simulink model "PD_trajectory"  (R2020b)
settings: Solver=VariableStepAuto  StartTime=0.0  StopTime=10  RelTol=1e-3
libraries: pid_lib x6
(part 2 of 3)

== matlab function PD_trajectory/plant/MATLAB Function1 ==
  data: Theta input size=6; V output size=6; Thetad input size=6
function V = NumV(Theta,Thetad)
t1=Theta(1);
t2=Theta(2);
t3=Theta(3);
t4=Theta(4);
t5=Theta(5);
t6=Theta(6);
td1=Thetad(1);
td2=Thetad(2);
td3=Thetad(3);
td4=Thetad(4);
td5=Thetad(5);
td6=Thetad(6);

L1=0.1025;
L2=0.408;
L3=0.376;
L4=0.1025; 
L5=0.1025;

V=[td2*(td1*(25109.9375*sin(2.0*t2 + 2.0*t3 + 2.0*t4) + 1339251.84*sin(2.0*t2 + t3) + 184221.2*sin(2.0*t2 + 2.0*t3 + t4) + 1047890.8266888983333333366584905*sin(2.0*t2) + 199899.6*sin(2.0*t2 + t3 + t4) + 617106.24*sin(2.0*t2 + 2.0*t3) - 0.149375*L3^2*sin(2.0*t2 + 2.0*t3 + 2.0*t4) + 1.195*L4^2*sin(2.0*t2 + 2.0*t3 + 2.0*t4) - 898.64*L4*sin(2.0*t2 +2.0*t3 + t4) + 0.0746875*L3^2*sin(2.0*t2 + 2.0*t3 + 2.0*t4 - 2.0*t5) + 0.0746875*L3^2*sin(2.0*t2 + 2.0*t3 + 2.0*t4 + 2.0*t5) + 224.66*L3*sin(2.0*t2 + 2.0*t3 + t4 - 1.0*t5) -61.24375*L3*sin(2.0*t2 + 2.0*t3 + 2.0*t4 + t5) - 975.12*L4*sin(2.0*t2 + t3 + t4) + 243.78*L3*sin(2.0*t2 + t3 + t4 - 1.0*t5) - 224.66*L3*sin(2.0*t2 + 2.0*t3 + t4 + t5) +0.94625*L2^2*sin(2.0*t2) - 244.975*L4*sin(2.0*t2 + 2.0*t3 + 2.0*t4) + 61.24375*L3*sin(2.0*t2 + 2.0*t3 + 2.0*t4 - 1.0*t5) - 243.78*L3*sin(2.0*t2 + t3 + t4 + t5) -0.5975*L3*L4*sin(2.0*t2 + 2.0*t3 + 2.0*t4 - 1.0*t5) + 0.5975*L3*L4*sin(2.0*t2 + 2.0*t3 + 2.0*t4 + t5)) - 1.0*td5*(0.00036659114583333335217474324707609*sin(3.0*t2 -1.0*t1 + t3 + t4) + 0.00073318229166666670434948649415219*sin(t2 - 2.0*t1 + 3.0*t3 + t4) + 0.00018329557291666667608737162353805*sin(3.0*t2 - 2.0*t1 + t3 + t4) +0.00018329557291666667608737162353805*sin(2.0*t1 + 3.0*t2 + t3 + t4) + 0.00073318229166666670434948649415219*sin(t2 + t3 + t4) + 0.00036659114583333335217474324707609*sin(t1 - 1.0*t2 + t3 + t4) -0.00057664973958333336527190549070099*sin(t2 - 2.0*t1 + t3 + t4) - 0.00057664973958333336527190549070099*sin(2.0*t1 + t2 + t3 + t4) + 0.00036659114583333335217474324707609*sin(t1 + 3.0*t2 + t3 + t4) -0.00018329557291666667608737162353805*sin(2.0*t1 + t2 - 1.0*t3 - 1.0*t4) + 0.00036659114583333335217474324707609*sin(t3 - 1.0*t2 + t4) - 0.00036659114583333335217474324707609*sin(t1 + t2 - 1.0*t3 - 1.0*t4) +0.00073318229166666670434948649415219*sin(2.0*t1 + t2 - 1.0*t3 + t4) + 0.00018329557291666667608737162353805*sin(2.0*t1 - 1.0*t2 + t3 + t4) - 0.0010997734375000000565242297412283*sin(3.0*t2 + t3 + t4) -243.78*L3*sin(t2 - 1.0*t5) + 0.29875*L3^2*sin(t2 + t3 + t4) - 0.149375*L3^2*sin(t2 + t3 + t4 - 2.0*t5) - 0.149375*L3^2*sin(t2 + t3 + t4 + 2.0*t5) + 61.24375*L3*sin(t2 + t3 + t4 + t5) + 243.78*L3*sin(t2 + t5) -224.66*L3*sin(t2 + t3 - 1.0*t5) + 224.66*L3*sin(t2 + t3 + t5) - 61.24375*L3*sin(t2 + t3 + t4 - 1.0*t5) + 0.5975*L3*L4*sin(t2 + t3 + t4 - 1.0*t5) - 0.5975*L3*L4*sin(t2 + t3 + t4 + t5)) -1.0*td6*(0.00084023437500000005238864897449957*cos(t1)*cos(t5)*sin(t1) + 0.00042011718750000002619432448724979*cos(t1)^2*cos(t2)*cos(t3)*cos(t4)*sin(t5) - 0.00042011718750000002619432448724979*cos(t2)*cos(t3)*cos(t4)*sin(t1)^2*sin(t5) -0.00042011718750000002619432448724979*cos(t1)^2*cos(t2)*sin(t3)*sin(t4)*sin(t5) - 0.00042011718750000002619432448724979*cos(t1)^2*cos(t3)*sin(t2)*sin(t4)*sin(t5) - 0.00042011718750000002619432448724979*cos(t1)^2*cos(t4)*sin(t2)*sin(t3)*sin(t5) +0.00042011718750000002619432448724979*cos(t2)*sin(t1)^2*sin(t3)*sin(t4)*sin(t5) + 0.00042011718750000002619432448724979*cos(t3)*sin(t1)^2*sin(t2)*sin(t4)*sin(t5) + 0.00042011718750000002619432448724979*cos(t4)*sin(t1)^2*sin(t2)*sin(t3)*sin(t5)) +td2*(1.8925*L2^2*cos(t1)*cos(t2)^2*sin(t1) - 1.8925*L2^2*cos(t1)*sin(t1) - 531.7925*sin(t2)*L2*cos(t1)^2 + 531.7925*sin(t2)*L2*sin(t1)^2 - 0.0029327291666666668173979459766088*sin(t3)*cos(t1)^2*cos(t3) - 0.10662220333333332668301896006824*cos(t1)*cos(t2)^2*sin(t1) +0.0058654583333333336347958919532175*cos(t1)*cos(t3)^2*sin(t1) + 149433.79717526104166665983606632*cos(t1)*sin(t1) + 0.0029327291666666668173979459766088*sin(t3)*cos(t3)*sin(t1)^2) + td3*(- 0.0029327291666666668173979459766088*sin(t3)*cos(t1)^2*cos(t3) + 0.0029327291666666668173979459766088*cos(t1)*cos(t2)^2*sin(t1) + 0.0058654583333333336347958919532175*cos(t1)*cos(t3)^2*sin(t1) - 0.0048796714583333336643505839802515*cos(t1)*sin(t1) + 0.0029327291666666668173979459766088*sin(t3)*cos(t3)*sin(t1)^2 + 0.00073318229166666670434948649415219*sin(t1 - 2.0*t2) + 0.00073318229166666670434948649415219*sin(t1 + 2.0*t2)) + td4*(0.0029327291666666668173979459766088*sin(2.0*t1)*cos(t3)^2 - 0.0029327291666666668173979459766088*cos(2.0*t1)*sin(t3)*cos(t3) + 0.00073318229166666670434948649415219*sin(t1 - 2.0*t2) + 0.00073318229166666670434948649415219*sin(t1 + 2.0*t2) - 0.0026196640625000001392427839697064*sin(2.0*t1) + 0.00073318229166666670434948649415219*cos(2.0*t2)*sin(2.0*t1))) - td6*(td6*(0.5*(0.00084023437500000005238864897449957*cos(t1)*cos(t5) - 0.00084023437500000005238864897449957*cos(t2)*cos(t3)*cos(t4)*sin(t1)*sin(t5) + 0.00084023437500000005238864897449957*cos(t2)*sin(t1)*sin(t3)*sin(t4)*sin(t5) + 0.00084023437500000005238864897449957*cos(t3)*sin(t1)*sin(t2)*sin(t4)*sin(t5) + 0.00084023437500000005238864897449957*cos(t4)*sin(t1)*sin(t2)*sin(t3)*sin(t5))*(cos(t1)*cos(t2)*sin(t3)*sin(t4)*sin(t5) - 1.0*cos(t1)*cos(t2)*cos(t3)*cos(t4)*sin(t5) - 1.0*cos(t5)*sin(t1) + cos(t1)*cos(t3)*sin(t2)*sin(t4)*sin(t5) + cos(t1)*cos(t4)*sin(t2)*sin(t3)*sin(t5)) - 0.5*(0.0016804687500000001047772979489991*cos(t1)*cos(t5) - 0.0016804687500000001047772979489991*cos(t2)*cos(t3)*cos(t4)*sin(t1)*sin(t5) + 0.0016804687500000001047772979489991*cos(t2)*sin(t1)*sin(t3)*sin(t4)*sin(t5) + 0.0016804687500000001047772979489991*cos(t3)*sin(t1)*sin(t2)*sin(t4)*sin(t5) + 0.0016804687500000001047772979489991*cos(t4)*sin(t1)*sin(t2)*sin(t3)*sin(t5))*(cos(t1)*cos(t2)*sin(t3)*sin(t4)*sin(t5) - 1.0*cos(t1)*cos(t2)*cos(t3)*cos(t4)*sin(t5) - 1.0*cos(t5)*sin(t1) + cos(t1)*cos(t3)*sin(t2)*sin(t4)*sin(t5) + cos(t1)*cos(t4)*sin(t2)*sin(t3)*sin(t5)) + 0.5*(0.00084023437500000005238864897449957*cos(t1)*cos(t2)*sin(t3)*sin(t4)*sin(t5) - 0.00084023437500000005238864897449957*cos(t1)*cos(t2)*cos(t3)*cos(t4)*sin(t5) - 0.00084023437500000005238864897449957*cos(t5)*sin(t1) + 0.00084023437500000005238864897449957*cos(t1)*cos(t3)*sin(t2)*sin(t4)*sin(t5) + 0.00084023437500000005238864897449957*cos(t1)*cos(t4)*sin(t2)*sin(t3)*sin(t5))*(cos(t1)*cos(t5) - 1.0*cos(t2)*cos(t3)*cos(t4)*sin(t1)*sin(t5) + cos(t2)*sin(t1)*sin(t3)*sin(t4)*sin(t5) + cos(t3)*sin(t1)*sin(t2)*sin(t4)*sin(t5) + cos(t4)*sin(t1)*sin(t2)*sin(t3)*sin(t5)) - 0.5*(0.0016804687500000001047772979489991*cos(t1)*cos(t2)*sin(t3)*sin(t4)*sin(t5) - 0.0016804687500000001047772979489991*cos(t1)*cos(t2)*cos(t3)*cos(t4)*sin(t5) - 0.0016804687500000001047772979489991*cos(t5)*sin(t1) + 0.0016804687500000001047772979489991*cos(t1)*cos(t3)*sin(t2)*sin(t4)*sin(t5) + 0.0016804687500000001047772979489991*cos(t1)*cos(t4)*sin(t2)*sin(t3)*sin(t5))*(cos(t1)*cos(t5) - 1.0*cos(t2)*cos(t3)*cos(t4)*sin(t1)*sin(t5) + cos(t2)*sin(t1)*sin(t3)*sin(t4)*sin(t5) + cos(t3)*sin(t1)*sin(t2)*sin(t4)*sin(t5) + cos(t4)*sin(t1)*sin(t2)*sin(t3)*sin(t5))) + 1.0*td2*(0.00084023437500000005238864897449957*cos(t1)*cos(t5)*sin(t1) + 0.00042011718750000002619432448724979*cos(t1)^2*cos(t2)*cos(t3)*cos(t4)*sin(t5) - 0.00042011718750000002619432448724979*cos(t2)*cos(t3)*cos(t4)*sin(t1)^2*sin(t5) - 0.00042011718750000002619432448724979*cos(t1)^2*cos(t2)*sin(t3)*sin(t4)*sin(t5) - 0.00042011718750000002619432448724979*cos(t1)^2*cos(t3)*sin(t2)*sin(t4)*sin(t5) - 0.00042011718750000002619432448724979*cos(t1)^2*cos(t4)*sin(t2)*sin(t3)*sin(t5) + 0.00042011718750000002619432448724979*cos(t2)*sin(t1)^2*sin(t3)*sin(t4)*sin(t5) + 0.00042011718750000002619432448724979*cos(t3)*sin(t1)^2*sin(t2)*sin(t4)*sin(t5) + 0.00042011718750000002619432448724979*cos(t4)*sin(t1)^2*sin(t2)*sin(t3)*sin(t5)) + 1.0*td3*(0.00084023437500000005238864897449957*cos(t1)*cos(t5)*sin(t1) + 0.00042011718750000002619432448724979*cos(t1)^2*cos(t2)*cos(t3)*cos(t4)*sin(t5) - 0.00042011718750000002619432448724979*cos(t2)*cos(t3)*cos(t4)*sin(t1)^2*sin(t5) - 0.00042011718750000002619432448724979*cos(t1)^2*cos(t2)*sin(t3)*sin(t4)*sin(t5) - 0.00042011718750000002619432448724979*cos(t1)^2*cos(t3)*sin(t2)*sin(t4)*sin(t5) - 0.00042011718750000002619432448724979*cos(t1)^2*cos(t4)*sin(t2)*sin(t3)*sin(t5) + 0.00042011718750000002619432448724979*cos(t2)*sin(t1)^2*sin(t3)*sin(t4)*sin(t5) + 0.00042011718750000002619432448724979*cos(t3)*sin(t1)^2*sin(t2)*sin(t4)*sin(t5) + 0.00042011718750000002619432448724979*cos(t4)*sin(t1)^2*sin(t2)*sin(t3)*sin(t5)) + 1.0*td4*(0.00084023437500000005238864897449957*cos(t1)*cos(t5)*sin(t1) + 0.00042011718750000002619432448724979*cos(t1)^2*cos(t2)*cos(t3)*cos(t4)*sin(t5) - 0.00042011718750000002619432448724979*cos(t2)*cos(t3)*cos(t4)*sin(t1)^2*sin(t5) - 0.00042011718750000002619432448724979*cos(t1)^2*cos(t2)*sin(t3)*sin(t4)*sin(t5) - 0.00042011718750000002619432448724979*cos(t1)^2*cos(t3)*sin(t2)*sin(t4)*sin(t5) - 0.00042011718750000002619432448724979*cos(t1)^2*cos(t4)*sin(t2)*sin(t3)*sin(t5) + 0.00042011718750000002619432448724979*cos(t2)*sin(t1)^2*sin(t3)*sin(t4)*sin(t5) + 0.00042011718750000002619432448724979*cos(t3)*sin(t1)^2*sin(t2)*sin(t4)*sin(t5) + 0.00042011718750000002619432448724979*cos(t4)*sin(t1)^2*sin(t2)*sin(t3)*sin(t5)) + td5*(0.00021005859375000001309716224362489*cos(2.0*t2)*cos(2.0*t3)*sin(2.0*t1)*sin(2.0*t4)*sin(t5) + 0.00021005859375000001309716224362489*cos(2.0*t2)*cos(2.0*t4)*sin(2.0*t1)*sin(2.0*t3)*sin(t5) + 0.00021005859375000001309716224362489*cos(2.0*t3)*cos(2.0*t4)*sin(2.0*t1)*sin(2.0*t2)*sin(t5) - 0.00042011718750000002619432448724979*cos(2.0*t1)*cos(t2)*cos(t3)*cos(t5)*sin(t4) - 0.00042011718750000002619432448724979*cos(2.0*t1)*cos(t2)*cos(t4)*cos(t5)*sin(t3) - 0.00042011718750000002619432448724979*cos(2.0*t1)*cos(t3)*cos(t4)*cos(t5)*sin(t2) - 0.00021005859375000001309716224362489*sin(2.0*t1)*sin(2.0*t2)*sin(2.0*t3)*sin(2.0*t4)*sin(t5) + 0.00042011718750000002619432448724979*cos(2.0*t1)*cos(t5)*sin(t2)*sin(t3)*sin(t4))) - td3*(1.0*td6*(0.00084023437500000005238864897449957*cos(t1)*cos(t5)*sin(t1) + 0.00042011718750000002619432448724979*cos(t1)^2*cos(t2)*cos(t3)*cos(t4)*sin(t5) - 0.00042011718750000002619432448724979*cos(t2)*cos(t3)*cos(t4)*sin(t1)^2*sin(t5) - 0.00042011718750000002619432448724979*cos(t1)^2*cos(t2)*sin(t3)*sin(t4)*sin(t5) - 0.00042011718750000002619432448724979*cos(t1)^2*cos(t3)*sin(t2)*sin(t4)*sin(t5) - 0.00042011718750000002619432448724979*cos(t1)^2*cos(t4)*sin(t2)*sin(t3)*sin(t5) + 0.00042011718750000002619432448724979*cos(t2)*sin(t1)^2*sin(t3)*sin(t4)*sin(t5) + 0.00042011718750000002619432448724979*cos(t3)*sin(t1)^2*sin(t2)*sin(t4)*sin(t5) + 0.00042011718750000002619432448724979*cos(t4)*sin(t1)^2*sin(t2)*sin(t3)*sin(t5)) - td1*(25109.9375*sin(2.0*t2 + 2.0*t3 + 2.0*t4) + 669625.92*sin(2.0*t2 + t3) + 184221.2*sin(2.0*t2 + 2.0*t3 + t4) - 99949.8*sin(t3 + t4) + 99949.8*sin(2.0*t2 + t3 + t4) - 669625.92*sin(t3) + 617106.24*sin(2.0*t2 + 2.0*t3) - 0.149375*L3^2*sin(2.0*t2 + 2.0*t3 + 2.0*t4) + 1.195*L4^2*sin(2.0*t2 + 2.0*t3 + 2.0*t4) - 898.64*L4*sin(2.0*t2 + 2.0*t3 + t4) + 0.0746875*L3^2*sin(2.0*t2 + 2.0*t3 + 2.0*t4 - 2.0*t5) + 0.0746875*L3^2*sin(2.0*t2 + 2.0*t3 + 2.0*t4 + 2.0*t5) + 224.66*L3*sin(2.0*t2 + 2.0*t3 + t4 - 1.0*t5) - 61.24375*L3*sin(2.0*t2 + 2.0*t3 + 2.0*t4 + t5) + 487.56*L4*sin(t3 + t4) - 487.56*L4*sin(2.0*t2 + t3 + t4) - 121.89*L3*sin(t3 + t4 - 1.0*t5) + 121.89*L3*sin(2.0*t2 + t3 + t4 - 1.0*t5) - 224.66*L3*sin(2.0*t2 + 2.0*t3 + t4 + t5) - 244.975*L4*sin(2.0*t2 + 2.0*t3 + 2.0*t4) + 61.24375*L3*sin(2.0*t2 + 2.0*t3 + 2.0*t4 - 1.0*t5) + 121.89*L3*sin(t3 + t4 + t5) - 121.89*L3*sin(2.0*t2 + t3 + t4 + t5) - 0.5975*L3*L4*sin(2.0*t2 + 2.0*t3 + 2.0*t4 - 1.0*t5) + 0.5975*L3*L4*sin(2.0*t2 + 2.0*t3 + 2.0*t4 + t5)) - td3*(- 0.0029327291666666668173979459766088*sin(t3)*cos(t1)^2*cos(t3) + 0.0029327291666666668173979459766088*cos(t1)*cos(t2)^2*sin(t1) + 0.0058654583333333336347958919532175*cos(t1)*cos(t3)^2*sin(t1) - 0.0048796714583333336643505839802515*cos(t1)*sin(t1) + 0.0029327291666666668173979459766088*sin(t3)*cos(t3)*sin(t1)^2) + td5*(0.00073318229166666670434948649415219*sin(t2 - 2.0*t1 + 3.0*t3 + t4) + 0.00018329557291666667608737162353805*sin(3.0*t2 - 2.0*t1 + t3 + t4) + 0.00018329557291666667608737162353805*sin(2.0*t1 + 3.0*t2 + t3 + t4) + 0.00073318229166666670434948649415219*sin(t2 + t3 + t4) - 0.00057664973958333336527190549070099*sin(t2 - 2.0*t1 + t3 + t4) - 0.00057664973958333336527190549070099*sin(2.0*t1 + t2 + t3 + t4) - 0.00018329557291666667608737162353805*sin(2.0*t1 + t2 - 1.0*t3 - 1.0*t4) - 0.00036659114583333335217474324707609*sin(t3 - 1.0*t2 + t4) + 0.00073318229166666670434948649415219*sin(2.0*t1 + t2 - 1.0*t3 + t4) + 0.00018329557291666667608737162353805*sin(2.0*t1 - 1.0*t2 + t3 + t4) - 0.00036659114583333335217474324707609*sin(3.0*t2 + t3 + t4) + 0.29875*L3^2*sin(t2 + t3 + t4) - 0.149375*L3^2*sin(t2 + t3 + t4 - 2.0*t5) - 0.149375*L3^2*sin(t2 + t3 + t4 + 2.0*t5) + 61.24375*L3*sin(t2 + t3 + t4 + t5) - 224.66*L3*sin(t2 + t3 - 1.0*t5) + 224.66*L3*sin(t2 + t3 + t5) - 61.24375*L3*sin(t2 + t3 + t4 - 1.0*t5) + 0.5975*L3*L4*sin(t2 + t3 + t4 - 1.0*t5) - 0.5975*L3*L4*sin(t2 + t3 + t4 + t5)) - td4*(- 0.0029327291666666668173979459766088*sin(t3)*cos(t1)^2*cos(t3) + 0.0029327291666666668173979459766088*cos(t1)*cos(t2)^2*sin(t1) + 0.0058654583333333336347958919532175*cos(t1)*cos(t3)^2*sin(t1) - 0.0067056927083333336871845409277171*cos(t1)*sin(t1) + 0.0029327291666666668173979459766088*sin(t3)*cos(t3)*sin(t1)^2) + 1.0*td2*(0.0029327291666666668173979459766088*sin(t3)*cos(t1)^2*cos(t3) - 0.0029327291666666668173979459766088*cos(t1)*cos(t2)^2*sin(t1) - 0.0058654583333333336347958919532175*cos(t1)*cos(t3)^2*sin(t1) + 0.0048796714583333336643505839802515*cos(t1)*sin(t1) - 0.0029327291666666668173979459766088*sin(t3)*cos(t3)*sin(t1)^2 + 0.00073318229166666670434948649415219*sin(t1 - 2.0*t2) + 0.00073318229166666670434948649415219*sin(t1 + 2.0*t2))) - td4*(1.0*td6*(0.00084023437500000005238864897449957*cos(t1)*cos(t5)*sin(t1) + 0.00042011718750000002619432448724979*cos(t1)^2*cos(t2)*cos(t3)*cos(t4)*sin(t5) - 0.00042011718750000002619432448724979*cos(t2)*cos(t3)*cos(t4)*sin(t1)^2*sin(t5) - 0.00042011718750000002619432448724979*cos(t1)^2*cos(t2)*sin(t3)*sin(t4)*sin(t5) - 0.00042011718750000002619432448724979*cos(t1)^2*cos(t3)*sin(t2)*sin(t4)*sin(t5) - 0.00042011718750000002619432448724979*cos(t1)^2*cos(t4)*sin(t2)*sin(t3)*sin(t5) + 0.00042011718750000002619432448724979*cos(t2)*sin(t1)^2*sin(t3)*sin(t4)*sin(t5) + 0.00042011718750000002619432448724979*cos(t3)*sin(t1)^2*sin(t2)*sin(t4)*sin(t5) + 0.00042011718750000002619432448724979*cos(t4)*sin(t1)^2*sin(t2)*sin(t3)*sin(t5)) + td5*(0.00073318229166666670434948649415219*sin(t2 - 2.0*t1 + 3.0*t3 + t4) + 0.00018329557291666667608737162353805*sin(3.0*t2 - 2.0*t1 + t3 + t4) + 0.00018329557291666667608737162353805*sin(2.0*t1 + 3.0*t2 + t3 + t4) + 0.00073318229166666670434948649415219*sin(t2 + t3 + t4) - 0.00057664973958333336527190549070099*sin(t2 - 2.0*t1 + t3 + t4) - 0.00057664973958333336527190549070099*sin(2.0*t1 + t2 + t3 + t4) - 0.00018329557291666667608737162353805*sin(2.0*t1 + t2 - 1.0*t3 - 1.0*t4) - 0.00036659114583333335217474324707609*sin(t3 - 1.0*t2 + t4) + 0.00073318229166666670434948649415219*sin(2.0*t1 + t2 - 1.0*t3 + t4) + 0.00018329557291666667608737162353805*sin(2.0*t1 - 1.0*t2 + t3 + t4) - 0.00036659114583333335217474324707609*sin(3.0*t2 + t3 + t4) + 0.29875*L3^2*sin(t2 + t3 + t4) - 0.149375*L3^2*sin(t2 + t3 + t4 - 2.0*t5) - 0.149375*L3^2*sin(t2 + t3 + t4 + 2.0*t5) + 61.24375*L3*sin(t2 + t3 + t4 + t5) - 61.24375*L3*sin(t2 + t3 + t4 - 1.0*t5) + 0.5975*L3*L4*sin(t2 + t3 + t4 - 1.0*t5) - 0.5975*L3*L4*sin(t2 + t3 + t4 + t5)) + 1.0*td4*(0.001153299479166666730543810981402*sin(2.0*t1) - 0.00073318229166666670434948649415219*cos(2.0*t2)*sin(2.0*t1) + 0.0014663645833333334086989729883044*cos(2.0*t1)*sin(2.0*t3) - 0.0014663645833333334086989729883044*cos(2.0*t3)*sin(2.0*t1)) - td3*(- 0.0029327291666666668173979459766088*sin(t3)*cos(t1)^2*cos(t3) + 0.0029327291666666668173979459766088*cos(t1)*cos(t2)^2*sin(t1) + 0.0058654583333333336347958919532175*cos(t1)*cos(t3)^2*sin(t1) - 0.0067056927083333336871845409277171*cos(t1)*sin(t1) + 0.0029327291666666668173979459766088*sin(t3)*cos(t3)*sin(t1)^2) + 1.0*td2*(- 0.0029327291666666668173979459766088*sin(2.0*t1)*cos(t3)^2 + 0.0029327291666666668173979459766088*cos(2.0*t1)*sin(t3)*cos(t3) + 0.00073318229166666670434948649415219*sin(t1 - 2.0*t2) + 0.00073318229166666670434948649415219*sin(t1 + 2.0*t2) + 0.0026196640625000001392427839697064*sin(2.0*t1) - 0.00073318229166666670434948649415219*cos(2.0*t2)*sin(2.0*t1)) - td1*(25109.9375*sin(2.0*t2 + 2.0*t3 + 2.0*t4) + 92110.6*sin(2.0*t2 + 2.0*t3 + t4) - 99949.8*sin(t3 + t4) + 99949.8*sin(2.0*t2 + t3 + t4) - 92110.6*sin(t4) - 112.33*L3*sin(t4 - 1.0*t5) - 0.149375*L3^2*sin(2.0*t2 + 2.0*t3 + 2.0*t4) + 1.195*L4^2*sin(2.0*t2 + 2.0*t3 + 2.0*t4) - 449.32*L4*sin(2.0*t2 + 2.0*t3 + t4) + 0.0746875*L3^2*sin(2.0*t2 + 2.0*t3 + 2.0*t4 - 2.0*t5) + 0.0746875*L3^2*sin(2.0*t2 + 2.0*t3 + 2.0*t4 + 2.0*t5) + 112.33*L3*sin(2.0*t2 + 2.0*t3 + t4 - 1.0*t5) - 61.24375*L3*sin(2.0*t2 + 2.0*t3 + 2.0*t4 + t5) + 487.56*L4*sin(t3 + t4) + 112.33*L3*sin(t4 + t5) - 487.56*L4*sin(2.0*t2 + t3 + t4) - 121.89*L3*sin(t3 + t4 - 1.0*t5) + 121.89*L3*sin(2.0*t2 + t3 + t4 - 1.0*t5) - 112.33*L3*sin(2.0*t2 + 2.0*t3 + t4 + t5) + 449.32*L4*sin(t4) - 244.975*L4*sin(2.0*t2 + 2.0*t3 + 2.0*t4) + 61.24375*L3*sin(2.0*t2 + 2.0*t3 + 2.0*t4 - 1.0*t5) + 121.89*L3*sin(t3 + t4 + t5) - 121.89*L3*sin(2.0*t2 + t3 + t4 + t5) - 0.5975*L3*L4*sin(2.0*t2 + 2.0*t3 + 2.0*t4 - 1.0*t5) + 0.5975*L3*L4*sin(2.0*t2 + 2.0*t3 + 2.0*t4 + t5))) - td5*(1.0*td3*(0.00073318229166666670434948649415219*sin(t2 - 2.0*t1 + 3.0*t3 + t4) - 0.00036659114583333335217474324707609*sin(3.0*t2 - 1.0*t1 + t3 + t4) + 0.00018329557291666667608737162353805*sin(3.0*t2 - 2.0*t1 + t3 + t4) + 0.00018329557291666667608737162353805*sin(2.0*t1 + 3.0*t2 + t3 + t4) - 0.00073318229166666670434948649415219*sin(t2 + t3 + t4) + 0.00036659114583333335217474324707609*sin(t1 - 1.0*t2 + t3 + t4) - 0.00057664973958333336527190549070099*sin(t2 - 2.0*t1 + t3 + t4) - 0.00057664973958333336527190549070099*sin(2.0*t1 + t2 + t3 + t4) - 0.00036659114583333335217474324707609*sin(t1 + 3.0*t2 + t3 + t4) - 0.00018329557291666667608737162353805*sin(2.0*t1 + t2 - 1.0*t3 - 1.0*t4) + 0.00036659114583333335217474324707609*sin(t3 - 1.0*t2 + t4) - 0.00036659114583333335217474324707609*sin(t1 + t2 - 1.0*t3 - 1.0*t4) + 0.00073318229166666670434948649415219*sin(2.0*t1 + t2 - 1.0*t3 + t4) + 0.00018329557291666667608737162353805*sin(2.0*t1 - 1.0*t2 + t3 + t4) + 0.00036659114583333335217474324707609*sin(3.0*t2 + t3 + t4) - 0.29875*L3^2*sin(t2 + t3 + t4) + 0.149375*L3^2*sin(t2 + t3 + t4 - 2.0*t5) + 0.149375*L3^2*sin(t2 + t3 + t4 + 2.0*t5) - 61.24375*L3*sin(t2 + t3 + t4 + t5) + 224.66*L3*sin(t2 + t3 - 1.0*t5) - 224.66*L3*sin(t2 + t3 + t5) + 61.24375*L3*sin(t2 + t3 + t4 - 1.0*t5) - 0.5975*L3*L4*sin(t2 + t3 + t4 - 1.0*t5) + 0.5975*L3*L4*sin(t2 + t3 + t4 + t5)) + 1.0*td5*(0.00018329557291666667608737162353805*sin(2.0*t3 - 1.0*t1 + 2.0*t4) - 0.00036659114583333335217474324707609*sin(2.0*t1 + 2.0*t2 + 2.0*t4) + 0.000091647786458333338043685811769024*sin(2.0*t3 - 2.0*t1 + 2.0*t4) - 0.000091647786458333338043685811769024*sin(2.0*t1 + 2.0*t3 + 2.0*t4) - 0.00018329557291666667608737162353805*sin(4.0*t2 - 1.0*t1 + 2.0*t3 + 2.0*t4) - 0.00028832486979166668263595274535049*sin(2.0*t2 - 2.0*t1 + 2.0*t3 + 2.0*t4) + 0.00028832486979166668263595274535049*sin(2.0*t1 + 2.0*t2 + 2.0*t3 + 2.0*t4) + 0.00036659114583333335217474324707609*sin(2.0*t2 - 2.0*t1 + 4.0*t3 + 2.0*t4) + 0.000091647786458333338043685811769024*sin(4.0*t2 - 2.0*t1 + 2.0*t3 + 2.0*t4) - 0.000091647786458333338043685811769024*sin(2.0*t1 + 4.0*t2 + 2.0*t3 + 2.0*t4) - 0.00018329557291666667608737162353805*sin(t1 + 2.0*t3 + 2.0*t4) + 0.00018329557291666667608737162353805*sin(t1 + 4.0*t2 + 2.0*t3 + 2.0*t4) - 0.00057664973958333336527190549070099*sin(2.0*t1) + 0.00018329557291666667608737162353805*sin(2.0*t1 - 2.0*t2) + 0.00018329557291666667608737162353805*sin(2.0*t1 + 2.0*t2) + 0.00073318229166666670434948649415219*sin(2.0*t1 - 2.0*t3)) + 1.0*td1*(0.0746875*L3^2*sin(2.0*t2 + 2.0*t3 + 2.0*t4 - 2.0*t5) - 112.33*L3*sin(t4 - 1.0*t5) - 0.0746875*L3^2*sin(2.0*t2 + 2.0*t3 + 2.0*t4 + 2.0*t5) + 112.33*L3*sin(2.0*t2 + 2.0*t3 + t4 - 1.0*t5) + 30.621875*L3*sin(2.0*t2 + 2.0*t3 + 2.0*t4 + t5) - 112.33*L3*sin(t4 + t5) - 121.89*L3*sin(t3 + t4 - 1.0*t5) + 121.89*L3*sin(2.0*t2 + t3 + t4 - 1.0*t5) + 112.33*L3*sin(2.0*t2 + 2.0*t3 + t4 + t5) + 0.149375*L3^2*sin(2.0*t5) + 167.8975*L3*sin(t5) + 30.621875*L3*sin(2.0*t2 + 2.0*t3 + 2.0*t4 - 1.0*t5) - 121.89*L3*sin(t3 + t4 + t5) + 121.89*L3*sin(2.0*t2 + t3 + t4 + t5) - 0.29875*L3*L4*sin(2.0*t2 + 2.0*t3 + 2.0*t4 - 1.0*t5) - 0.29875*L3*L4*sin(2.0*t2 + 2.0*t3 + 2.0*t4 + t5)) - td2*(0.00073318229166666670434948649415219*sin(3.0*t2 - 1.0*t1 + t3 + t4) - 0.00073318229166666670434948649415219*sin(t2 - 2.0*t1 + 3.0*t3 + t4) - 0.00018329557291666667608737162353805*sin(3.0*t2 - 2.0*t1 + t3 + t4) - 0.00018329557291666667608737162353805*sin(2.0*t1 + 3.0*t2 + t3 + t4) + 0.00073318229166666670434948649415219*sin(t2 + t3 + t4) + 0.00057664973958333336527190549070099*sin(t2 - 2.0*t1 + t3 + t4) + 0.00057664973958333336527190549070099*sin(2.0*t1 + t2 + t3 + t4) + 0.00073318229166666670434948649415219*sin(t1 + 3.0*t2 + t3 + t4) + 0.00018329557291666667608737162353805*sin(2.0*t1 + t2 - 1.0*t3 - 1.0*t4) + 0.00036659114583333335217474324707609*sin(t3 - 1.0*t2 + t4) - 0.00073318229166666670434948649415219*sin(2.0*t1 + t2 - 1.0*t3 + t4) - 0.00018329557291666667608737162353805*sin(2.0*t1 - 1.0*t2 + t3 + t4) - 0.0010997734375000000565242297412283*sin(3.0*t2 + t3 + t4) - 243.78*L3*sin(t2 - 1.0*t5) + 0.29875*L3^2*sin(t2 + t3 + t4) - 0.149375*L3^2*sin(t2 + t3 + t4 - 2.0*t5) - 0.149375*L3^2*sin(t2 + t3 + t4 + 2.0*t5) + 61.24375*L3*sin(t2 + t3 + t4 + t5) + 243.78*L3*sin(t2 + t5) - 224.66*L3*sin(t2 + t3 - 1.0*t5) + 224.66*L3*sin(t2 + t3 + t5) - 61.24375*L3*sin(t2 + t3 + t4 - 1.0*t5) + 0.5975*L3*L4*sin(t2 + t3 + t4 - 1.0*t5) - 0.5975*L3*L4*sin(t2 + t3 + t4 + t5)) + 1.0*td4*(0.00073318229166666670434948649415219*sin(t2 - 2.0*t1 + 3.0*t3 + t4) - 0.00036659114583333335217474324707609*sin(3.0*t2 - 1.0*t1 + t3 + t4) + 0.00018329557291666667608737162353805*sin(3.0*t2 - 2.0*t1 + t3 + t4) + 0.00018329557291666667608737162353805*sin(2.0*t1 + 3.0*t2 + t3 + t4) - 0.00073318229166666670434948649415219*sin(t2 + t3 + t4) + 0.00036659114583333335217474324707609*sin(t1 - 1.0*t2 + t3 + t4) - 0.00057664973958333336527190549070099*sin(t2 - 2.0*t1 + t3 + t4) - 0.00057664973958333336527190549070099*sin(2.0*t1 + t2 + t3 + t4) - 0.00036659114583333335217474324707609*sin(t1 + 3.0*t2 + t3 + t4) - 0.00018329557291666667608737162353805*sin(2.0*t1 + t2 - 1.0*t3 - 1.0*t4) + 0.00036659114583333335217474324707609*sin(t3 - 1.0*t2 + t4) - 0.00036659114583333335217474324707609*sin(t1 + t2 - 1.0*t3 - 1.0*t4) + 0.00073318229166666670434948649415219*sin(2.0*t1 + t2 - 1.0*t3 + t4) + 0.00018329557291666667608737162353805*sin(2.0*t1 - 1.0*t2 + t3 + t4) + 0.00036659114583333335217474324707609*sin(3.0*t2 + t3 + t4) - 0.29875*L3^2*sin(t2 + t3 + t4) + 0.149375*L3^2*sin(t2 + t3 + t4 - 2.0*t5) + 0.149375*L3^2*sin(t2 + t3 + t4 + 2.0*t5) - 61.24375*L3*sin(t2 + t3 + t4 + t5) + 61.24375*L3*sin(t2 + t3 + t4 - 1.0*t5) - 0.5975*L3*L4*sin(t2 + t3 + t4 - 1.0*t5) + 0.5975*L3*L4*sin(t2 + t3 + t4 + t5)) + td6*(0.00021005859375000001309716224362489*cos(2.0*t2)*cos(2.0*t3)*sin(2.0*t1)*sin(2.0*t4)*sin(t5) + 0.00021005859375000001309716224362489*cos(2.0*t2)*cos(2.0*t4)*sin(2.0*t1)*sin(2.0*t3)*sin(t5) + 0.00021005859375000001309716224362489*cos(2.0*t3)*cos(2.0*t4)*sin(2.0*t1)*sin(2.0*t2)*sin(t5) - 0.00042011718750000002619432448724979*cos(2.0*t1)*cos(t2)*cos(t3)*cos(t5)*sin(t4) - 0.00042011718750000002619432448724979*cos(2.0*t1)*cos(t2)*cos(t4)*cos(t5)*sin(t3) - 0.00042011718750000002619432448724979*cos(2.0*t1)*cos(t3)*cos(t4)*cos(t5)*sin(t2) - 0.00021005859375000001309716224362489*sin(2.0*t1)*sin(2.0*t2)*sin(2.0*t3)*sin(2.0*t4)*sin(t5) + 0.00042011718750000002619432448724979*cos(2.0*t1)*cos(t5)*sin(t2)*sin(t3)*sin(t4))) - td1*(1.0*td4*(25109.9375*sin(2.0*t2 + 2.0*t3 + 2.0*t4) + 0.00073318229166666670434948649415219*sin(t1 - 2.0*t2) - 0.00073318229166666670434948649415219*sin(t1 + 2.0*t2) + 92110.6*sin(2.0*t2 + 2.0*t3 + t4) - 99949.8*sin(t3 + t4) + 99949.8*sin(2.0*t2 + t3 + t4) - 92110.6*sin(t4) - 112.33*L3*sin(t4 - 1.0*t5) - 0.149375*L3^2*sin(2.0*t2 + 2.0*t3 + 2.0*t4) + 1.195*L4^2*sin(2.0*t2 + 2.0*t3 + 2.0*t4) - 449.32*L4*sin(2.0*t2 + 2.0*t3 + t4) + 0.0746875*L3^2*sin(2.0*t2 + 2.0*t3 + 2.0*t4 - 2.0*t5) + 0.0746875*L3^2*sin(2.0*t2 + 2.0*t3 + 2.0*t4 + 2.0*t5) + 112.33*L3*sin(2.0*t2 + 2.0*t3 + t4 - 1.0*t5) - 61.24375*L3*sin(2.0*t2 + 2.0*t3 + 2.0*t4 + t5) + 487.56*L4*sin(t3 + t4) + 112.33*L3*sin(t4 + t5) - 487.56*L4*sin(2.0*t2 + t3 + t4) - 121.89*L3*sin(t3 + t4 - 1.0*t5) + 121.89*L3*sin(2.0*t2 + t3 + t4 - 1.0*t5) - 112.33*L3*sin(2.0*t2 + 2.0*t3 + t4 + t5) + 449.32*L4*sin(t4) - 244.975*L4*sin(2.0*t2 + 2.0*t3 + 2.0*t4) + 61.24375*L3*sin(2.0*t2 + 2.0*t3 + 2.0*t4 - 1.0*t5) + 121.89*L3*sin(t3 + t4 + t5) - 121.89*L3*sin(2.0*t2 + t3 + t4 + t5) - 0.5975*L3*L4*sin(2.0*t2 + 2.0*t3 + 2.0*t4 - 1.0*t5) + 0.5975*L3*L4*sin(2.0*t2 + 2.0*t3 + 2.0*t4 + t5)) - td5*(0.00036659114583333335217474324707609*sin(3.0*t2 - 1.0*t1 + t3 + t4) + 0.00036659114583333335217474324707609*sin(t1 - 1.0*t2 + t3 + t4) - 0.00036659114583333335217474324707609*sin(t1 + 3.0*t2 + t3 + t4) + 0.00036659114583333335217474324707609*sin(t1 + t2 - 1.0*t3 - 1.0*t4) - 112.33*L3*sin(t4 - 1.0*t5) + 0.0746875*L3^2*sin(2.0*t2 + 2.0*t3 + 2.0*t4 - 2.0*t5) - 0.0746875*L3^2*sin(2.0*t2 + 2.0*t3 + 2.0*t4 + 2.0*t5) + 112.33*L3*sin(2.0*t2 + 2.0*t3 + t4 - 1.0*t5) + 30.621875*L3*sin(2.0*t2 + 2.0*t3 + 2.0*t4 + t5) - 112.33*L3*sin(t4 + t5) - 121.89*L3*sin(t3 + t4 - 1.0*t5) + 121.89*L3*sin(2.0*t2 + t3 + t4 - 1.0*t5) + 112.33*L3*sin(2.0*t2 + 2.0*t3 + t4 + t5) + 0.149375*L3^2*sin(2.0*t5) + 167.8975*L3*sin(t5) + 30.621875*L3*sin(2.0*t2 + 2.0*t3 + 2.0*t4 - 1.0*t5) - 121.89*L3*sin(t3 + t4 + t5) + 121.89*L3*sin(2.0*t2 + t3 + t4 + t5) - 0.29875*L3*L4*sin(2.0*t2 + 2.0*t3 + 2.0*t4 - 1.0*t5) - 0.29875*L3*L4*sin(2.0*t2 + 2.0*t3 + 2.0*t4 + t5)) + 1.0*td2*(25109.9375*sin(2.0*t2 + 2.0*t3 + 2.0*t4) - 0.02665555083333333167075474001706*sin(t1 - 2.0*t2) + 0.02665555083333333167075474001706*sin(t1 + 2.0*t2) + 1339251.84*sin(2.0*t2 + t3) + 184221.2*sin(2.0*t2 + 2.0*t3 + t4) + 1047890.8266888983333333366584905*sin(2.0*t2) + 199899.6*sin(2.0*t2 + t3 + t4) + 617106.24*sin(2.0*t2 + 2.0*t3) - 265.89625*L2*sin(t1 - 1.0*t2) - 0.149375*L3^2*sin(2.0*t2 + 2.0*t3 + 2.0*t4) + 1.195*L4^2*sin(2.0*t2 + 2.0*t3 + 2.0*t4) - 898.64*L4*sin(2.0*t2 + 2.0*t3 + t4) + 0.0746875*L3^2*sin(2.0*t2 + 2.0*t3 + 2.0*t4 - 2.0*t5) + 0.0746875*L3^2*sin(2.0*t2 + 2.0*t3 + 2.0*t4 + 2.0*t5) + 224.66*L3*sin(2.0*t2 + 2.0*t3 + t4 - 1.0*t5) - 61.24375*L3*sin(2.0*t2 + 2.0*t3 + 2.0*t4 + t5) - 0.473125*L2^2*sin(t1 - 2.0*t2) + 0.473125*L2^2*sin(t1 + 2.0*t2) - 265.89625*L2*sin(t1 + t2) - 975.12*L4*sin(2.0*t2 + t3 + t4) + 243.78*L3*sin(2.0*t2 + t3 + t4 - 1.0*t5) - 224.66*L3*sin(2.0*t2 + 2.0*t3 + t4 + t5) + 0.94625*L2^2*sin(2.0*t2) - 244.975*L4*sin(2.0*t2 + 2.0*t3 + 2.0*t4) + 61.24375*L3*sin(2.0*t2 + 2.0*t3 + 2.0*t4 - 1.0*t5) - 243.78*L3*sin(2.0*t2 + t3 + t4 + t5) - 0.5975*L3*L4*sin(2.0*t2 + 2.0*t3 + 2.0*t4 - 1.0*t5) + 0.5975*L3*L4*sin(2.0*t2 + 2.0*t3 + 2.0*t4 + t5)) + 1.0*td3*(25109.9375*sin(2.0*t2 + 2.0*t3 + 2.0*t4) + 0.00073318229166666670434948649415219*sin(t1 - 2.0*t2) - 0.00073318229166666670434948649415219*sin(t1 + 2.0*t2) + 669625.92*sin(2.0*t2 + t3) + 184221.2*sin(2.0*t2 + 2.0*t3 + t4) - 99949.8*sin(t3 + t4) + 99949.8*sin(2.0*t2 + t3 + t4) - 669625.92*sin(t3) + 617106.24*sin(2.0*t2 + 2.0*t3) - 0.149375*L3^2*sin(2.0*t2 + 2.0*t3 + 2.0*t4) + 1.195*L4^2*sin(2.0*t2 + 2.0*t3 + 2.0*t4) - 898.64*L4*sin(2.0*t2 + 2.0*t3 + t4) + 0.0746875*L3^2*sin(2.0*t2 + 2.0*t3 + 2.0*t4 - 2.0*t5) + 0.0746875*L3^2*sin(2.0*t2 + 2.0*t3 + 2.0*t4 + 2.0*t5) + 224.66*L3*sin(2.0*t2 + 2.0*t3 + t4 - 1.0*t5) - 61.24375*L3*sin(2.0*t2 + 2.0*t3 + 2.0*t4 + t5) + 487.56*L4*sin(t3 + t4) - 487.56*L4*sin(2.0*t2 + t3 + t4) - 121.89*L3*sin(t3 + t4 - 1.0*t5) + 121.89*L3*sin(2.0*t2 + t3 + t4 - 1.0*t5) - 224.66*L3*sin(2.0*t2 + 2.0*t3 + t4 + t5) - 244.975*L4*sin(2.0*t2 + 2.0*t3 + 2.0*t4) + 61.24375*L3*sin(2.0*t2 + 2.0*t3 + 2.0*t4 - 1.0*t5) + 121.89*L3*sin(t3 + t4 + t5) - 121.89*L3*sin(2.0*t2 + t3 + t4 + t5) - 0.5975*L3*L4*sin(2.0*t2 + 2.0*t3 + 2.0*t4 - 1.0*t5) + 0.5975*L3*L4*sin(2.0*t2 + 2.0*t3 + 2.0*t4 + t5)))
    td6*(td1*(0.00084023437500000005238864897449957*cos(t1)*cos(t5)*sin(t1) + 0.00042011718750000002619432448724979*cos(t1)^2*cos(t2)*cos(t3)*cos(t4)*sin(t5) - 0.00042011718750000002619432448724979*cos(t2)*cos(t3)*cos(t4)*sin(t1)^2*sin(t5) - 0.00042011718750000002619432448724979*cos(t1)^2*cos(t2)*sin(t3)*sin(t4)*sin(t5) - 0.00042011718750000002619432448724979*cos(t1)^2*cos(t3)*sin(t2)*sin(t4)*sin(t5) - 0.00042011718750000002619432448724979*cos(t1)^2*cos(t4)*sin(t2)*sin(t3)*sin(t5) + 0.00042011718750000002619432448724979*cos(t2)*sin(t1)^2*sin(t3)*sin(t4)*sin(t5) + 0.00042011718750000002619432448724979*cos(t3)*sin(t1)^2*sin(t2)*sin(t4)*sin(t5) + 0.00042011718750000002619432448724979*cos(t4)*sin(t1)^2*sin(t2)*sin(t3)*sin(t5)) + td6*(0.5*(0.00084023437500000005238864897449957*cos(t1)*cos(t2)*cos(t3)*sin(t4)*sin(t5) + 0.00084023437500000005238864897449957*cos(t1)*cos(t2)*cos(t4)*sin(t3)*sin(t5) + 0.00084023437500000005238864897449957*cos(t1)*cos(t3)*cos(t4)*sin(t2)*sin(t5) - 0.00084023437500000005238864897449957*cos(t1)*sin(t2)*sin(t3)*sin(t4)*sin(t5))*(cos(t1)*cos(t2)*sin(t3)*sin(t4)*sin(t5) - 1.0*cos(t1)*cos(t2)*cos(t3)*cos(t4)*sin(t5) - 1.0*cos(t5)*sin(t1) + cos(t1)*cos(t3)*sin(t2)*sin(t4)*sin(t5) + cos(t1)*cos(t4)*sin(t2)*sin(t3)*sin(t5)) + 0.5*(cos(t1)*cos(t2)*cos(t3)*sin(t4)*sin(t5) + cos(t1)*cos(t2)*cos(t4)*sin(t3)*sin(t5) + cos(t1)*cos(t3)*cos(t4)*sin(t2)*sin(t5) - 1.0*cos(t1)*sin(t2)*sin(t3)*sin(t4)*sin(t5))*(0.00084023437500000005238864897449957*cos(t1)*cos(t2)*sin(t3)*sin(t4)*sin(t5) - 0.00084023437500000005238864897449957*cos(t1)*cos(t2)*cos(t3)*cos(t4)*sin(t5) - 0.00084023437500000005238864897449957*cos(t5)*sin(t1) + 0.00084023437500000005238864897449957*cos(t1)*cos(t3)*sin(t2)*sin(t4)*sin(t5) + 0.00084023437500000005238864897449957*cos(t1)*cos(t4)*sin(t2)*sin(t3)*sin(t5)) + 0.5*(0.0016804687500000001047772979489991*cos(t2)*cos(t3)*sin(t1)*sin(t4)*sin(t5) + 0.0016804687500000001047772979489991*cos(t2)*cos(t4)*sin(t1)*sin(t3)*sin(t5) + 0.0016804687500000001047772979489991*cos(t3)*cos(t4)*sin(t1)*sin(t2)*sin(t5) - 0.0016804687500000001047772979489991*sin(t1)*sin(t2)*sin(t3)*sin(t4)*sin(t5))*(cos(t1)*cos(t5) - 1.0*cos(t2)*cos(t3)*cos(t4)*sin(t1)*sin(t5) + cos(t2)*sin(t1)*sin(t3)*sin(t4)*sin(t5) + cos(t3)*sin(t1)*sin(t2)*sin(t4)*sin(t5) + cos(t4)*sin(t1)*sin(t2)*sin(t3)*sin(t5)) + 0.5*(cos(t2)*cos(t3)*sin(t1)*sin(t4)*sin(t5) + cos(t2)*cos(t4)*sin(t1)*sin(t3)*sin(t5) + cos(t3)*cos(t4)*sin(t1)*sin(t2)*sin(t5) - 1.0*sin(t1)*sin(t2)*sin(t3)*sin(t4)*sin(t5))*(0.0016804687500000001047772979489991*cos(t1)*cos(t5) - 0.0016804687500000001047772979489991*cos(t2)*cos(t3)*cos(t4)*sin(t1)*sin(t5) + 0.0016804687500000001047772979489991*cos(t2)*sin(t1)*sin(t3)*sin(t4)*sin(t5) + 0.0016804687500000001047772979489991*cos(t3)*sin(t1)*sin(t2)*sin(t4)*sin(t5) + 0.0016804687500000001047772979489991*cos(t4)*sin(t1)*sin(t2)*sin(t3)*sin(t5))) - 1.0*td5*(0.00063017578125000003929148673087468*cos(2.0*t2)*cos(2.0*t3)*cos(2.0*t4)*sin(t5) - 0.00042011718750000002619432448724979*cos(t1)^2*sin(t5) - 0.00042011718750000002619432448724979*sin(t5) - 0.00063017578125000003929148673087468*cos(2.0*t2)*sin(2.0*t3)*sin(2.0*t4)*sin(t5) - 0.00063017578125000003929148673087468*cos(2.0*t3)*sin(2.0*t2)*sin(2.0*t4)*sin(t5) - 0.00063017578125000003929148673087468*cos(2.0*t4)*sin(2.0*t2)*sin(2.0*t3)*sin(t5) - 0.00021005859375000001309716224362489*cos(2.0*t1)*cos(2.0*t2)*cos(2.0*t3)*cos(2.0*t4)*sin(t5) + 0.00021005859375000001309716224362489*cos(2.0*t1)*cos(2.0*t2)*sin(2.0*t3)*sin(2.0*t4)*sin(t5) + 0.00021005859375000001309716224362489*cos(2.0*t1)*cos(2.0*t3)*sin(2.0*t2)*sin(2.0*t4)*sin(t5) + 0.00021005859375000001309716224362489*cos(2.0*t1)*cos(2.0*t4)*sin(2.0*t2)*sin(2.0*t3)*sin(t5) - 0.00021005859375000001309716224362489*sin(2.0*t1)*cos(t2)*cos(t3)*cos(t4)*cos(t5) + 0.00021005859375000001309716224362489*sin(2.0*t1)*cos(t2)*cos(t5)*sin(t3)*sin(t4) + 0.00021005859375000001309716224362489*sin(2.0*t1)*cos(t3)*cos(t5)*sin(t2)*sin(t4) + 0.00021005859375000001309716224362489*sin(2.0*t1)*cos(t4)*cos(t5)*sin(t2)*sin(t3) - 0.00042011718750000002619432448724979*cos(t1)*cos(t2)*cos(t3)*cos(t4)*cos(t5)*sin(t1) + 0.00042011718750000002619432448724979*cos(t1)*cos(t2)*cos(t5)*sin(t1)*sin(t3)*sin(t4) + 0.00042011718750000002619432448724979*cos(t1)*cos(t3)*cos(t5)*sin(t1)*sin(t2)*sin(t4) + 0.00042011718750000002619432448724979*cos(t1)*cos(t4)*cos(t5)*sin(t1)*sin(t2)*sin(t3))) - td2*(1.0*td4*(0.0014663645833333334086989729883044*sin(2.0*t2) - 184221.2*sin(t4) - 199899.6*cos(t3)*sin(t4) - 199899.6*cos(t4)*sin(t3) - 0.0014663645833333334086989729883044*cos(2.0*t1)*sin(2.0*t2) + 898.64*L4*sin(t4) + 975.12*L4*cos(t3)*sin(t4) + 975.12*L4*cos(t4)*sin(t3) + 449.32*L3*cos(t4)*sin(t5) + 487.56*L3*cos(t3)*cos(t4)*sin(t5) - 487.56*L3*sin(t3)*sin(t4)*sin(t5)) - td3*(1339251.84*sin(t3) - 0.0058654583333333336347958919532175*cos(t2)*sin(t2) + 0.0029327291666666668173979459766088*cos(t3)*sin(t3) + 199899.6*cos(t3)*sin(t4) + 199899.6*cos(t4)*sin(t3) + 0.0029327291666666668173979459766088*cos(t1)*cos(t3)^2*sin(t1) + 0.0058654583333333336347958919532175*cos(t1)^2*cos(t2)*sin(t2) - 0.0058654583333333336347958919532175*cos(t1)^2*cos(t3)*sin(t3) - 0.0029327291666666668173979459766088*cos(t1)*sin(t1)*sin(t3)^2 - 975.12*L4*cos(t3)*sin(t4) - 975.12*L4*cos(t4)*sin(t3) - 487.56*L3*cos(t3)*cos(t4)*sin(t5) + 487.56*L3*sin(t3)*sin(t4)*sin(t5)) + td5*(0.0010997734375000000565242297412283*sin(3.0*t2 - 1.0*t1 + t3 + t4) - 0.00073318229166666670434948649415219*sin(t2 - 2.0*t1 + 3.0*t3 + t4) - 0.00054988671875000002826211487061414*sin(3.0*t2 - 2.0*t1 + t3 + t4) + 0.00054988671875000002826211487061414*sin(2.0*t1 + 3.0*t2 + t3 + t4) - 0.00036659114583333335217474324707609*sin(t1 - 1.0*t2 + t3 + t4) + 0.00057664973958333336527190549070099*sin(t2 - 2.0*t1 + t3 + t4) - 0.00057664973958333336527190549070099*sin(2.0*t1 + t2 + t3 + t4) - 0.0010997734375000000565242297412283*sin(t1 + 3.0*t2 + t3 + t4) - 0.00018329557291666667608737162353805*sin(2.0*t1 + t2 - 1.0*t3 - 1.0*t4) - 0.00036659114583333335217474324707609*sin(t1 + t2 - 1.0*t3 - 1.0*t4) + 0.00073318229166666670434948649415219*sin(2.0*t1 + t2 - 1.0*t3 + t4) - 0.00018329557291666667608737162353805*sin(2.0*t1 - 1.0*t2 + t3 + t4) + 449.32*L3*cos(t5)*sin(t4) + 0.5975*L3^2*cos(t5)*sin(t5) + 487.56*L3*cos(t3)*cos(t5)*sin(t4) + 487.56*L3*cos(t4)*cos(t5)*sin(t3)) + 1.0*td1*(0.053311101666666663341509480034119*sin(t1 - 2.0*t2) - 68837.975*sin(t2 + t3 + t4) + 0.053311101666666663341509480034119*sin(t1 + 2.0*t2) - 461188.44*sin(t2 + t3) - 721709.16*sin(t2) + 265.89625*L2*sin(t1 - 1.0*t2) - 243.78*L3*sin(t2 - 1.0*t5) + 149433.79717526104166665983606632*cos(t1)*sin(t1) - 0.149375*L3^2*sin(t2 + t3 + t4 - 2.0*t5) + 0.149375*L3^2*sin(t2 + t3 + t4 + 2.0*t5) + 22.705*L3*sin(t2 + t3 + t4 + t5) + 0.94625*L2^2*sin(t1 - 2.0*t2) + 0.94625*L2^2*sin(t1 + 2.0*t2) - 265.89625*L2*sin(t1 + t2) + 1485.2*L1*sin(t2 + t3) - 243.78*L3*sin(t2 + t5) - 224.66*L3*sin(t2 + t3 - 1.0*t5) + 3186.48*L1*sin(t2) - 224.66*L3*sin(t2 + t3 + t5) + 335.795*L4*sin(t2 + t3 + t4) - 145.1925*L3*sin(t2 + t3 + t4 - 1.0*t5) + 0.5975*L3*L4*sin(t2 + t3 + t4 - 1.0*t5) - 0.10662220333333332668301896006824*cos(t1)*cos(t2)^2*sin(t1) + 0.0058654583333333336347958919532175*cos(t1)*cos(t3)^2*sin(t1) - 0.0029327291666666668173979459766088*cos(t1)^2*cos(t3)*sin(t3) + 0.0029327291666666668173979459766088*cos(t3)*sin(t1)^2*sin(t3) + 0.5975*L3*L4*sin(t2 + t3 + t4 + t5) - 1.8925*L2^2*cos(t1)*sin(t1) - 531.7925*L2*cos(t1)^2*sin(t2) + 531.7925*L2*sin(t1)^2*sin(t2) + 1.8925*L2^2*cos(t1)*cos(t2)^2*sin(t1)) - td6*(0.00084023437500000005238864897449957*cos(t1)*cos(t2)*cos(t3)*sin(t1)*sin(t4)*sin(t5) + 0.00084023437500000005238864897449957*cos(t1)*cos(t2)*cos(t4)*sin(t1)*sin(t3)*sin(t5) + 0.00084023437500000005238864897449957*cos(t1)*cos(t3)*cos(t4)*sin(t1)*sin(t2)*sin(t5) - 0.00084023437500000005238864897449957*cos(t1)*sin(t1)*sin(t2)*sin(t3)*sin(t4)*sin(t5)) + 1.0*td2*(- 1.8925*cos(t2)*sin(t2)*L2^2*cos(t1)^2 + 1.8925*cos(t2)*sin(t2)*L2^2 + 531.7925*cos(t2)*sin(t1)*L2*cos(t1) + 0.10662220333333332668301896006824*cos(t2)*sin(t2)*cos(t1)^2 - 0.10662220333333332668301896006824*cos(t2)*sin(t2))) - td3*(1.0*td3*(0.0029327291666666668173979459766088*cos(t2)*sin(t2) - 0.0029327291666666668173979459766088*cos(t1)^2*cos(t2)*sin(t2)) - td6*(0.00084023437500000005238864897449957*cos(t1)*cos(t2)*cos(t3)*sin(t1)*sin(t4)*sin(t5) + 0.00084023437500000005238864897449957*cos(t1)*cos(t2)*cos(t4)*sin(t1)*sin(t3)*sin(t5) + 0.00084023437500000005238864897449957*cos(t1)*cos(t3)*cos(t4)*sin(t1)*sin(t2)*sin(t5) - 0.00084023437500000005238864897449957*cos(t1)*sin(t1)*sin(t2)*sin(t3)*sin(t4)*sin(t5)) - td1*(68837.975*sin(t2 + t3 + t4) + 0.00073318229166666670434948649415219*sin(t1 - 2.0*t2) + 0.00073318229166666670434948649415219*sin(t1 + 2.0*t2) + 461188.44*sin(t2 + t3) + 0.0048796714583333336643505839802515*cos(t1)*sin(t1) + 0.149375*L3^2*sin(t2 + t3 + t4 - 2.0*t5) - 0.149375*L3^2*sin(t2 + t3 + t4 + 2.0*t5) - 22.705*L3*sin(t2 + t3 + t4 + t5) - 1485.2*L1*sin(t2 + t3) + 224.66*L3*sin(t2 + t3 - 1.0*t5) + 224.66*L3*sin(t2 + t3 + t5) - 335.795*L4*sin(t2 + t3 + t4) + 145.1925*L3*sin(t2 + t3 + t4 - 1.0*t5) - 0.5975*L3*L4*sin(t2 + t3 + t4 - 1.0*t5) - 0.0029327291666666668173979459766088*cos(t1)*cos(t2)^2*sin(t1) - 0.0058654583333333336347958919532175*cos(t1)*cos(t3)^2*sin(t1) + 0.0029327291666666668173979459766088*cos(t1)^2*cos(t3)*sin(t3) - 0.0029327291666666668173979459766088*cos(t3)*sin(t1)^2*sin(t3) - 0.5975*L3*L4*sin(t2 + t3 + t4 + t5)) + 1.0*td2*(1339251.84*sin(t3) + 0.0029327291666666668173979459766088*cos(t3)*sin(t3) + 199899.6*cos(t3)*sin(t4) + 199899.6*cos(t4)*sin(t3) + 0.0029327291666666668173979459766088*cos(t1)*cos(t3)^2*sin(t1) - 0.0058654583333333336347958919532175*cos(t1)^2*cos(t3)*sin(t3) - 0.0029327291666666668173979459766088*cos(t1)*sin(t1)*sin(t3)^2 - 975.12*L4*cos(t3)*sin(t4) - 975.12*L4*cos(t4)*sin(t3) - 487.56*L3*cos(t3)*cos(t4)*sin(t5) + 487.56*L3*sin(t3)*sin(t4)*sin(t5)) + 1.0*td5*(0.00073318229166666670434948649415219*sin(3.0*t2 - 1.0*t1 + t3 + t4) - 0.0014663645833333334086989729883044*sin(t2 - 2.0*t1 + 3.0*t3 + t4) - 0.00036659114583333335217474324707609*sin(3.0*t2 - 2.0*t1 + t3 + t4) + 0.00036659114583333335217474324707609*sin(2.0*t1 + 3.0*t2 + t3 + t4) + 0.00057664973958333336527190549070099*sin(t2 - 2.0*t1 + t3 + t4) - 0.00057664973958333336527190549070099*sin(2.0*t1 + t2 + t3 + t4) - 0.00073318229166666670434948649415219*sin(t1 + 3.0*t2 + t3 + t4) - 121.89*L3*sin(t3 + t4 - 1.0*t5) - 121.89*L3*sin(t3 + t4 + t5) + 449.32*L3*cos(t5)*sin(t4) + 0.5975*L3^2*cos(t5)*sin(t5) + 243.78*L3*cos(t3)*cos(t5)*sin(t4) + 243.78*L3*cos(t4)*cos(t5)*sin(t3)) - td4*(0.0029327291666666668173979459766088*cos(t2)*sin(t2)*cos(t1)^2 - 0.0014663645833333334086989729883044*sin(2.0*t1)*cos(t3)^2 + 0.0029327291666666668173979459766088*cos(2.0*t1)*cos(t3)*sin(t3) + 0.0014663645833333334086989729883044*sin(2.0*t1)*sin(t3)^2 + 184221.2*sin(t4) - 0.0029327291666666668173979459766088*cos(t2)*sin(t2) - 898.64*L4*sin(t4) - 449.32*L3*cos(t4)*sin(t5))) + td1*(td1*(25109.9375*sin(2.0*t2 + 2.0*t3 + 2.0*t4) + 1339251.84*sin(2.0*t2 + t3) + 184221.2*sin(2.0*t2 + 2.0*t3 + t4) + 1047890.8266888983333333366584905*sin(2.0*t2) + 199899.6*sin(2.0*t2 + t3 + t4) + 617106.24*sin(2.0*t2 + 2.0*t3) - 0.149375*L3^2*sin(2.0*t2 + 2.0*t3 + 2.0*t4) + 1.195*L4^2*sin(2.0*t2 + 2.0*t3 + 2.0*t4) - 898.64*L4*sin(2.0*t2 + 2.0*t3 + t4) + 0.0746875*L3^2*sin(2.0*t2 + 2.0*t3 + 2.0*t4 - 2.0*t5) + 0.0746875*L3^2*sin(2.0*t2 + 2.0*t3 + 2.0*t4 + 2.0*t5) + 224.66*L3*sin(2.0*t2 + 2.0*t3 + t4 - 1.0*t5) - 61.24375*L3*sin(2.0*t2 + 2.0*t3 + 2.0*t4 + t5) - 975.12*L4*sin(2.0*t2 + t3 + t4) + 243.78*L3*sin(2.0*t2 + t3 + t4 - 1.0*t5) - 224.66*L3*sin(2.0*t2 + 2.0*t3 + t4 + t5) + 0.94625*L2^2*sin(2.0*t2) - 244.975*L4*sin(2.0*t2 + 2.0*t3 + 2.0*t4) + 61.24375*L3*sin(2.0*t2 + 2.0*t3 + 2.0*t4 - 1.0*t5) - 243.78*L3*sin(2.0*t2 + t3 + t4 + t5) - 0.5975*L3*L4*sin(2.0*t2 + 2.0*t3 + 2.0*t4 - 1.0*t5) + 0.5975*L3*L4*sin(2.0*t2 + 2.0*t3 + 2.0*t4 + t5)) - 1.0*td5*(0.00036659114583333335217474324707609*sin(3.0*t2 - 1.0*t1 + t3 + t4) + 0.00073318229166666670434948649415219*sin(t2 - 2.0*t1 + 3.0*t3 + t4) + 0.00018329557291666667608737162353805*sin(3.0*t2 - 2.0*t1 + t3 + t4) + 0.00018329557291666667608737162353805*sin(2.0*t1 + 3.0*t2 + t3 + t4) + 0.00073318229166666670434948649415219*sin(t2 + t3 + t4) + 0.00036659114583333335217474324707609*sin(t1 - 1.0*t2 + t3 + t4) - 0.00057664973958333336527190549070099*sin(t2 - 2.0*t1 + t3 + t4) - 0.00057664973958333336527190549070099*sin(2.0*t1 + t2 + t3 + t4) + 0.00036659114583333335217474324707609*sin(t1 + 3.0*t2 + t3 + t4) - 0.00018329557291666667608737162353805*sin(2.0*t1 + t2 - 1.0*t3 - 1.0*t4) + 0.00036659114583333335217474324707609*sin(t3 - 1.0*t2 + t4) - 0.00036659114583333335217474324707609*sin(t1 + t2 - 1.0*t3 - 1.0*t4) + 0.00073318229166666670434948649415219*sin(2.0*t1 + t2 - 1.0*t3 + t4) + 0.00018329557291666667608737162353805*sin(2.0*t1 - 1.0*t2 + t3 + t4) - 0.0010997734375000000565242297412283*sin(3.0*t2 + t3 + t4) - 243.78*L3*sin(t2 - 1.0*t5) + 0.29875*L3^2*sin(t2 + t3 + t4) - 0.149375*L3^2*sin(t2 + t3 + t4 - 2.0*t5) - 0.149375*L3^2*sin(t2 + t3 + t4 + 2.0*t5) + 61.24375*L3*sin(t2 + t3 + t4 + t5) + 243.78*L3*sin(t2 + t5) - 224.66*L3*sin(t2 + t3 - 1.0*t5) + 224.66*L3*sin(t2 + t3 + t5) - 61.24375*L3*sin(t2 + t3 + t4 - 1.0*t5) + 0.5975*L3*L4*sin(t2 + t3 + t4 - 1.0*t5) - 0.5975*L3*L4*sin(t2 + t3 + t4 + t5)) - 1.0*td6*(0.00084023437500000005238864897449957*cos(t1)*cos(t5)*sin(t1) + 0.00042011718750000002619432448724979*cos(t1)^2*cos(t2)*cos(t3)*cos(t4)*sin(t5) - 0.00042011718750000002619432448724979*cos(t2)*cos(t3)*cos(t4)*sin(t1)^2*sin(t5) - 0.00042011718750000002619432448724979*cos(t1)^2*cos(t2)*sin(t3)*sin(t4)*sin(t5) - 0.00042011718750000002619432448724979*cos(t1)^2*cos(t3)*sin(t2)*sin(t4)*sin(t5) - 0.00042011718750000002619432448724979*cos(t1)^2*cos(t4)*sin(t2)*sin(t3)*sin(t5) + 0.00042011718750000002619432448724979*cos(t2)*sin(t1)^2*sin(t3)*sin(t4)*sin(t5) + 0.00042011718750000002619432448724979*cos(t3)*sin(t1)^2*sin(t2)*sin(t4)*sin(t5) + 0.00042011718750000002619432448724979*cos(t4)*sin(t1)^2*sin(t2)*sin(t3)*sin(t5)) + td2*(1.8925*L2^2*cos(t1)*cos(t2)^2*sin(t1) - 1.8925*L2^2*cos(t1)*sin(t1) - 531.7925*sin(t2)*L2*cos(t1)^2 + 531.7925*sin(t2)*L2*sin(t1)^2 - 0.0029327291666666668173979459766088*sin(t3)*cos(t1)^2*cos(t3) - 0.10662220333333332668301896006824*cos(t1)*cos(t2)^2*sin(t1) + 0.0058654583333333336347958919532175*cos(t1)*cos(t3)^2*sin(t1) + 149433.79717526104166665983606632*cos(t1)*sin(t1) + 0.0029327291666666668173979459766088*sin(t3)*cos(t3)*sin(t1)^2) + td3*(- 0.0029327291666666668173979459766088*sin(t3)*cos(t1)^2*cos(t3) + 0.0029327291666666668173979459766088*cos(t1)*cos(t2)^2*sin(t1) + 0.0058654583333333336347958919532175*cos(t1)*cos(t3)^2*sin(t1) - 0.0048796714583333336643505839802515*cos(t1)*sin(t1) + 0.0029327291666666668173979459766088*sin(t3)*cos(t3)*sin(t1)^2 + 0.00073318229166666670434948649415219*sin(t1 - 2.0*t2) + 0.00073318229166666670434948649415219*sin(t1 + 2.0*t2)) + td4*(0.0029327291666666668173979459766088*sin(2.0*t1)*cos(t3)^2 - 0.0029327291666666668173979459766088*cos(2.0*t1)*sin(t3)*cos(t3) + 0.00073318229166666670434948649415219*sin(t1 - 2.0*t2) + 0.00073318229166666670434948649415219*sin(t1 + 2.0*t2) - 0.0026196640625000001392427839697064*sin(2.0*t1) + 0.00073318229166666670434948649415219*cos(2.0*t2)*sin(2.0*t1))) + td5*(td4*(0.00018329557291666667608737162353805*sin(3.0*t2 - 2.0*t1 + t3 + t4) - 0.00036659114583333335217474324707609*sin(3.0*t2 - 1.0*t1 + t3 + t4) - 0.00018329557291666667608737162353805*sin(2.0*t1 + 3.0*t2 + t3 + t4) + 0.00036659114583333335217474324707609*sin(t1 - 1.0*t2 + t3 + t4) + 0.00036659114583333335217474324707609*sin(t1 + 3.0*t2 + t3 + t4) + 0.00018329557291666667608737162353805*sin(2.0*t1 + t2 - 1.0*t3 - 1.0*t4) + 0.00036659114583333335217474324707609*sin(t1 + t2 - 1.0*t3 - 1.0*t4) + 0.00018329557291666667608737162353805*sin(2.0*t1 - 1.0*t2 + t3 + t4) - 112.33*L3*sin(t4 - 1.0*t5) - 112.33*L3*sin(t4 + t5) - 121.89*L3*sin(t3 + t4 - 1.0*t5) - 121.89*L3*sin(t3 + t4 + t5) + 224.66*L3*cos(t5)*sin(t4) + 0.5975*L3^2*cos(t5)*sin(t5) + 243.78*L3*cos(t3)*cos(t5)*sin(t4) + 243.78*L3*cos(t4)*cos(t5)*sin(t3)) + td3*(0.00018329557291666667608737162353805*sin(3.0*t2 - 2.0*t1 + t3 + t4) - 0.00073318229166666670434948649415219*sin(t2 - 2.0*t1 + 3.0*t3 + t4) - 0.00036659114583333335217474324707609*sin(3.0*t2 - 1.0*t1 + t3 + t4) - 0.00018329557291666667608737162353805*sin(2.0*t1 + 3.0*t2 + t3 + t4) + 0.00036659114583333335217474324707609*sin(t1 - 1.0*t2 + t3 + t4) + 0.00036659114583333335217474324707609*sin(t1 + 3.0*t2 + t3 + t4) + 0.00018329557291666667608737162353805*sin(2.0*t1 + t2 - 1.0*t3 - 1.0*t4) + 0.00036659114583333335217474324707609*sin(t1 + t2 - 1.0*t3 - 1.0*t4) - 0.00073318229166666670434948649415219*sin(2.0*t1 + t2 - 1.0*t3 + t4) + 0.00018329557291666667608737162353805*sin(2.0*t1 - 1.0*t2 + t3 + t4) - 121.89*L3*sin(t3 + t4 - 1.0*t5) - 121.89*L3*sin(t3 + t4 + t5) + 449.32*L3*cos(t5)*sin(t4) + 0.5975*L3^2*cos(t5)*sin(t5) + 243.78*L3*cos(t3)*cos(t5)*sin(t4) + 243.78*L3*cos(t4)*cos(t5)*sin(t3)) - 1.0*td1*(0.00073318229166666670434948649415219*sin(3.0*t2 - 1.0*t1 + t3 + t4) - 0.00073318229166666670434948649415219*sin(t2 - 2.0*t1 + 3.0*t3 + t4) - 0.00018329557291666667608737162353805*sin(3.0*t2 - 2.0*t1 + t3 + t4) - 0.00018329557291666667608737162353805*sin(2.0*t1 + 3.0*t2 + t3 + t4) + 0.00073318229166666670434948649415219*sin(t2 + t3 + t4) + 0.00057664973958333336527190549070099*sin(t2 - 2.0*t1 + t3 + t4) + 0.00057664973958333336527190549070099*sin(2.0*t1 + t2 + t3 + t4) + 0.00073318229166666670434948649415219*sin(t1 + 3.0*t2 + t3 + t4) + 0.00018329557291666667608737162353805*sin(2.0*t1 + t2 - 1.0*t3 - 1.0*t4) + 0.00036659114583333335217474324707609*sin(t3 - 1.0*t2 + t4) - 0.00073318229166666670434948649415219*sin(2.0*t1 + t2 - 1.0*t3 + t4) - 0.00018329557291666667608737162353805*sin(2.0*t1 - 1.0*t2 + t3 + t4) - 0.0010997734375000000565242297412283*sin(3.0*t2 + t3 + t4) + 0.29875*L3^2*sin(t2 + t3 + t4) + 0.149375*L3^2*sin(t2 + t3 + t4 - 2.0*t5) + 0.149375*L3^2*sin(t2 + t3 + t4 + 2.0*t5) + 83.94875*L3*sin(t2 + t3 + t4 + t5) + 83.94875*L3*sin(t2 + t3 + t4 - 1.0*t5)) + td2*(449.32*L3*cos(t5)*sin(t4) + 0.5975*L3^2*cos(t5)*sin(t5) + 487.56*L3*cos(t3)*cos(t5)*sin(t4) + 487.56*L3*cos(t4)*cos(t5)*sin(t3)) + td5*(0.00036659114583333335217474324707609*sin(2.0*t1 + 2.0*t2 + 2.0*t4) + 0.001729949218750000095815716472103*sin(2.0*t2 + 2.0*t3 + 2.0*t4) + 0.0010997734375000000565242297412283*sin(4.0*t2 + 2.0*t3 + 2.0*t4) - 0.00073318229166666670434948649415219*sin(4.0*t2 - 1.0*t1 + 2.0*t3 + 2.0*t4) - 0.00028832486979166668263595274535049*sin(2.0*t2 - 2.0*t1 + 2.0*t3 + 2.0*t4) - 0.00028832486979166668263595274535049*sin(2.0*t1 + 2.0*t2 + 2.0*t3 + 2.0*t4) + 0.00036659114583333335217474324707609*sin(2.0*t2 - 2.0*t1 + 4.0*t3 + 2.0*t4) + 0.00018329557291666667608737162353805*sin(4.0*t2 - 2.0*t1 + 2.0*t3 + 2.0*t4) + 0.00018329557291666667608737162353805*sin(2.0*t1 + 4.0*t2 + 2.0*t3 + 2.0*t4) - 0.00073318229166666670434948649415219*sin(t1 + 4.0*t2 + 2.0*t3 + 2.0*t4) + 0.00036659114583333335217474324707609*sin(2.0*t2) + 0.00018329557291666667608737162353805*sin(2.0*t1 - 2.0*t2) - 0.00018329557291666667608737162353805*sin(2.0*t1 + 2.0*t2)) - 1.0*td6*(0.00042011718750000002619432448724979*sin(t5) + 0.00042011718750000002619432448724979*cos(t1)^2*sin(t5) + 0.00063017578125000003929148673087468*cos(2.0*t2)*cos(2.0*t3)*cos(2.0*t4)*sin(t5) - 0.00063017578125000003929148673087468*cos(2.0*t2)*sin(2.0*t3)*sin(2.0*t4)*sin(t5) - 0.00063017578125000003929148673087468*cos(2.0*t3)*sin(2.0*t2)*sin(2.0*t4)*sin(t5) - 0.00063017578125000003929148673087468*cos(2.0*t4)*sin(2.0*t2)*sin(2.0*t3)*sin(t5) - 0.00021005859375000001309716224362489*cos(2.0*t1)*cos(2.0*t2)*cos(2.0*t3)*cos(2.0*t4)*sin(t5) + 0.00021005859375000001309716224362489*cos(2.0*t1)*cos(2.0*t2)*sin(2.0*t3)*sin(2.0*t4)*sin(t5) + 0.00021005859375000001309716224362489*cos(2.0*t1)*cos(2.0*t3)*sin(2.0*t2)*sin(2.0*t4)*sin(t5) + 0.00021005859375000001309716224362489*cos(2.0*t1)*cos(2.0*t4)*sin(2.0*t2)*sin(2.0*t3)*sin(t5) - 0.00021005859375000001309716224362489*sin(2.0*t1)*cos(t2)*cos(t3)*cos(t4)*cos(t5) + 0.00021005859375000001309716224362489*sin(2.0*t1)*cos(t2)*cos(t5)*sin(t3)*sin(t4) + 0.00021005859375000001309716224362489*sin(2.0*t1)*cos(t3)*cos(t5)*sin(t2)*sin(t4) + 0.00021005859375000001309716224362489*sin(2.0*t1)*cos(t4)*cos(t5)*sin(t2)*sin(t3) + 0.00042011718750000002619432448724979*cos(t1)*cos(t2)*cos(t3)*cos(t4)*cos(t5)*sin(t1) - 0.00042011718750000002619432448724979*cos(t1)*cos(t2)*cos(t5)*sin(t1)*sin(t3)*sin(t4) - 0.00042011718750000002619432448724979*cos(t1)*cos(t3)*cos(t5)*sin(t1)*sin(t2)*sin(t4) - 0.00042011718750000002619432448724979*cos(t1)*cos(t4)*cos(t5)*sin(t1)*sin(t2)*sin(t3))) + td4*(td2*(898.64*L4*sin(t4) - 199899.6*cos(t3)*sin(t4) - 199899.6*cos(t4)*sin(t3) - 184221.2*sin(t4) + 975.12*L4*cos(t3)*sin(t4) + 975.12*L4*cos(t4)*sin(t3) + 449.32*L3*cos(t4)*sin(t5) + 487.56*L3*cos(t3)*cos(t4)*sin(t5) - 487.56*L3*sin(t3)*sin(t4)*sin(t5)) - 1.0*td4*(0.00073318229166666670434948649415219*sin(2.0*t2) - 0.00073318229166666670434948649415219*cos(2.0*t1)*sin(2.0*t2)) + td1*(68837.975*sin(t2 + t3 + t4) + 0.00073318229166666670434948649415219*sin(t1 - 2.0*t2) + 0.00073318229166666670434948649415219*sin(t1 + 2.0*t2) + 0.0026196640625000001392427839697064*sin(2.0*t1) - 0.0029327291666666668173979459766088*sin(2.0*t1)*cos(t3)^2 + 0.149375*L3^2*sin(t2 + t3 + t4 - 2.0*t5) - 0.149375*L3^2*sin(t2 + t3 + t4 + 2.0*t5) - 22.705*L3*sin(t2 + t3 + t4 + t5) - 0.00073318229166666670434948649415219*cos(2.0*t2)*sin(2.0*t1) - 335.795*L4*sin(t2 + t3 + t4) + 145.1925*L3*sin(t2 + t3 + t4 - 1.0*t5) - 0.5975*L3*L4*sin(t2 + t3 + t4 - 1.0*t5) + 0.0029327291666666668173979459766088*cos(2.0*t1)*cos(t3)*sin(t3) - 0.5975*L3*L4*sin(t2 + t3 + t4 + t5)) + td6*(0.00084023437500000005238864897449957*cos(t1)*cos(t2)*cos(t3)*sin(t1)*sin(t4)*sin(t5) + 0.00084023437500000005238864897449957*cos(t1)*cos(t2)*cos(t4)*sin(t1)*sin(t3)*sin(t5) + 0.00084023437500000005238864897449957*cos(t1)*cos(t3)*cos(t4)*sin(t1)*sin(t2)*sin(t5) - 0.00084023437500000005238864897449957*cos(t1)*sin(t1)*sin(t2)*sin(t3)*sin(t4)*sin(t5)) - 1.0*td5*(0.00073318229166666670434948649415219*sin(3.0*t2 - 1.0*t1 + t3 + t4) - 0.00073318229166666670434948649415219*sin(t2 - 2.0*t1 + 3.0*t3 + t4) - 0.00036659114583333335217474324707609*sin(3.0*t2 - 2.0*t1 + t3 + t4) + 0.00036659114583333335217474324707609*sin(2.0*t1 + 3.0*t2 + t3 + t4) + 0.00057664973958333336527190549070099*sin(t2 - 2.0*t1 + t3 + t4) - 0.00057664973958333336527190549070099*sin(2.0*t1 + t2 + t3 + t4) - 0.00073318229166666670434948649415219*sin(t1 + 3.0*t2 + t3 + t4) + 0.00073318229166666670434948649415219*sin(2.0*t1 + t2 - 1.0*t3 + t4) - 112.33*L3*sin(t4 - 1.0*t5) - 112.33*L3*sin(t4 + t5) - 121.89*L3*sin(t3 + t4 - 1.0*t5) - 121.89*L3*sin(t3 + t4 + t5) + 224.66*L3*cos(t5)*sin(t4) + 0.5975*L3^2*cos(t5)*sin(t5) + 243.78*L3*cos(t3)*cos(t5)*sin(t4) + 243.78*L3*cos(t4)*cos(t5)*sin(t3)) - 1.0*td3*(- 0.0029327291666666668173979459766088*cos(t2)*sin(t2)*cos(t1)^2 - 0.0014663645833333334086989729883044*sin(2.0*t1)*cos(t3)^2 + 0.0029327291666666668173979459766088*cos(2.0*t1)*cos(t3)*sin(t3) + 0.0014663645833333334086989729883044*sin(2.0*t1)*sin(t3)^2 + 184221.2*sin(t4) + 0.0029327291666666668173979459766088*cos(t2)*sin(t2) - 898.64*L4*sin(t4) - 449.32*L3*cos(t4)*sin(t5)))
    td5*(td5*(0.00036659114583333335217474324707609*sin(2.0*t3 - 1.0*t1 + 2.0*t4) + 0.000091647786458333338043685811769024*sin(2.0*t3 - 2.0*t1 + 2.0*t4) + 0.000091647786458333338043685811769024*sin(2.0*t1 + 2.0*t3 + 2.0*t4) + 0.001729949218750000095815716472103*sin(2.0*t2 + 2.0*t3 + 2.0*t4) + 0.00054988671875000002826211487061414*sin(4.0*t2 + 2.0*t3 + 2.0*t4) - 0.00036659114583333335217474324707609*sin(4.0*t2 - 1.0*t1 + 2.0*t3 + 2.0*t4) - 0.00028832486979166668263595274535049*sin(2.0*t2 - 2.0*t1 + 2.0*t3 + 2.0*t4) - 0.00028832486979166668263595274535049*sin(2.0*t1 + 2.0*t2 + 2.0*t3 + 2.0*t4) + 0.00073318229166666670434948649415219*sin(2.0*t2 - 2.0*t1 + 4.0*t3 + 2.0*t4) + 0.000091647786458333338043685811769024*sin(4.0*t2 - 2.0*t1 + 2.0*t3 + 2.0*t4) + 0.000091647786458333338043685811769024*sin(2.0*t1 + 4.0*t2 + 2.0*t3 + 2.0*t4) + 0.00036659114583333335217474324707609*sin(t1 + 2.0*t3 + 2.0*t4) - 0.00036659114583333335217474324707609*sin(t1 + 4.0*t2 + 2.0*t3 + 2.0*t4) + 0.00073318229166666670434948649415219*sin(2.0*t1 - 2.0*t3) + 0.00054988671875000002826211487061414*sin(2.0*t3 + 2.0*t4)) - 1.0*td1*(0.00036659114583333335217474324707609*sin(3.0*t2 - 1.0*t1 + t3 + t4) - 0.00073318229166666670434948649415219*sin(t2 - 2.0*t1 + 3.0*t3 + t4) - 0.00018329557291666667608737162353805*sin(3.0*t2 - 2.0*t1 + t3 + t4) - 0.00018329557291666667608737162353805*sin(2.0*t1 + 3.0*t2 + t3 + t4) + 0.00073318229166666670434948649415219*sin(t2 + t3 + t4) - 0.00036659114583333335217474324707609*sin(t1 - 1.0*t2 + t3 + t4) + 0.00057664973958333336527190549070099*sin(t2 - 2.0*t1 + t3 + t4) + 0.00057664973958333336527190549070099*sin(2.0*t1 + t2 + t3 + t4) + 0.00036659114583333335217474324707609*sin(t1 + 3.0*t2 + t3 + t4) + 0.00018329557291666667608737162353805*sin(2.0*t1 + t2 - 1.0*t3 - 1.0*t4) - 0.00036659114583333335217474324707609*sin(t3 - 1.0*t2 + t4) + 0.00036659114583333335217474324707609*sin(t1 + t2 - 1.0*t3 - 1.0*t4) - 0.00073318229166666670434948649415219*sin(2.0*t1 + t2 - 1.0*t3 + t4) - 0.00018329557291666667608737162353805*sin(2.0*t1 - 1.0*t2 + t3 + t4) - 0.00036659114583333335217474324707609*sin(3.0*t2 + t3 + t4) + 0.29875*L3^2*sin(t2 + t3 + t4) + 0.149375*L3^2*sin(t2 + t3 + t4 - 2.0*t5) + 0.149375*L3^2*sin(t2 + t3 + t4 + 2.0*t5) + 83.94875*L3*sin(t2 + t3 + t4 + t5) + 83.94875*L3*sin(t2 + t3 + t4 - 1.0*t5)) + td3*(0.5975*cos(t5)*sin(t5)*L3^2 + 449.32*cos(t5)*sin(t4)*L3) + td2*(0.00036659114583333335217474324707609*sin(3.0*t2 - 1.0*t1 + t3 + t4) + 0.00073318229166666670434948649415219*sin(t2 - 2.0*t1 + 3.0*t3 + t4) - 0.00018329557291666667608737162353805*sin(3.0*t2 - 2.0*t1 + t3 + t4) + 0.00018329557291666667608737162353805*sin(2.0*t1 + 3.0*t2 + t3 + t4) - 0.00036659114583333335217474324707609*sin(t1 - 1.0*t2 + t3 + t4) - 0.00036659114583333335217474324707609*sin(t1 + 3.0*t2 + t3 + t4) - 0.00018329557291666667608737162353805*sin(2.0*t1 + t2 - 1.0*t3 - 1.0*t4) - 0.00036659114583333335217474324707609*sin(t1 + t2 - 1.0*t3 - 1.0*t4) + 0.00073318229166666670434948649415219*sin(2.0*t1 + t2 - 1.0*t3 + t4) - 0.00018329557291666667608737162353805*sin(2.0*t1 - 1.0*t2 + t3 + t4) + 121.89*L3*sin(t3 + t4 - 1.0*t5) + 121.89*L3*sin(t3 + t4 + t5) + 449.32*L3*cos(t5)*sin(t4) + 0.5975*L3^2*cos(t5)*sin(t5) + 243.78*L3*cos(t3)*cos(t5)*sin(t4) + 243.78*L3*cos(t4)*cos(t5)*sin(t3)) + td4*(0.00073318229166666670434948649415219*sin(t2 - 2.0*t1 + 3.0*t3 + t4) + 0.00073318229166666670434948649415219*sin(2.0*t1 + t2 - 1.0*t3 + t4) - 112.33*L3*sin(t4 - 1.0*t5) - 112.33*L3*sin(t4 + t5) + 224.66*L3*cos(t5)*sin(t4) + 0.5975*L3^2*cos(t5)*sin(t5)) - 1.0*td6*(0.00042011718750000002619432448724979*sin(t5) + 0.00042011718750000002619432448724979*cos(t1)^2*sin(t5) + 0.00063017578125000003929148673087468*cos(2.0*t2)*cos(2.0*t3)*cos(2.0*t4)*sin(t5) - 0.00063017578125000003929148673087468*cos(2.0*t2)*sin(2.0*t3)*sin(2.0*t4)*sin(t5) - 0.00063017578125000003929148673087468*cos(2.0*t3)*sin(2.0*t2)*sin(2.0*t4)*sin(t5) - 0.00063017578125000003929148673087468*cos(2.0*t4)*sin(2.0*t2)*sin(2.0*t3)*sin(t5) - 0.00021005859375000001309716224362489*cos(2.0*t1)*cos(2.0*t2)*cos(2.0*t3)*cos(2.0*t4)*sin(t5) + 0.00021005859375000001309716224362489*cos(2.0*t1)*cos(2.0*t2)*sin(2.0*t3)*sin(2.0*t4)*sin(t5) + 0.00021005859375000001309716224362489*cos(2.0*t1)*cos(2.0*t3)*sin(2.0*t2)*sin(2.0*t4)*sin(t5) + 0.00021005859375000001309716224362489*cos(2.0*t1)*cos(2.0*t4)*sin(2.0*t2)*sin(2.0*t3)*sin(t5) - 0.00021005859375000001309716224362489*sin(2.0*t1)*cos(t2)*cos(t3)*cos(t4)*cos(t5) + 0.00021005859375000001309716224362489*sin(2.0*t1)*cos(t2)*cos(t5)*sin(t3)*sin(t4) + 0.00021005859375000001309716224362489*sin(2.0*t1)*cos(t3)*cos(t5)*sin(t2)*sin(t4) + 0.00021005859375000001309716224362489*sin(2.0*t1)*cos(t4)*cos(t5)*sin(t2)*sin(t3) + 0.00042011718750000002619432448724979*cos(t1)*cos(t2)*cos(t3)*cos(t4)*cos(t5)*sin(t1) - 0.00042011718750000002619432448724979*cos(t1)*cos(t2)*cos(t5)*sin(t1)*sin(t3)*sin(t4) - 0.00042011718750000002619432448724979*cos(t1)*cos(t3)*cos(t5)*sin(t1)*sin(t2)*sin(t4) - 0.00042011718750000002619432448724979*cos(t1)*cos(t4)*cos(t5)*sin(t1)*sin(t2)*sin(t3))) + td6*(td1*(0.00084023437500000005238864897449957*cos(t1)*cos(t5)*sin(t1) + 0.00042011718750000002619432448724979*cos(t1)^2*cos(t2)*cos(t3)*cos(t4)*sin(t5) - 0.00042011718750000002619432448724979*cos(t2)*cos(t3)*cos(t4)*sin(t1)^2*sin(t5) - 0.00042011718750000002619432448724979*cos(t1)^2*cos(t2)*sin(t3)*sin(t4)*sin(t5) - 0.00042011718750000002619432448724979*cos(t1)^2*cos(t3)*sin(t2)*sin(t4)*sin(t5) - 0.00042011718750000002619432448724979*cos(t1)^2*cos(t4)*sin(t2)*sin(t3)*sin(t5) + 0.00042011718750000002619432448724979*cos(t2)*sin(t1)^2*sin(t3)*sin(t4)*sin(t5) + 0.00042011718750000002619432448724979*cos(t3)*sin(t1)^2*sin(t2)*sin(t4)*sin(t5) + 0.00042011718750000002619432448724979*cos(t4)*sin(t1)^2*sin(t2)*sin(t3)*sin(t5)) + td6*(0.5*(0.00084023437500000005238864897449957*cos(t1)*cos(t2)*cos(t3)*sin(t4)*sin(t5) + 0.00084023437500000005238864897449957*cos(t1)*cos(t2)*cos(t4)*sin(t3)*sin(t5) + 0.00084023437500000005238864897449957*cos(t1)*cos(t3)*cos(t4)*sin(t2)*sin(t5) - 0.00084023437500000005238864897449957*cos(t1)*sin(t2)*sin(t3)*sin(t4)*sin(t5))*(cos(t1)*cos(t2)*sin(t3)*sin(t4)*sin(t5) - 1.0*cos(t1)*cos(t2)*cos(t3)*cos(t4)*sin(t5) - 1.0*cos(t5)*sin(t1) + cos(t1)*cos(t3)*sin(t2)*sin(t4)*sin(t5) + cos(t1)*cos(t4)*sin(t2)*sin(t3)*sin(t5)) + 0.5*(cos(t1)*cos(t2)*cos(t3)*sin(t4)*sin(t5) + cos(t1)*cos(t2)*cos(t4)*sin(t3)*sin(t5) + cos(t1)*cos(t3)*cos(t4)*sin(t2)*sin(t5) - 1.0*cos(t1)*sin(t2)*sin(t3)*sin(t4)*sin(t5))*(0.00084023437500000005238864897449957*cos(t1)*cos(t2)*sin(t3)*sin(t4)*sin(t5) - 0.00084023437500000005238864897449957*cos(t1)*cos(t2)*cos(t3)*cos(t4)*sin(t5) - 0.00084023437500000005238864897449957*cos(t5)*sin(t1) + 0.00084023437500000005238864897449957*cos(t1)*cos(t3)*sin(t2)*sin(t4)*sin(t5) + 0.00084023437500000005238864897449957*cos(t1)*cos(t4)*sin(t2)*sin(t3)*sin(t5)) + 0.5*(0.0016804687500000001047772979489991*cos(t2)*cos(t3)*sin(t1)*sin(t4)*sin(t5) + 0.0016804687500000001047772979489991*cos(t2)*cos(t4)*sin(t1)*sin(t3)*sin(t5) + 0.0016804687500000001047772979489991*cos(t3)*cos(t4)*sin(t1)*sin(t2)*sin(t5) - 0.0016804687500000001047772979489991*sin(t1)*sin(t2)*sin(t3)*sin(t4)*sin(t5))*(cos(t1)*cos(t5) - 1.0*cos(t2)*cos(t3)*cos(t4)*sin(t1)*sin(t5) + cos(t2)*sin(t1)*sin(t3)*sin(t4)*sin(t5) + cos(t3)*sin(t1)*sin(t2)*sin(t4)*sin(t5) + cos(t4)*sin(t1)*sin(t2)*sin(t3)*sin(t5)) + 0.5*(cos(t2)*cos(t3)*sin(t1)*sin(t4)*sin(t5) + cos(t2)*cos(t4)*sin(t1)*sin(t3)*sin(t5) + cos(t3)*cos(t4)*sin(t1)*sin(t2)*sin(t5) - 1.0*sin(t1)*sin(t2)*sin(t3)*sin(t4)*sin(t5))*(0.0016804687500000001047772979489991*cos(t1)*cos(t5) - 0.0016804687500000001047772979489991*cos(t2)*cos(t3)*cos(t4)*sin(t1)*sin(t5) + 0.0016804687500000001047772979489991*cos(t2)*sin(t1)*sin(t3)*sin(t4)*sin(t5) + 0.0016804687500000001047772979489991*cos(t3)*sin(t1)*sin(t2)*sin(t4)*sin(t5) + 0.0016804687500000001047772979489991*cos(t4)*sin(t1)*sin(t2)*sin(t3)*sin(t5))) - 1.0*td5*(0.00063017578125000003929148673087468*cos(2.0*t2)*cos(2.0*t3)*cos(2.0*t4)*sin(t5) - 0.00042011718750000002619432448724979*cos(t1)^2*sin(t5) - 0.00042011718750000002619432448724979*sin(t5) - 0.00063017578125000003929148673087468*cos(2.0*t2)*sin(2.0*t3)*sin(2.0*t4)*sin(t5) - 0.00063017578125000003929148673087468*cos(2.0*t3)*sin(2.0*t2)*sin(2.0*t4)*sin(t5) - 0.00063017578125000003929148673087468*cos(2.0*t4)*sin(2.0*t2)*sin(2.0*t3)*sin(t5) - 0.00021005859375000001309716224362489*cos(2.0*t1)*cos(2.0*t2)*cos(2.0*t3)*cos(2.0*t4)*sin(t5) + 0.00021005859375000001309716224362489*cos(2.0*t1)*cos(2.0*t2)*sin(2.0*t3)*sin(2.0*t4)*sin(t5) + 0.00021005859375000001309716224362489*cos(2.0*t1)*cos(2.0*t3)*sin(2.0*t2)*sin(2.0*t4)*sin(t5) + 0.00021005859375000001309716224362489*cos(2.0*t1)*cos(2.0*t4)*sin(2.0*t2)*sin(2.0*t3)*sin(t5) - 0.00021005859375000001309716224362489*sin(2.0*t1)*cos(t2)*cos(t3)*cos(t4)*cos(t5) + 0.00021005859375000001309716224362489*sin(2.0*t1)*cos(t2)*cos(t5)*sin(t3)*sin(t4) + 0.00021005859375000001309716224362489*sin(2.0*t1)*cos(t3)*cos(t5)*sin(t2)*sin(t4) + 0.00021005859375000001309716224362489*sin(2.0*t1)*cos(t4)*cos(t5)*sin(t2)*sin(t3) - 0.00042011718750000002619432448724979*cos(t1)*cos(t2)*cos(t3)*cos(t4)*cos(t5)*sin(t1) + 0.00042011718750000002619432448724979*cos(t1)*cos(t2)*cos(t5)*sin(t1)*sin(t3)*sin(t4) + 0.00042011718750000002619432448724979*cos(t1)*cos(t3)*cos(t5)*sin(t1)*sin(t2)*sin(t4) + 0.00042011718750000002619432448724979*cos(t1)*cos(t4)*cos(t5)*sin(t1)*sin(t2)*sin(t3))) - td2*(1.0*td3*(0.0029327291666666668173979459766088*cos(t2)*sin(t2) - 0.0029327291666666668173979459766088*cos(t1)^2*cos(t2)*sin(t2)) - td6*(0.00084023437500000005238864897449957*cos(t1)*cos(t2)*cos(t3)*sin(t1)*sin(t4)*sin(t5) + 0.00084023437500000005238864897449957*cos(t1)*cos(t2)*cos(t4)*sin(t1)*sin(t3)*sin(t5) + 0.00084023437500000005238864897449957*cos(t1)*cos(t3)*cos(t4)*sin(t1)*sin(t2)*sin(t5) - 0.00084023437500000005238864897449957*cos(t1)*sin(t1)*sin(t2)*sin(t3)*sin(t4)*sin(t5)) - td1*(68837.975*sin(t2 + t3 + t4) + 0.00073318229166666670434948649415219*sin(t1 - 2.0*t2) + 0.00073318229166666670434948649415219*sin(t1 + 2.0*t2) + 461188.44*sin(t2 + t3) + 0.0048796714583333336643505839802515*cos(t1)*sin(t1) + 0.149375*L3^2*sin(t2 + t3 + t4 - 2.0*t5) - 0.149375*L3^2*sin(t2 + t3 + t4 + 2.0*t5) - 22.705*L3*sin(t2 + t3 + t4 + t5) - 1485.2*L1*sin(t2 + t3) + 224.66*L3*sin(t2 + t3 - 1.0*t5) + 224.66*L3*sin(t2 + t3 + t5) - 335.795*L4*sin(t2 + t3 + t4) + 145.1925*L3*sin(t2 + t3 + t4 - 1.0*t5) - 0.5975*L3*L4*sin(t2 + t3 + t4 - 1.0*t5) - 0.0029327291666666668173979459766088*cos(t1)*cos(t2)^2*sin(t1) - 0.0058654583333333336347958919532175*cos(t1)*cos(t3)^2*sin(t1) + 0.0029327291666666668173979459766088*cos(t1)^2*cos(t3)*sin(t3) - 0.0029327291666666668173979459766088*cos(t3)*sin(t1)^2*sin(t3) - 0.5975*L3*L4*sin(t2 + t3 + t4 + t5)) + 1.0*td2*(1339251.84*sin(t3) + 0.0029327291666666668173979459766088*cos(t3)*sin(t3) + 199899.6*cos(t3)*sin(t4) + 199899.6*cos(t4)*sin(t3) + 0.0029327291666666668173979459766088*cos(t1)*cos(t3)^2*sin(t1) - 0.0058654583333333336347958919532175*cos(t1)^2*cos(t3)*sin(t3) - 0.0029327291666666668173979459766088*cos(t1)*sin(t1)*sin(t3)^2 - 975.12*L4*cos(t3)*sin(t4) - 975.12*L4*cos(t4)*sin(t3) - 487.56*L3*cos(t3)*cos(t4)*sin(t5) + 487.56*L3*sin(t3)*sin(t4)*sin(t5)) + 1.0*td5*(0.00073318229166666670434948649415219*sin(3.0*t2 - 1.0*t1 + t3 + t4) - 0.0014663645833333334086989729883044*sin(t2 - 2.0*t1 + 3.0*t3 + t4) - 0.00036659114583333335217474324707609*sin(3.0*t2 - 2.0*t1 + t3 + t4) + 0.00036659114583333335217474324707609*sin(2.0*t1 + 3.0*t2 + t3 + t4) + 0.00057664973958333336527190549070099*sin(t2 - 2.0*t1 + t3 + t4) - 0.00057664973958333336527190549070099*sin(2.0*t1 + t2 + t3 + t4) - 0.00073318229166666670434948649415219*sin(t1 + 3.0*t2 + t3 + t4) - 121.89*L3*sin(t3 + t4 - 1.0*t5) - 121.89*L3*sin(t3 + t4 + t5) + 449.32*L3*cos(t5)*sin(t4) + 0.5975*L3^2*cos(t5)*sin(t5) + 243.78*L3*cos(t3)*cos(t5)*sin(t4) + 243.78*L3*cos(t4)*cos(t5)*sin(t3)) - td4*(0.0029327291666666668173979459766088*cos(t2)*sin(t2)*cos(t1)^2 - 0.0014663645833333334086989729883044*sin(2.0*t1)*cos(t3)^2 + 0.0029327291666666668173979459766088*cos(2.0*t1)*cos(t3)*sin(t3) + 0.0014663645833333334086989729883044*sin(2.0*t1)*sin(t3)^2 + 184221.2*sin(t4) - 0.0029327291666666668173979459766088*cos(t2)*sin(t2) - 898.64*L4*sin(t4) - 449.32*L3*cos(t4)*sin(t5))) - td1*(1.0*td6*(0.00084023437500000005238864897449957*cos(t1)*cos(t5)*sin(t1) + 0.00042011718750000002619432448724979*cos(t1)^2*cos(t2)*cos(t3)*cos(t4)*sin(t5) - 0.00042011718750000002619432448724979*cos(t2)*cos(t3)*cos(t4)*sin(t1)^2*sin(t5) - 0.00042011718750000002619432448724979*cos(t1)^2*cos(t2)*sin(t3)*sin(t4)*sin(t5) - 0.00042011718750000002619432448724979*cos(t1)^2*cos(t3)*sin(t2)*sin(t4)*sin(t5) - 0.00042011718750000002619432448724979*cos(t1)^2*cos(t4)*sin(t2)*sin(t3)*sin(t5) + 0.00042011718750000002619432448724979*cos(t2)*sin(t1)^2*sin(t3)*sin(t4)*sin(t5) + 0.00042011718750000002619432448724979*cos(t3)*sin(t1)^2*sin(t2)*sin(t4)*sin(t5) + 0.00042011718750000002619432448724979*cos(t4)*sin(t1)^2*sin(t2)*sin(t3)*sin(t5)) - td1*(25109.9375*sin(2.0*t2 + 2.0*t3 + 2.0*t4) + 669625.92*sin(2.0*t2 + t3) + 184221.2*sin(2.0*t2 + 2.0*t3 + t4) - 99949.8*sin(t3 + t4) + 99949.8*sin(2.0*t2 + t3 + t4) - 669625.92*sin(t3) + 617106.24*sin(2.0*t2 + 2.0*t3) - 0.149375*L3^2*sin(2.0*t2 + 2.0*t3 + 2.0*t4) + 1.195*L4^2*sin(2.0*t2 + 2.0*t3 + 2.0*t4) - 898.64*L4*sin(2.0*t2 + 2.0*t3 + t4) + 0.0746875*L3^2*sin(2.0*t2 + 2.0*t3 + 2.0*t4 - 2.0*t5) + 0.0746875*L3^2*sin(2.0*t2 + 2.0*t3 + 2.0*t4 + 2.0*t5) + 224.66*L3*sin(2.0*t2 + 2.0*t3 + t4 - 1.0*t5) - 61.24375*L3*sin(2.0*t2 + 2.0*t3 + 2.0*t4 + t5) + 487.56*L4*sin(t3 + t4) - 487.56*L4*sin(2.0*t2 + t3 + t4) - 121.89*L3*sin(t3 + t4 - 1.0*t5) + 121.89*L3*sin(2.0*t2 + t3 + t4 - 1.0*t5) - 224.66*L3*sin(2.0*t2 + 2.0*t3 + t4 + t5) - 244.975*L4*sin(2.0*t2 + 2.0*t3 + 2.0*t4) + 61.24375*L3*sin(2.0*t2 + 2.0*t3 + 2.0*t4 - 1.0*t5) + 121.89*L3*sin(t3 + t4 + t5) - 121.89*L3*sin(2.0*t2 + t3 + t4 + t5) - 0.5975*L3*L4*sin(2.0*t2 + 2.0*t3 + 2.0*t4 - 1.0*t5) + 0.5975*L3*L4*sin(2.0*t2 + 2.0*t3 + 2.0*t4 + t5)) - td3*(- 0.0029327291666666668173979459766088*sin(t3)*cos(t1)^2*cos(t3) + 0.0029327291666666668173979459766088*cos(t1)*cos(t2)^2*sin(t1) + 0.0058654583333333336347958919532175*cos(t1)*cos(t3)^2*sin(t1) - 0.0048796714583333336643505839802515*cos(t1)*sin(t1) + 0.0029327291666666668173979459766088*sin(t3)*cos(t3)*sin(t1)^2) + td5*(0.00073318229166666670434948649415219*sin(t2 - 2.0*t1 + 3.0*t3 + t4) + 0.00018329557291666667608737162353805*sin(3.0*t2 - 2.0*t1 + t3 + t4) + 0.00018329557291666667608737162353805*sin(2.0*t1 + 3.0*t2 + t3 + t4) + 0.00073318229166666670434948649415219*sin(t2 + t3 + t4) - 0.00057664973958333336527190549070099*sin(t2 - 2.0*t1 + t3 + t4) - 0.00057664973958333336527190549070099*sin(2.0*t1 + t2 + t3 + t4) - 0.00018329557291666667608737162353805*sin(2.0*t1 + t2 - 1.0*t3 - 1.0*t4) - 0.00036659114583333335217474324707609*sin(t3 - 1.0*t2 + t4) + 0.00073318229166666670434948649415219*sin(2.0*t1 + t2 - 1.0*t3 + t4) + 0.00018329557291666667608737162353805*sin(2.0*t1 - 1.0*t2 + t3 + t4) - 0.00036659114583333335217474324707609*sin(3.0*t2 + t3 + t4) + 0.29875*L3^2*sin(t2 + t3 + t4) - 0.149375*L3^2*sin(t2 + t3 + t4 - 2.0*t5) - 0.149375*L3^2*sin(t2 + t3 + t4 + 2.0*t5) + 61.24375*L3*sin(t2 + t3 + t4 + t5) - 224.66*L3*sin(t2 + t3 - 1.0*t5) + 224.66*L3*sin(t2 + t3 + t5) - 61.24375*L3*sin(t2 + t3 + t4 - 1.0*t5) + 0.5975*L3*L4*sin(t2 + t3 + t4 - 1.0*t5) - 0.5975*L3*L4*sin(t2 + t3 + t4 + t5)) - td4*(- 0.0029327291666666668173979459766088*sin(t3)*cos(t1)^2*cos(t3) + 0.0029327291666666668173979459766088*cos(t1)*cos(t2)^2*sin(t1) + 0.0058654583333333336347958919532175*cos(t1)*cos(t3)^2*sin(t1) - 0.0067056927083333336871845409277171*cos(t1)*sin(t1) + 0.0029327291666666668173979459766088*sin(t3)*cos(t3)*sin(t1)^2) + 1.0*td2*(0.0029327291666666668173979459766088*sin(t3)*cos(t1)^2*cos(t3) - 0.0029327291666666668173979459766088*cos(t1)*cos(t2)^2*sin(t1) - 0.0058654583333333336347958919532175*cos(t1)*cos(t3)^2*sin(t1) + 0.0048796714583333336643505839802515*cos(t1)*sin(t1) - 0.0029327291666666668173979459766088*sin(t3)*cos(t3)*sin(t1)^2 + 0.00073318229166666670434948649415219*sin(t1 - 2.0*t2) + 0.00073318229166666670434948649415219*sin(t1 + 2.0*t2))) + td4*(td2*(0.0029327291666666668173979459766088*cos(t2)*sin(t2) - 0.0014663645833333334086989729883044*sin(2.0*t1)*cos(t3)^2 - 184221.2*sin(t4) - 199899.6*cos(t3)*sin(t4) - 199899.6*cos(t4)*sin(t3) + 0.0014663645833333334086989729883044*sin(2.0*t1)*sin(t3)^2 + 898.64*L4*sin(t4) - 0.0029327291666666668173979459766088*cos(t1)^2*cos(t2)*sin(t2) + 975.12*L4*cos(t3)*sin(t4) + 975.12*L4*cos(t4)*sin(t3) + 449.32*L3*cos(t4)*sin(t5) + 0.0029327291666666668173979459766088*cos(2.0*t1)*cos(t3)*sin(t3) + 487.56*L3*cos(t3)*cos(t4)*sin(t5) - 487.56*L3*sin(t3)*sin(t4)*sin(t5)) - 1.0*td1*(0.149375*L3^2*sin(t2 + t3 + t4 + 2.0*t5) - 0.0067056927083333336871845409277171*cos(t1)*sin(t1) - 0.149375*L3^2*sin(t2 + t3 + t4 - 2.0*t5) - 68837.975*sin(t2 + t3 + t4) + 22.705*L3*sin(t2 + t3 + t4 + t5) + 335.795*L4*sin(t2 + t3 + t4) - 145.1925*L3*sin(t2 + t3 + t4 - 1.0*t5) + 0.5975*L3*L4*sin(t2 + t3 + t4 - 1.0*t5) + 0.0029327291666666668173979459766088*cos(t1)*cos(t2)^2*sin(t1) + 0.0058654583333333336347958919532175*cos(t1)*cos(t3)^2*sin(t1) - 0.0029327291666666668173979459766088*cos(t1)^2*cos(t3)*sin(t3) + 0.0029327291666666668173979459766088*cos(t3)*sin(t1)^2*sin(t3) + 0.5975*L3*L4*sin(t2 + t3 + t4 + t5)) + td6*(0.00084023437500000005238864897449957*cos(t1)*cos(t2)*cos(t3)*sin(t1)*sin(t4)*sin(t5) + 0.00084023437500000005238864897449957*cos(t1)*cos(t2)*cos(t4)*sin(t1)*sin(t3)*sin(t5) + 0.00084023437500000005238864897449957*cos(t1)*cos(t3)*cos(t4)*sin(t1)*sin(t2)*sin(t5) - 0.00084023437500000005238864897449957*cos(t1)*sin(t1)*sin(t2)*sin(t3)*sin(t4)*sin(t5)) + td4*(0.0014663645833333334086989729883044*cos(2.0*t1)*sin(2.0*t3) - 0.0014663645833333334086989729883044*cos(2.0*t3)*sin(2.0*t1)) + td3*(898.64*L4*sin(t4) - 184221.2*sin(t4) + 449.32*L3*cos(t4)*sin(t5)) - 1.0*td5*(0.00036659114583333335217474324707609*sin(3.0*t2 - 1.0*t1 + t3 + t4) - 0.0014663645833333334086989729883044*sin(t2 - 2.0*t1 + 3.0*t3 + t4) - 0.00018329557291666667608737162353805*sin(3.0*t2 - 2.0*t1 + t3 + t4) + 0.00018329557291666667608737162353805*sin(2.0*t1 + 3.0*t2 + t3 + t4) + 0.00036659114583333335217474324707609*sin(t1 - 1.0*t2 + t3 + t4) + 0.00057664973958333336527190549070099*sin(t2 - 2.0*t1 + t3 + t4) - 0.00057664973958333336527190549070099*sin(2.0*t1 + t2 + t3 + t4) - 0.00036659114583333335217474324707609*sin(t1 + 3.0*t2 + t3 + t4) + 0.00018329557291666667608737162353805*sin(2.0*t1 + t2 - 1.0*t3 - 1.0*t4) + 0.00036659114583333335217474324707609*sin(t1 + t2 - 1.0*t3 - 1.0*t4) + 0.00018329557291666667608737162353805*sin(2.0*t1 - 1.0*t2 + t3 + t4) - 112.33*L3*sin(t4 - 1.0*t5) - 112.33*L3*sin(t4 + t5) + 224.66*L3*cos(t5)*sin(t4) + 0.5975*L3^2*cos(t5)*sin(t5))) - td3*(1.0*td2*(1339251.84*sin(t3) - 0.0029327291666666668173979459766088*cos(t2)*sin(t2) + 0.0058654583333333336347958919532175*cos(t3)*sin(t3) + 199899.6*cos(t3)*sin(t4) + 199899.6*cos(t4)*sin(t3) + 0.0058654583333333336347958919532175*cos(t1)*cos(t3)^2*sin(t1) + 0.0029327291666666668173979459766088*cos(t1)^2*cos(t2)*sin(t2) - 0.011730916666666667269591783906435*cos(t1)^2*cos(t3)*sin(t3) - 0.0058654583333333336347958919532175*cos(t1)*sin(t1)*sin(t3)^2 - 975.12*L4*cos(t3)*sin(t4) - 975.12*L4*cos(t4)*sin(t3) - 487.56*L3*cos(t3)*cos(t4)*sin(t5) + 487.56*L3*sin(t3)*sin(t4)*sin(t5)) + 1.0*td5*(0.5975*cos(t5)*sin(t5)*L3^2 + 449.32*cos(t5)*sin(t4)*L3 + 0.00036659114583333335217474324707609*sin(3.0*t2 - 1.0*t1 + t3 + t4) - 0.0021995468750000001130484594824566*sin(t2 - 2.0*t1 + 3.0*t3 + t4) - 0.00018329557291666667608737162353805*sin(3.0*t2 - 2.0*t1 + t3 + t4) + 0.00018329557291666667608737162353805*sin(2.0*t1 + 3.0*t2 + t3 + t4) + 0.00036659114583333335217474324707609*sin(t1 - 1.0*t2 + t3 + t4) + 0.00057664973958333336527190549070099*sin(t2 - 2.0*t1 + t3 + t4) - 0.00057664973958333336527190549070099*sin(2.0*t1 + t2 + t3 + t4) - 0.00036659114583333335217474324707609*sin(t1 + 3.0*t2 + t3 + t4) + 0.00018329557291666667608737162353805*sin(2.0*t1 + t2 - 1.0*t3 - 1.0*t4) + 0.00036659114583333335217474324707609*sin(t1 + t2 - 1.0*t3 - 1.0*t4) - 0.00073318229166666670434948649415219*sin(2.0*t1 + t2 - 1.0*t3 + t4) + 0.00018329557291666667608737162353805*sin(2.0*t1 - 1.0*t2 + t3 + t4)) + 1.0*td4*(- 0.011730916666666667269591783906435*cos(t1)^2*cos(t3)*sin(t3) + 0.0058654583333333336347958919532175*sin(t1)*cos(t1)*cos(t3)^2 - 0.0058654583333333336347958919532175*sin(t1)*cos(t1)*sin(t3)^2 + 0.0058654583333333336347958919532175*cos(t3)*sin(t3) - 184221.2*sin(t4) + 898.64*L4*sin(t4) + 449.32*L3*cos(t4)*sin(t5)) - td6*(0.00084023437500000005238864897449957*cos(t1)*cos(t2)*cos(t3)*sin(t1)*sin(t4)*sin(t5) + 0.00084023437500000005238864897449957*cos(t1)*cos(t2)*cos(t4)*sin(t1)*sin(t3)*sin(t5) + 0.00084023437500000005238864897449957*cos(t1)*cos(t3)*cos(t4)*sin(t1)*sin(t2)*sin(t5) - 0.00084023437500000005238864897449957*cos(t1)*sin(t1)*sin(t2)*sin(t3)*sin(t4)*sin(t5)) + 1.0*td1*(0.149375*L3^2*sin(t2 + t3 + t4 + 2.0*t5) - 461188.44*sin(t2 + t3) - 0.0048796714583333336643505839802515*cos(t1)*sin(t1) - 0.149375*L3^2*sin(t2 + t3 + t4 - 2.0*t5) - 68837.975*sin(t2 + t3 + t4) + 22.705*L3*sin(t2 + t3 + t4 + t5) + 1485.2*L1*sin(t2 + t3) - 224.66*L3*sin(t2 + t3 - 1.0*t5) - 224.66*L3*sin(t2 + t3 + t5) + 335.795*L4*sin(t2 + t3 + t4) - 145.1925*L3*sin(t2 + t3 + t4 - 1.0*t5) + 0.5975*L3*L4*sin(t2 + t3 + t4 - 1.0*t5) + 0.0029327291666666668173979459766088*cos(t1)*cos(t2)^2*sin(t1) + 0.0058654583333333336347958919532175*cos(t1)*cos(t3)^2*sin(t1) - 0.0029327291666666668173979459766088*cos(t1)^2*cos(t3)*sin(t3) + 0.0029327291666666668173979459766088*cos(t3)*sin(t1)^2*sin(t3) + 0.5975*L3*L4*sin(t2 + t3 + t4 + t5)) + 1.0*td3*(- 0.0058654583333333336347958919532175*cos(t1)^2*cos(t3)*sin(t3) + 0.0029327291666666668173979459766088*sin(t1)*cos(t1)*cos(t3)^2 - 0.0029327291666666668173979459766088*sin(t1)*cos(t1)*sin(t3)^2 + 0.0029327291666666668173979459766088*cos(t3)*sin(t3)))
    td6*(td1*(0.00084023437500000005238864897449957*cos(t1)*cos(t5)*sin(t1) + 0.00042011718750000002619432448724979*cos(t1)^2*cos(t2)*cos(t3)*cos(t4)*sin(t5) - 0.00042011718750000002619432448724979*cos(t2)*cos(t3)*cos(t4)*sin(t1)^2*sin(t5) - 0.00042011718750000002619432448724979*cos(t1)^2*cos(t2)*sin(t3)*sin(t4)*sin(t5) - 0.00042011718750000002619432448724979*cos(t1)^2*cos(t3)*sin(t2)*sin(t4)*sin(t5) - 0.00042011718750000002619432448724979*cos(t1)^2*cos(t4)*sin(t2)*sin(t3)*sin(t5) + 0.00042011718750000002619432448724979*cos(t2)*sin(t1)^2*sin(t3)*sin(t4)*sin(t5) + 0.00042011718750000002619432448724979*cos(t3)*sin(t1)^2*sin(t2)*sin(t4)*sin(t5) + 0.00042011718750000002619432448724979*cos(t4)*sin(t1)^2*sin(t2)*sin(t3)*sin(t5)) + td6*(0.5*(0.00084023437500000005238864897449957*cos(t1)*cos(t2)*cos(t3)*sin(t4)*sin(t5) + 0.00084023437500000005238864897449957*cos(t1)*cos(t2)*cos(t4)*sin(t3)*sin(t5) + 0.00084023437500000005238864897449957*cos(t1)*cos(t3)*cos(t4)*sin(t2)*sin(t5) - 0.00084023437500000005238864897449957*cos(t1)*sin(t2)*sin(t3)*sin(t4)*sin(t5))*(cos(t1)*cos(t2)*sin(t3)*sin(t4)*sin(t5) - 1.0*cos(t1)*cos(t2)*cos(t3)*cos(t4)*sin(t5) - 1.0*cos(t5)*sin(t1) + cos(t1)*cos(t3)*sin(t2)*sin(t4)*sin(t5) + cos(t1)*cos(t4)*sin(t2)*sin(t3)*sin(t5)) + 0.5*(cos(t1)*cos(t2)*cos(t3)*sin(t4)*sin(t5) + cos(t1)*cos(t2)*cos(t4)*sin(t3)*sin(t5) + cos(t1)*cos(t3)*cos(t4)*sin(t2)*sin(t5) - 1.0*cos(t1)*sin(t2)*sin(t3)*sin(t4)*sin(t5))*(0.00084023437500000005238864897449957*cos(t1)*cos(t2)*sin(t3)*sin(t4)*sin(t5) - 0.00084023437500000005238864897449957*cos(t1)*cos(t2)*cos(t3)*cos(t4)*sin(t5) - 0.00084023437500000005238864897449957*cos(t5)*sin(t1) + 0.00084023437500000005238864897449957*cos(t1)*cos(t3)*sin(t2)*sin(t4)*sin(t5) + 0.00084023437500000005238864897449957*cos(t1)*cos(t4)*sin(t2)*sin(t3)*sin(t5)) + 0.5*(0.0016804687500000001047772979489991*cos(t2)*cos(t3)*sin(t1)*sin(t4)*sin(t5) + 0.0016804687500000001047772979489991*cos(t2)*cos(t4)*sin(t1)*sin(t3)*sin(t5) + 0.0016804687500000001047772979489991*cos(t3)*cos(t4)*sin(t1)*sin(t2)*sin(t5) - 0.0016804687500000001047772979489991*sin(t1)*sin(t2)*sin(t3)*sin(t4)*sin(t5))*(cos(t1)*cos(t5) - 1.0*cos(t2)*cos(t3)*cos(t4)*sin(t1)*sin(t5) + cos(t2)*sin(t1)*sin(t3)*sin(t4)*sin(t5) + cos(t3)*sin(t1)*sin(t2)*sin(t4)*sin(t5) + cos(t4)*sin(t1)*sin(t2)*sin(t3)*sin(t5)) + 0.5*(cos(t2)*cos(t3)*sin(t1)*sin(t4)*sin(t5) + cos(t2)*cos(t4)*sin(t1)*sin(t3)*sin(t5) + cos(t3)*cos(t4)*sin(t1)*sin(t2)*sin(t5) - 1.0*sin(t1)*sin(t2)*sin(t3)*sin(t4)*sin(t5))*(0.0016804687500000001047772979489991*cos(t1)*cos(t5) - 0.0016804687500000001047772979489991*cos(t2)*cos(t3)*cos(t4)*sin(t1)*sin(t5) + 0.0016804687500000001047772979489991*cos(t2)*sin(t1)*sin(t3)*sin(t4)*sin(t5) + 0.0016804687500000001047772979489991*cos(t3)*sin(t1)*sin(t2)*sin(t4)*sin(t5) + 0.0016804687500000001047772979489991*cos(t4)*sin(t1)*sin(t2)*sin(t3)*sin(t5))) - 1.0*td5*(0.00063017578125000003929148673087468*cos(2.0*t2)*cos(2.0*t3)*cos(2.0*t4)*sin(t5) - 0.00042011718750000002619432448724979*cos(t1)^2*sin(t5) - 0.00042011718750000002619432448724979*sin(t5) - 0.00063017578125000003929148673087468*cos(2.0*t2)*sin(2.0*t3)*sin(2.0*t4)*sin(t5) - 0.00063017578125000003929148673087468*cos(2.0*t3)*sin(2.0*t2)*sin(2.0*t4)*sin(t5) - 0.00063017578125000003929148673087468*cos(2.0*t4)*sin(2.0*t2)*sin(2.0*t3)*sin(t5) - 0.00021005859375000001309716224362489*cos(2.0*t1)*cos(2.0*t2)*cos(2.0*t3)*cos(2.0*t4)*sin(t5) + 0.00021005859375000001309716224362489*cos(2.0*t1)*cos(2.0*t2)*sin(2.0*t3)*sin(2.0*t4)*sin(t5) + 0.00021005859375000001309716224362489*cos(2.0*t1)*cos(2.0*t3)*sin(2.0*t2)*sin(2.0*t4)*sin(t5) + 0.00021005859375000001309716224362489*cos(2.0*t1)*cos(2.0*t4)*sin(2.0*t2)*sin(2.0*t3)*sin(t5) - 0.00021005859375000001309716224362489*sin(2.0*t1)*cos(t2)*cos(t3)*cos(t4)*cos(t5) + 0.00021005859375000001309716224362489*sin(2.0*t1)*cos(t2)*cos(t5)*sin(t3)*sin(t4) + 0.00021005859375000001309716224362489*sin(2.0*t1)*cos(t3)*cos(t5)*sin(t2)*sin(t4) + 0.00021005859375000001309716224362489*sin(2.0*t1)*cos(t4)*cos(t5)*sin(t2)*sin(t3) - 0.00042011718750000002619432448724979*cos(t1)*cos(t2)*cos(t3)*cos(t4)*cos(t5)*sin(t1) + 0.00042011718750000002619432448724979*cos(t1)*cos(t2)*cos(t5)*sin(t1)*sin(t3)*sin(t4) + 0.00042011718750000002619432448724979*cos(t1)*cos(t3)*cos(t5)*sin(t1)*sin(t2)*sin(t4) + 0.00042011718750000002619432448724979*cos(t1)*cos(t4)*cos(t5)*sin(t1)*sin(t2)*sin(t3))) + td5*(td2*(0.00036659114583333335217474324707609*sin(3.0*t2 - 1.0*t1 + t3 + t4) - 0.00018329557291666667608737162353805*sin(3.0*t2 - 2.0*t1 + t3 + t4) + 0.00018329557291666667608737162353805*sin(2.0*t1 + 3.0*t2 + t3 + t4) - 0.00036659114583333335217474324707609*sin(t1 - 1.0*t2 + t3 + t4) - 0.00036659114583333335217474324707609*sin(t1 + 3.0*t2 + t3 + t4) - 0.00018329557291666667608737162353805*sin(2.0*t1 + t2 - 1.0*t3 - 1.0*t4) - 0.00036659114583333335217474324707609*sin(t1 + t2 - 1.0*t3 - 1.0*t4) - 0.00018329557291666667608737162353805*sin(2.0*t1 - 1.0*t2 + t3 + t4) + 112.33*L3*sin(t4 - 1.0*t5) + 112.33*L3*sin(t4 + t5) + 121.89*L3*sin(t3 + t4 - 1.0*t5) + 121.89*L3*sin(t3 + t4 + t5) + 224.66*L3*cos(t5)*sin(t4) + 0.5975*L3^2*cos(t5)*sin(t5) + 243.78*L3*cos(t3)*cos(t5)*sin(t4) + 243.78*L3*cos(t4)*cos(t5)*sin(t3)) + td5*(0.00036659114583333335217474324707609*sin(2.0*t3 - 1.0*t1 + 2.0*t4) + 0.00036659114583333335217474324707609*sin(2.0*t1 + 2.0*t2 + 2.0*t4) + 0.000091647786458333338043685811769024*sin(2.0*t3 - 2.0*t1 + 2.0*t4) + 0.000091647786458333338043685811769024*sin(2.0*t1 + 2.0*t3 + 2.0*t4) + 0.001729949218750000095815716472103*sin(2.0*t2 + 2.0*t3 + 2.0*t4) + 0.00054988671875000002826211487061414*sin(4.0*t2 + 2.0*t3 + 2.0*t4) - 0.00036659114583333335217474324707609*sin(4.0*t2 - 1.0*t1 + 2.0*t3 + 2.0*t4) - 0.00028832486979166668263595274535049*sin(2.0*t2 - 2.0*t1 + 2.0*t3 + 2.0*t4) - 0.00028832486979166668263595274535049*sin(2.0*t1 + 2.0*t2 + 2.0*t3 + 2.0*t4) + 0.00036659114583333335217474324707609*sin(2.0*t2 - 2.0*t1 + 4.0*t3 + 2.0*t4) + 0.000091647786458333338043685811769024*sin(4.0*t2 - 2.0*t1 + 2.0*t3 + 2.0*t4) + 0.000091647786458333338043685811769024*sin(2.0*t1 + 4.0*t2 + 2.0*t3 + 2.0*t4) + 0.00036659114583333335217474324707609*sin(t1 + 2.0*t3 + 2.0*t4) - 0.00036659114583333335217474324707609*sin(t1 + 4.0*t2 + 2.0*t3 + 2.0*t4) + 0.00054988671875000002826211487061414*sin(2.0*t3 + 2.0*t4)) - 1.0*td1*(0.00036659114583333335217474324707609*sin(3.0*t2 - 1.0*t1 + t3 + t4) - 0.00073318229166666670434948649415219*sin(t2 - 2.0*t1 + 3.0*t3 + t4) - 0.00018329557291666667608737162353805*sin(3.0*t2 - 2.0*t1 + t3 + t4) - 0.00018329557291666667608737162353805*sin(2.0*t1 + 3.0*t2 + t3 + t4) + 0.00073318229166666670434948649415219*sin(t2 + t3 + t4) - 0.00036659114583333335217474324707609*sin(t1 - 1.0*t2 + t3 + t4) + 0.00057664973958333336527190549070099*sin(t2 - 2.0*t1 + t3 + t4) + 0.00057664973958333336527190549070099*sin(2.0*t1 + t2 + t3 + t4) + 0.00036659114583333335217474324707609*sin(t1 + 3.0*t2 + t3 + t4) + 0.00018329557291666667608737162353805*sin(2.0*t1 + t2 - 1.0*t3 - 1.0*t4) - 0.00036659114583333335217474324707609*sin(t3 - 1.0*t2 + t4) + 0.00036659114583333335217474324707609*sin(t1 + t2 - 1.0*t3 - 1.0*t4) - 0.00073318229166666670434948649415219*sin(2.0*t1 + t2 - 1.0*t3 + t4) - 0.00018329557291666667608737162353805*sin(2.0*t1 - 1.0*t2 + t3 + t4) - 0.00036659114583333335217474324707609*sin(3.0*t2 + t3 + t4) + 0.29875*L3^2*sin(t2 + t3 + t4) + 0.149375*L3^2*sin(t2 + t3 + t4 - 2.0*t5) + 0.149375*L3^2*sin(t2 + t3 + t4 + 2.0*t5) + 83.94875*L3*sin(t2 + t3 + t4 + t5) + 83.94875*L3*sin(t2 + t3 + t4 - 1.0*t5)) + td3*(112.33*L3*sin(t4 - 1.0*t5) - 0.00073318229166666670434948649415219*sin(2.0*t1 + t2 - 1.0*t3 + t4) - 0.00073318229166666670434948649415219*sin(t2 - 2.0*t1 + 3.0*t3 + t4) + 112.33*L3*sin(t4 + t5) + 224.66*L3*cos(t5)*sin(t4) + 0.5975*L3^2*cos(t5)*sin(t5)) - 1.0*td6*(0.00042011718750000002619432448724979*sin(t5) + 0.00042011718750000002619432448724979*cos(t1)^2*sin(t5) + 0.00063017578125000003929148673087468*cos(2.0*t2)*cos(2.0*t3)*cos(2.0*t4)*sin(t5) - 0.00063017578125000003929148673087468*cos(2.0*t2)*sin(2.0*t3)*sin(2.0*t4)*sin(t5) - 0.00063017578125000003929148673087468*cos(2.0*t3)*sin(2.0*t2)*sin(2.0*t4)*sin(t5) - 0.00063017578125000003929148673087468*cos(2.0*t4)*sin(2.0*t2)*sin(2.0*t3)*sin(t5) - 0.00021005859375000001309716224362489*cos(2.0*t1)*cos(2.0*t2)*cos(2.0*t3)*cos(2.0*t4)*sin(t5) + 0.00021005859375000001309716224362489*cos(2.0*t1)*cos(2.0*t2)*sin(2.0*t3)*sin(2.0*t4)*sin(t5) + 0.00021005859375000001309716224362489*cos(2.0*t1)*cos(2.0*t3)*sin(2.0*t2)*sin(2.0*t4)*sin(t5) + 0.00021005859375000001309716224362489*cos(2.0*t1)*cos(2.0*t4)*sin(2.0*t2)*sin(2.0*t3)*sin(t5) - 0.00021005859375000001309716224362489*sin(2.0*t1)*cos(t2)*cos(t3)*cos(t4)*cos(t5) + 0.00021005859375000001309716224362489*sin(2.0*t1)*cos(t2)*cos(t5)*sin(t3)*sin(t4) + 0.00021005859375000001309716224362489*sin(2.0*t1)*cos(t3)*cos(t5)*sin(t2)*sin(t4) + 0.00021005859375000001309716224362489*sin(2.0*t1)*cos(t4)*cos(t5)*sin(t2)*sin(t3) + 0.00042011718750000002619432448724979*cos(t1)*cos(t2)*cos(t3)*cos(t4)*cos(t5)*sin(t1) - 0.00042011718750000002619432448724979*cos(t1)*cos(t2)*cos(t5)*sin(t1)*sin(t3)*sin(t4) - 0.00042011718750000002619432448724979*cos(t1)*cos(t3)*cos(t5)*sin(t1)*sin(t2)*sin(t4) - 0.00042011718750000002619432448724979*cos(t1)*cos(t4)*cos(t5)*sin(t1)*sin(t2)*sin(t3)) + 0.29875*L3^2*td4*sin(2.0*t5)) - td1*(1.0*td6*(0.00084023437500000005238864897449957*cos(t1)*cos(t5)*sin(t1) + 0.00042011718750000002619432448724979*cos(t1)^2*cos(t2)*cos(t3)*cos(t4)*sin(t5) - 0.00042011718750000002619432448724979*cos(t2)*cos(t3)*cos(t4)*sin(t1)^2*sin(t5) - 0.00042011718750000002619432448724979*cos(t1)^2*cos(t2)*sin(t3)*sin(t4)*sin(t5) - 0.00042011718750000002619432448724979*cos(t1)^2*cos(t3)*sin(t2)*sin(t4)*sin(t5) - 0.00042011718750000002619432448724979*cos(t1)^2*cos(t4)*sin(t2)*sin(t3)*sin(t5) + 0.00042011718750000002619432448724979*cos(t2)*sin(t1)^2*sin(t3)*sin(t4)*sin(t5) + 0.00042011718750000002619432448724979*cos(t3)*sin(t1)^2*sin(t2)*sin(t4)*sin(t5) + 0.00042011718750000002619432448724979*cos(t4)*sin(t1)^2*sin(t2)*sin(t3)*sin(t5)) + td5*(0.00073318229166666670434948649415219*sin(t2 - 2.0*t1 + 3.0*t3 + t4) + 0.00018329557291666667608737162353805*sin(3.0*t2 - 2.0*t1 + t3 + t4) + 0.00018329557291666667608737162353805*sin(2.0*t1 + 3.0*t2 + t3 + t4) + 0.00073318229166666670434948649415219*sin(t2 + t3 + t4) - 0.00057664973958333336527190549070099*sin(t2 - 2.0*t1 + t3 + t4) - 0.00057664973958333336527190549070099*sin(2.0*t1 + t2 + t3 + t4) - 0.00018329557291666667608737162353805*sin(2.0*t1 + t2 - 1.0*t3 - 1.0*t4) - 0.00036659114583333335217474324707609*sin(t3 - 1.0*t2 + t4) + 0.00073318229166666670434948649415219*sin(2.0*t1 + t2 - 1.0*t3 + t4) + 0.00018329557291666667608737162353805*sin(2.0*t1 - 1.0*t2 + t3 + t4) - 0.00036659114583333335217474324707609*sin(3.0*t2 + t3 + t4) + 0.29875*L3^2*sin(t2 + t3 + t4) - 0.149375*L3^2*sin(t2 + t3 + t4 - 2.0*t5) - 0.149375*L3^2*sin(t2 + t3 + t4 + 2.0*t5) + 61.24375*L3*sin(t2 + t3 + t4 + t5) - 61.24375*L3*sin(t2 + t3 + t4 - 1.0*t5) + 0.5975*L3*L4*sin(t2 + t3 + t4 - 1.0*t5) - 0.5975*L3*L4*sin(t2 + t3 + t4 + t5)) + 1.0*td4*(0.001153299479166666730543810981402*sin(2.0*t1) - 0.00073318229166666670434948649415219*cos(2.0*t2)*sin(2.0*t1) + 0.0014663645833333334086989729883044*cos(2.0*t1)*sin(2.0*t3) - 0.0014663645833333334086989729883044*cos(2.0*t3)*sin(2.0*t1)) - td3*(- 0.0029327291666666668173979459766088*sin(t3)*cos(t1)^2*cos(t3) + 0.0029327291666666668173979459766088*cos(t1)*cos(t2)^2*sin(t1) + 0.0058654583333333336347958919532175*cos(t1)*cos(t3)^2*sin(t1) - 0.0067056927083333336871845409277171*cos(t1)*sin(t1) + 0.0029327291666666668173979459766088*sin(t3)*cos(t3)*sin(t1)^2) + 1.0*td2*(- 0.0029327291666666668173979459766088*sin(2.0*t1)*cos(t3)^2 + 0.0029327291666666668173979459766088*cos(2.0*t1)*sin(t3)*cos(t3) + 0.00073318229166666670434948649415219*sin(t1 - 2.0*t2) + 0.00073318229166666670434948649415219*sin(t1 + 2.0*t2) + 0.0026196640625000001392427839697064*sin(2.0*t1) - 0.00073318229166666670434948649415219*cos(2.0*t2)*sin(2.0*t1)) - td1*(25109.9375*sin(2.0*t2 + 2.0*t3 + 2.0*t4) + 92110.6*sin(2.0*t2 + 2.0*t3 + t4) - 99949.8*sin(t3 + t4) + 99949.8*sin(2.0*t2 + t3 + t4) - 92110.6*sin(t4) - 112.33*L3*sin(t4 - 1.0*t5) - 0.149375*L3^2*sin(2.0*t2 + 2.0*t3 + 2.0*t4) + 1.195*L4^2*sin(2.0*t2 + 2.0*t3 + 2.0*t4) - 449.32*L4*sin(2.0*t2 + 2.0*t3 + t4) + 0.0746875*L3^2*sin(2.0*t2 + 2.0*t3 + 2.0*t4 - 2.0*t5) + 0.0746875*L3^2*sin(2.0*t2 + 2.0*t3 + 2.0*t4 + 2.0*t5) + 112.33*L3*sin(2.0*t2 + 2.0*t3 + t4 - 1.0*t5) - 61.24375*L3*sin(2.0*t2 + 2.0*t3 + 2.0*t4 + t5) + 487.56*L4*sin(t3 + t4) + 112.33*L3*sin(t4 + t5) - 487.56*L4*sin(2.0*t2 + t3 + t4) - 121.89*L3*sin(t3 + t4 - 1.0*t5) + 121.89*L3*sin(2.0*t2 + t3 + t4 - 1.0*t5) - 112.33*L3*sin(2.0*t2 + 2.0*t3 + t4 + t5) + 449.32*L4*sin(t4) - 244.975*L4*sin(2.0*t2 + 2.0*t3 + 2.0*t4) + 61.24375*L3*sin(2.0*t2 + 2.0*t3 + 2.0*t4 - 1.0*t5) + 121.89*L3*sin(t3 + t4 + t5) - 121.89*L3*sin(2.0*t2 + t3 + t4 + t5) - 0.5975*L3*L4*sin(2.0*t2 + 2.0*t3 + 2.0*t4 - 1.0*t5) + 0.5975*L3*L4*sin(2.0*t2 + 2.0*t3 + 2.0*t4 + t5))) + td2*(td2*(898.64*L4*sin(t4) - 199899.6*cos(t3)*sin(t4) - 199899.6*cos(t4)*sin(t3) - 184221.2*sin(t4) + 975.12*L4*cos(t3)*sin(t4) + 975.12*L4*cos(t4)*sin(t3) + 449.32*L3*cos(t4)*sin(t5) + 487.56*L3*cos(t3)*cos(t4)*sin(t5) - 487.56*L3*sin(t3)*sin(t4)*sin(t5)) - 1.0*td4*(0.00073318229166666670434948649415219*sin(2.0*t2) - 0.00073318229166666670434948649415219*cos(2.0*t1)*sin(2.0*t2)) + td1*(68837.975*sin(t2 + t3 + t4) + 0.00073318229166666670434948649415219*sin(t1 - 2.0*t2) + 0.00073318229166666670434948649415219*sin(t1 + 2.0*t2) + 0.0026196640625000001392427839697064*sin(2.0*t1) - 0.0029327291666666668173979459766088*sin(2.0*t1)*cos(t3)^2 + 0.149375*L3^2*sin(t2 + t3 + t4 - 2.0*t5) - 0.149375*L3^2*sin(t2 + t3 + t4 + 2.0*t5) - 22.705*L3*sin(t2 + t3 + t4 + t5) - 0.00073318229166666670434948649415219*cos(2.0*t2)*sin(2.0*t1) - 335.795*L4*sin(t2 + t3 + t4) + 145.1925*L3*sin(t2 + t3 + t4 - 1.0*t5) - 0.5975*L3*L4*sin(t2 + t3 + t4 - 1.0*t5) + 0.0029327291666666668173979459766088*cos(2.0*t1)*cos(t3)*sin(t3) - 0.5975*L3*L4*sin(t2 + t3 + t4 + t5)) + td6*(0.00084023437500000005238864897449957*cos(t1)*cos(t2)*cos(t3)*sin(t1)*sin(t4)*sin(t5) + 0.00084023437500000005238864897449957*cos(t1)*cos(t2)*cos(t4)*sin(t1)*sin(t3)*sin(t5) + 0.00084023437500000005238864897449957*cos(t1)*cos(t3)*cos(t4)*sin(t1)*sin(t2)*sin(t5) - 0.00084023437500000005238864897449957*cos(t1)*sin(t1)*sin(t2)*sin(t3)*sin(t4)*sin(t5)) - 1.0*td5*(0.00073318229166666670434948649415219*sin(3.0*t2 - 1.0*t1 + t3 + t4) - 0.00073318229166666670434948649415219*sin(t2 - 2.0*t1 + 3.0*t3 + t4) - 0.00036659114583333335217474324707609*sin(3.0*t2 - 2.0*t1 + t3 + t4) + 0.00036659114583333335217474324707609*sin(2.0*t1 + 3.0*t2 + t3 + t4) + 0.00057664973958333336527190549070099*sin(t2 - 2.0*t1 + t3 + t4) - 0.00057664973958333336527190549070099*sin(2.0*t1 + t2 + t3 + t4) - 0.00073318229166666670434948649415219*sin(t1 + 3.0*t2 + t3 + t4) + 0.00073318229166666670434948649415219*sin(2.0*t1 + t2 - 1.0*t3 + t4) - 112.33*L3*sin(t4 - 1.0*t5) - 112.33*L3*sin(t4 + t5) - 121.89*L3*sin(t3 + t4 - 1.0*t5) - 121.89*L3*sin(t3 + t4 + t5) + 224.66*L3*cos(t5)*sin(t4) + 0.5975*L3^2*cos(t5)*sin(t5) + 243.78*L3*cos(t3)*cos(t5)*sin(t4) + 243.78*L3*cos(t4)*cos(t5)*sin(t3)) - 1.0*td3*(- 0.0029327291666666668173979459766088*cos(t2)*sin(t2)*cos(t1)^2 - 0.0014663645833333334086989729883044*sin(2.0*t1)*cos(t3)^2 + 0.0029327291666666668173979459766088*cos(2.0*t1)*cos(t3)*sin(t3) + 0.0014663645833333334086989729883044*sin(2.0*t1)*sin(t3)^2 + 184221.2*sin(t4) + 0.0029327291666666668173979459766088*cos(t2)*sin(t2) - 898.64*L4*sin(t4) - 449.32*L3*cos(t4)*sin(t5))) + td4*(td2*(0.00073318229166666670434948649415219*sin(2.0*t2) - 184221.2*sin(t4) - 199899.6*cos(t3)*sin(t4) - 199899.6*cos(t4)*sin(t3) - 0.00073318229166666670434948649415219*cos(2.0*t1)*sin(2.0*t2) + 898.64*L4*sin(t4) + 975.12*L4*cos(t3)*sin(t4) + 975.12*L4*cos(t4)*sin(t3) + 449.32*L3*cos(t4)*sin(t5) + 487.56*L3*cos(t3)*cos(t4)*sin(t5) - 487.56*L3*sin(t3)*sin(t4)*sin(t5)) - 1.0*td1*(0.149375*L3^2*sin(t2 + t3 + t4 + 2.0*t5) - 0.001153299479166666730543810981402*sin(2.0*t1) - 0.149375*L3^2*sin(t2 + t3 + t4 - 2.0*t5) - 68837.975*sin(t2 + t3 + t4) + 22.705*L3*sin(t2 + t3 + t4 + t5) + 0.00073318229166666670434948649415219*cos(2.0*t2)*sin(2.0*t1) - 0.0014663645833333334086989729883044*cos(2.0*t1)*sin(2.0*t3) + 0.0014663645833333334086989729883044*cos(2.0*t3)*sin(2.0*t1) + 335.795*L4*sin(t2 + t3 + t4) - 145.1925*L3*sin(t2 + t3 + t4 - 1.0*t5) + 0.5975*L3*L4*sin(t2 + t3 + t4 - 1.0*t5) + 0.5975*L3*L4*sin(t2 + t3 + t4 + t5)) + td3*(0.0014663645833333334086989729883044*cos(2.0*t3)*sin(2.0*t1) - 0.0014663645833333334086989729883044*cos(2.0*t1)*sin(2.0*t3) - 184221.2*sin(t4) + 898.64*L4*sin(t4) + 449.32*L3*cos(t4)*sin(t5)) - 1.0*td5*(0.29875*sin(2.0*t5)*L3^2 + 0.00036659114583333335217474324707609*sin(3.0*t2 - 1.0*t1 + t3 + t4) - 0.00073318229166666670434948649415219*sin(t2 - 2.0*t1 + 3.0*t3 + t4) - 0.00018329557291666667608737162353805*sin(3.0*t2 - 2.0*t1 + t3 + t4) + 0.00018329557291666667608737162353805*sin(2.0*t1 + 3.0*t2 + t3 + t4) + 0.00036659114583333335217474324707609*sin(t1 - 1.0*t2 + t3 + t4) + 0.00057664973958333336527190549070099*sin(t2 - 2.0*t1 + t3 + t4) - 0.00057664973958333336527190549070099*sin(2.0*t1 + t2 + t3 + t4) - 0.00036659114583333335217474324707609*sin(t1 + 3.0*t2 + t3 + t4) + 0.00018329557291666667608737162353805*sin(2.0*t1 + t2 - 1.0*t3 - 1.0*t4) + 0.00036659114583333335217474324707609*sin(t1 + t2 - 1.0*t3 - 1.0*t4) + 0.00073318229166666670434948649415219*sin(2.0*t1 + t2 - 1.0*t3 + t4) + 0.00018329557291666667608737162353805*sin(2.0*t1 - 1.0*t2 + t3 + t4)) + td6*(0.00084023437500000005238864897449957*cos(t1)*cos(t2)*cos(t3)*sin(t1)*sin(t4)*sin(t5) + 0.00084023437500000005238864897449957*cos(t1)*cos(t2)*cos(t4)*sin(t1)*sin(t3)*sin(t5) + 0.00084023437500000005238864897449957*cos(t1)*cos(t3)*cos(t4)*sin(t1)*sin(t2)*sin(t5) - 0.00084023437500000005238864897449957*cos(t1)*sin(t1)*sin(t2)*sin(t3)*sin(t4)*sin(t5))) + td3*(td2*(0.0029327291666666668173979459766088*cos(t2)*sin(t2) - 0.0014663645833333334086989729883044*sin(2.0*t1)*cos(t3)^2 - 184221.2*sin(t4) - 199899.6*cos(t3)*sin(t4) - 199899.6*cos(t4)*sin(t3) + 0.0014663645833333334086989729883044*sin(2.0*t1)*sin(t3)^2 + 898.64*L4*sin(t4) - 0.0029327291666666668173979459766088*cos(t1)^2*cos(t2)*sin(t2) + 975.12*L4*cos(t3)*sin(t4) + 975.12*L4*cos(t4)*sin(t3) + 449.32*L3*cos(t4)*sin(t5) + 0.0029327291666666668173979459766088*cos(2.0*t1)*cos(t3)*sin(t3) + 487.56*L3*cos(t3)*cos(t4)*sin(t5) - 487.56*L3*sin(t3)*sin(t4)*sin(t5)) - 1.0*td1*(0.149375*L3^2*sin(t2 + t3 + t4 + 2.0*t5) - 0.0067056927083333336871845409277171*cos(t1)*sin(t1) - 0.149375*L3^2*sin(t2 + t3 + t4 - 2.0*t5) - 68837.975*sin(t2 + t3 + t4) + 22.705*L3*sin(t2 + t3 + t4 + t5) + 335.795*L4*sin(t2 + t3 + t4) - 145.1925*L3*sin(t2 + t3 + t4 - 1.0*t5) + 0.5975*L3*L4*sin(t2 + t3 + t4 - 1.0*t5) + 0.0029327291666666668173979459766088*cos(t1)*cos(t2)^2*sin(t1) + 0.0058654583333333336347958919532175*cos(t1)*cos(t3)^2*sin(t1) - 0.0029327291666666668173979459766088*cos(t1)^2*cos(t3)*sin(t3) + 0.0029327291666666668173979459766088*cos(t3)*sin(t1)^2*sin(t3) + 0.5975*L3*L4*sin(t2 + t3 + t4 + t5)) + td6*(0.00084023437500000005238864897449957*cos(t1)*cos(t2)*cos(t3)*sin(t1)*sin(t4)*sin(t5) + 0.00084023437500000005238864897449957*cos(t1)*cos(t2)*cos(t4)*sin(t1)*sin(t3)*sin(t5) + 0.00084023437500000005238864897449957*cos(t1)*cos(t3)*cos(t4)*sin(t1)*sin(t2)*sin(t5) - 0.00084023437500000005238864897449957*cos(t1)*sin(t1)*sin(t2)*sin(t3)*sin(t4)*sin(t5)) + td4*(0.0014663645833333334086989729883044*cos(2.0*t1)*sin(2.0*t3) - 0.0014663645833333334086989729883044*cos(2.0*t3)*sin(2.0*t1)) + td3*(898.64*L4*sin(t4) - 184221.2*sin(t4) + 449.32*L3*cos(t4)*sin(t5)) - 1.0*td5*(0.00036659114583333335217474324707609*sin(3.0*t2 - 1.0*t1 + t3 + t4) - 0.0014663645833333334086989729883044*sin(t2 - 2.0*t1 + 3.0*t3 + t4) - 0.00018329557291666667608737162353805*sin(3.0*t2 - 2.0*t1 + t3 + t4) + 0.00018329557291666667608737162353805*sin(2.0*t1 + 3.0*t2 + t3 + t4) + 0.00036659114583333335217474324707609*sin(t1 - 1.0*t2 + t3 + t4) + 0.00057664973958333336527190549070099*sin(t2 - 2.0*t1 + t3 + t4) - 0.00057664973958333336527190549070099*sin(2.0*t1 + t2 + t3 + t4) - 0.00036659114583333335217474324707609*sin(t1 + 3.0*t2 + t3 + t4) + 0.00018329557291666667608737162353805*sin(2.0*t1 + t2 - 1.0*t3 - 1.0*t4) + 0.00036659114583333335217474324707609*sin(t1 + t2 - 1.0*t3 - 1.0*t4) + 0.00018329557291666667608737162353805*sin(2.0*t1 - 1.0*t2 + t3 + t4) - 112.33*L3*sin(t4 - 1.0*t5) - 112.33*L3*sin(t4 + t5) + 224.66*L3*cos(t5)*sin(t4) + 0.5975*L3^2*cos(t5)*sin(t5)))
    td3*(td5*(0.00036659114583333335217474324707609*sin(2.0*t3 - 1.0*t1 + 2.0*t4) + 0.000091647786458333338043685811769024*sin(2.0*t3 - 2.0*t1 + 2.0*t4) + 0.000091647786458333338043685811769024*sin(2.0*t1 + 2.0*t3 + 2.0*t4) + 0.001729949218750000095815716472103*sin(2.0*t2 + 2.0*t3 + 2.0*t4) + 0.00054988671875000002826211487061414*sin(4.0*t2 + 2.0*t3 + 2.0*t4) - 0.00036659114583333335217474324707609*sin(4.0*t2 - 1.0*t1 + 2.0*t3 + 2.0*t4) - 0.00028832486979166668263595274535049*sin(2.0*t2 - 2.0*t1 + 2.0*t3 + 2.0*t4) - 0.00028832486979166668263595274535049*sin(2.0*t1 + 2.0*t2 + 2.0*t3 + 2.0*t4) + 0.00073318229166666670434948649415219*sin(2.0*t2 - 2.0*t1 + 4.0*t3 + 2.0*t4) + 0.000091647786458333338043685811769024*sin(4.0*t2 - 2.0*t1 + 2.0*t3 + 2.0*t4) + 0.000091647786458333338043685811769024*sin(2.0*t1 + 4.0*t2 + 2.0*t3 + 2.0*t4) + 0.00036659114583333335217474324707609*sin(t1 + 2.0*t3 + 2.0*t4) - 0.00036659114583333335217474324707609*sin(t1 + 4.0*t2 + 2.0*t3 + 2.0*t4) + 0.00073318229166666670434948649415219*sin(2.0*t1 - 2.0*t3) + 0.00054988671875000002826211487061414*sin(2.0*t3 + 2.0*t4)) - 1.0*td1*(0.00036659114583333335217474324707609*sin(3.0*t2 - 1.0*t1 + t3 + t4) - 0.00073318229166666670434948649415219*sin(t2 - 2.0*t1 + 3.0*t3 + t4) - 0.00018329557291666667608737162353805*sin(3.0*t2 - 2.0*t1 + t3 + t4) - 0.00018329557291666667608737162353805*sin(2.0*t1 + 3.0*t2 + t3 + t4) + 0.00073318229166666670434948649415219*sin(t2 + t3 + t4) - 0.00036659114583333335217474324707609*sin(t1 - 1.0*t2 + t3 + t4) + 0.00057664973958333336527190549070099*sin(t2 - 2.0*t1 + t3 + t4) + 0.00057664973958333336527190549070099*sin(2.0*t1 + t2 + t3 + t4) + 0.00036659114583333335217474324707609*sin(t1 + 3.0*t2 + t3 + t4) + 0.00018329557291666667608737162353805*sin(2.0*t1 + t2 - 1.0*t3 - 1.0*t4) - 0.00036659114583333335217474324707609*sin(t3 - 1.0*t2 + t4) + 0.00036659114583333335217474324707609*sin(t1 + t2 - 1.0*t3 - 1.0*t4) - 0.00073318229166666670434948649415219*sin(2.0*t1 + t2 - 1.0*t3 + t4) - 0.00018329557291666667608737162353805*sin(2.0*t1 - 1.0*t2 + t3 + t4) - 0.00036659114583333335217474324707609*sin(3.0*t2 + t3 + t4) + 0.29875*L3^2*sin(t2 + t3 + t4) + 0.149375*L3^2*sin(t2 + t3 + t4 - 2.0*t5) + 0.149375*L3^2*sin(t2 + t3 + t4 + 2.0*t5) + 83.94875*L3*sin(t2 + t3 + t4 + t5) + 83.94875*L3*sin(t2 + t3 + t4 - 1.0*t5)) + td3*(0.5975*cos(t5)*sin(t5)*L3^2 + 449.32*cos(t5)*sin(t4)*L3) + td2*(0.00036659114583333335217474324707609*sin(3.0*t2 - 1.0*t1 + t3 + t4) + 0.00073318229166666670434948649415219*sin(t2 - 2.0*t1 + 3.0*t3 + t4) - 0.00018329557291666667608737162353805*sin(3.0*t2 - 2.0*t1 + t3 + t4) + 0.00018329557291666667608737162353805*sin(2.0*t1 + 3.0*t2 + t3 + t4) - 0.00036659114583333335217474324707609*sin(t1 - 1.0*t2 + t3 + t4) - 0.00036659114583333335217474324707609*sin(t1 + 3.0*t2 + t3 + t4) - 0.00018329557291666667608737162353805*sin(2.0*t1 + t2 - 1.0*t3 - 1.0*t4) - 0.00036659114583333335217474324707609*sin(t1 + t2 - 1.0*t3 - 1.0*t4) + 0.00073318229166666670434948649415219*sin(2.0*t1 + t2 - 1.0*t3 + t4) - 0.00018329557291666667608737162353805*sin(2.0*t1 - 1.0*t2 + t3 + t4) + 121.89*L3*sin(t3 + t4 - 1.0*t5) + 121.89*L3*sin(t3 + t4 + t5) + 449.32*L3*cos(t5)*sin(t4) + 0.5975*L3^2*cos(t5)*sin(t5) + 243.78*L3*cos(t3)*cos(t5)*sin(t4) + 243.78*L3*cos(t4)*cos(t5)*sin(t3)) + td4*(0.00073318229166666670434948649415219*sin(t2 - 2.0*t1 + 3.0*t3 + t4) + 0.00073318229166666670434948649415219*sin(2.0*t1 + t2 - 1.0*t3 + t4) - 112.33*L3*sin(t4 - 1.0*t5) - 112.33*L3*sin(t4 + t5) + 224.66*L3*cos(t5)*sin(t4) + 0.5975*L3^2*cos(t5)*sin(t5)) - 1.0*td6*(0.00042011718750000002619432448724979*sin(t5) + 0.00042011718750000002619432448724979*cos(t1)^2*sin(t5) + 0.00063017578125000003929148673087468*cos(2.0*t2)*cos(2.0*t3)*cos(2.0*t4)*sin(t5) - 0.00063017578125000003929148673087468*cos(2.0*t2)*sin(2.0*t3)*sin(2.0*t4)*sin(t5) - 0.00063017578125000003929148673087468*cos(2.0*t3)*sin(2.0*t2)*sin(2.0*t4)*sin(t5) - 0.00063017578125000003929148673087468*cos(2.0*t4)*sin(2.0*t2)*sin(2.0*t3)*sin(t5) - 0.00021005859375000001309716224362489*cos(2.0*t1)*cos(2.0*t2)*cos(2.0*t3)*cos(2.0*t4)*sin(t5) + 0.00021005859375000001309716224362489*cos(2.0*t1)*cos(2.0*t2)*sin(2.0*t3)*sin(2.0*t4)*sin(t5) + 0.00021005859375000001309716224362489*cos(2.0*t1)*cos(2.0*t3)*sin(2.0*t2)*sin(2.0*t4)*sin(t5) + 0.00021005859375000001309716224362489*cos(2.0*t1)*cos(2.0*t4)*sin(2.0*t2)*sin(2.0*t3)*sin(t5) - 0.00021005859375000001309716224362489*sin(2.0*t1)*cos(t2)*cos(t3)*cos(t4)*cos(t5) + 0.00021005859375000001309716224362489*sin(2.0*t1)*cos(t2)*cos(t5)*sin(t3)*sin(t4) + 0.00021005859375000001309716224362489*sin(2.0*t1)*cos(t3)*cos(t5)*sin(t2)*sin(t4) + 0.00021005859375000001309716224362489*sin(2.0*t1)*cos(t4)*cos(t5)*sin(t2)*sin(t3) + 0.00042011718750000002619432448724979*cos(t1)*cos(t2)*cos(t3)*cos(t4)*cos(t5)*sin(t1) - 0.00042011718750000002619432448724979*cos(t1)*cos(t2)*cos(t5)*sin(t1)*sin(t3)*sin(t4) - 0.00042011718750000002619432448724979*cos(t1)*cos(t3)*cos(t5)*sin(t1)*sin(t2)*sin(t4) - 0.00042011718750000002619432448724979*cos(t1)*cos(t4)*cos(t5)*sin(t1)*sin(t2)*sin(t3))) - td5*(1.0*td6*(0.00063017578125000003929148673087468*cos(2.0*t2)*cos(2.0*t3)*sin(2.0*t4)*cos(t5) + 0.00063017578125000003929148673087468*cos(2.0*t2)*cos(2.0*t4)*sin(2.0*t3)*cos(t5) + 0.00063017578125000003929148673087468*cos(2.0*t3)*cos(2.0*t4)*sin(2.0*t2)*cos(t5) - 0.00063017578125000003929148673087468*sin(2.0*t2)*sin(2.0*t3)*sin(2.0*t4)*cos(t5) - 0.00021005859375000001309716224362489*cos(2.0*t1)*cos(2.0*t2)*cos(2.0*t3)*sin(2.0*t4)*cos(t5) - 0.00021005859375000001309716224362489*cos(2.0*t1)*cos(2.0*t2)*cos(2.0*t4)*sin(2.0*t3)*cos(t5) - 0.00021005859375000001309716224362489*cos(2.0*t1)*cos(2.0*t3)*cos(2.0*t4)*sin(2.0*t2)*cos(t5) + 0.00021005859375000001309716224362489*cos(2.0*t1)*sin(2.0*t2)*sin(2.0*t3)*sin(2.0*t4)*cos(t5) + 0.00042011718750000002619432448724979*sin(2.0*t1)*cos(t2)*cos(t3)*sin(t4)*sin(t5) + 0.00042011718750000002619432448724979*sin(2.0*t1)*cos(t2)*cos(t4)*sin(t3)*sin(t5) + 0.00042011718750000002619432448724979*sin(2.0*t1)*cos(t3)*cos(t4)*sin(t2)*sin(t5) - 0.00042011718750000002619432448724979*sin(2.0*t1)*sin(t2)*sin(t3)*sin(t4)*sin(t5)) - 1.0*td1*(0.00018329557291666667608737162353805*sin(2.0*t3 - 1.0*t1 + 2.0*t4) - 0.00036659114583333335217474324707609*sin(2.0*t1 + 2.0*t2 + 2.0*t4) + 0.000091647786458333338043685811769024*sin(2.0*t3 - 2.0*t1 + 2.0*t4) - 0.000091647786458333338043685811769024*sin(2.0*t1 + 2.0*t3 + 2.0*t4) - 0.00018329557291666667608737162353805*sin(4.0*t2 - 1.0*t1 + 2.0*t3 + 2.0*t4) - 0.00028832486979166668263595274535049*sin(2.0*t2 - 2.0*t1 + 2.0*t3 + 2.0*t4) + 0.00028832486979166668263595274535049*sin(2.0*t1 + 2.0*t2 + 2.0*t3 + 2.0*t4) + 0.00036659114583333335217474324707609*sin(2.0*t2 - 2.0*t1 + 4.0*t3 + 2.0*t4) + 0.000091647786458333338043685811769024*sin(4.0*t2 - 2.0*t1 + 2.0*t3 + 2.0*t4) - 0.000091647786458333338043685811769024*sin(2.0*t1 + 4.0*t2 + 2.0*t3 + 2.0*t4) - 0.00018329557291666667608737162353805*sin(t1 + 2.0*t3 + 2.0*t4) + 0.00018329557291666667608737162353805*sin(t1 + 4.0*t2 + 2.0*t3 + 2.0*t4) - 0.00057664973958333336527190549070099*sin(2.0*t1) + 0.00018329557291666667608737162353805*sin(2.0*t1 - 2.0*t2) + 0.00018329557291666667608737162353805*sin(2.0*t1 + 2.0*t2) + 0.00073318229166666670434948649415219*sin(2.0*t1 - 2.0*t3) - 243.78*L3*sin(t2 - 1.0*t5) - 145.1925*L3*sin(t2 + t3 + t4 + t5) - 243.78*L3*sin(t2 + t5) - 224.66*L3*sin(t2 + t3 - 1.0*t5) - 224.66*L3*sin(t2 + t3 + t5) + 22.705*L3*sin(t2 + t3 + t4 - 1.0*t5) + 0.5975*L3*L4*sin(t2 + t3 + t4 - 1.0*t5) + 0.5975*L3*L4*sin(t2 + t3 + t4 + t5)) + 1.0*td4*(0.00036659114583333335217474324707609*sin(2.0*t3 - 1.0*t1 + 2.0*t4) + 0.00036659114583333335217474324707609*sin(2.0*t1 + 2.0*t2 + 2.0*t4) + 0.000091647786458333338043685811769024*sin(2.0*t3 - 2.0*t1 + 2.0*t4) + 0.000091647786458333338043685811769024*sin(2.0*t1 + 2.0*t3 + 2.0*t4) + 0.001729949218750000095815716472103*sin(2.0*t2 + 2.0*t3 + 2.0*t4) + 0.00054988671875000002826211487061414*sin(4.0*t2 + 2.0*t3 + 2.0*t4) - 0.00036659114583333335217474324707609*sin(4.0*t2 - 1.0*t1 + 2.0*t3 + 2.0*t4) - 0.00028832486979166668263595274535049*sin(2.0*t2 - 2.0*t1 + 2.0*t3 + 2.0*t4) - 0.00028832486979166668263595274535049*sin(2.0*t1 + 2.0*t2 + 2.0*t3 + 2.0*t4) + 0.00036659114583333335217474324707609*sin(2.0*t2 - 2.0*t1 + 4.0*t3 + 2.0*t4) + 0.000091647786458333338043685811769024*sin(4.0*t2 - 2.0*t1 + 2.0*t3 + 2.0*t4) + 0.000091647786458333338043685811769024*sin(2.0*t1 + 4.0*t2 + 2.0*t3 + 2.0*t4) + 0.00036659114583333335217474324707609*sin(t1 + 2.0*t3 + 2.0*t4) - 0.00036659114583333335217474324707609*sin(t1 + 4.0*t2 + 2.0*t3 + 2.0*t4) + 0.00054988671875000002826211487061414*sin(2.0*t3 + 2.0*t4) - 122.4875*L3*sin(t5) + 1.195*L3*L4*sin(t5)) + 1.0*td2*(0.00036659114583333335217474324707609*sin(2.0*t1 + 2.0*t2 + 2.0*t4) + 0.001729949218750000095815716472103*sin(2.0*t2 + 2.0*t3 + 2.0*t4) + 0.0010997734375000000565242297412283*sin(4.0*t2 + 2.0*t3 + 2.0*t4) - 0.00073318229166666670434948649415219*sin(4.0*t2 - 1.0*t1 + 2.0*t3 + 2.0*t4) - 0.00028832486979166668263595274535049*sin(2.0*t2 - 2.0*t1 + 2.0*t3 + 2.0*t4) - 0.00028832486979166668263595274535049*sin(2.0*t1 + 2.0*t2 + 2.0*t3 + 2.0*t4) + 0.00036659114583333335217474324707609*sin(2.0*t2 - 2.0*t1 + 4.0*t3 + 2.0*t4) + 0.00018329557291666667608737162353805*sin(4.0*t2 - 2.0*t1 + 2.0*t3 + 2.0*t4) + 0.00018329557291666667608737162353805*sin(2.0*t1 + 4.0*t2 + 2.0*t3 + 2.0*t4) - 0.00073318229166666670434948649415219*sin(t1 + 4.0*t2 + 2.0*t3 + 2.0*t4) + 0.00036659114583333335217474324707609*sin(2.0*t2) + 0.00018329557291666667608737162353805*sin(2.0*t1 - 2.0*t2) - 0.00018329557291666667608737162353805*sin(2.0*t1 + 2.0*t2) + 224.66*L3*sin(t4 - 1.0*t5) - 224.66*L3*sin(t4 + t5) + 243.78*L3*sin(t3 + t4 - 1.0*t5) - 122.4875*L3*sin(t5) - 243.78*L3*sin(t3 + t4 + t5) + 1.195*L3*L4*sin(t5)) + 1.0*td3*(0.00036659114583333335217474324707609*sin(2.0*t3 - 1.0*t1 + 2.0*t4) + 0.000091647786458333338043685811769024*sin(2.0*t3 - 2.0*t1 + 2.0*t4) + 0.000091647786458333338043685811769024*sin(2.0*t1 + 2.0*t3 + 2.0*t4) + 0.001729949218750000095815716472103*sin(2.0*t2 + 2.0*t3 + 2.0*t4) + 0.00054988671875000002826211487061414*sin(4.0*t2 + 2.0*t3 + 2.0*t4) - 0.00036659114583333335217474324707609*sin(4.0*t2 - 1.0*t1 + 2.0*t3 + 2.0*t4) - 0.00028832486979166668263595274535049*sin(2.0*t2 - 2.0*t1 + 2.0*t3 + 2.0*t4) - 0.00028832486979166668263595274535049*sin(2.0*t1 + 2.0*t2 + 2.0*t3 + 2.0*t4) + 0.00073318229166666670434948649415219*sin(2.0*t2 - 2.0*t1 + 4.0*t3 + 2.0*t4) + 0.000091647786458333338043685811769024*sin(4.0*t2 - 2.0*t1 + 2.0*t3 + 2.0*t4) + 0.000091647786458333338043685811769024*sin(2.0*t1 + 4.0*t2 + 2.0*t3 + 2.0*t4) + 0.00036659114583333335217474324707609*sin(t1 + 2.0*t3 + 2.0*t4) - 0.00036659114583333335217474324707609*sin(t1 + 4.0*t2 + 2.0*t3 + 2.0*t4) + 0.00073318229166666670434948649415219*sin(2.0*t1 - 2.0*t3) + 0.00054988671875000002826211487061414*sin(2.0*t3 + 2.0*t4) + 224.66*L3*sin(t4 - 1.0*t5) - 224.66*L3*sin(t4 + t5) - 122.4875*L3*sin(t5) + 1.195*L3*L4*sin(t5))) + td4*(td2*(0.00036659114583333335217474324707609*sin(3.0*t2 - 1.0*t1 + t3 + t4) - 0.00018329557291666667608737162353805*sin(3.0*t2 - 2.0*t1 + t3 + t4) + 0.00018329557291666667608737162353805*sin(2.0*t1 + 3.0*t2 + t3 + t4) - 0.00036659114583333335217474324707609*sin(t1 - 1.0*t2 + t3 + t4) - 0.00036659114583333335217474324707609*sin(t1 + 3.0*t2 + t3 + t4) - 0.00018329557291666667608737162353805*sin(2.0*t1 + t2 - 1.0*t3 - 1.0*t4) - 0.00036659114583333335217474324707609*sin(t1 + t2 - 1.0*t3 - 1.0*t4) - 0.00018329557291666667608737162353805*sin(2.0*t1 - 1.0*t2 + t3 + t4) + 112.33*L3*sin(t4 - 1.0*t5) + 112.33*L3*sin(t4 + t5) + 121.89*L3*sin(t3 + t4 - 1.0*t5) + 121.89*L3*sin(t3 + t4 + t5) + 224.66*L3*cos(t5)*sin(t4) + 0.5975*L3^2*cos(t5)*sin(t5) + 243.78*L3*cos(t3)*cos(t5)*sin(t4) + 243.78*L3*cos(t4)*cos(t5)*sin(t3)) + td5*(0.00036659114583333335217474324707609*sin(2.0*t3 - 1.0*t1 + 2.0*t4) + 0.00036659114583333335217474324707609*sin(2.0*t1 + 2.0*t2 + 2.0*t4) + 0.000091647786458333338043685811769024*sin(2.0*t3 - 2.0*t1 + 2.0*t4) + 0.000091647786458333338043685811769024*sin(2.0*t1 + 2.0*t3 + 2.0*t4) + 0.001729949218750000095815716472103*sin(2.0*t2 + 2.0*t3 + 2.0*t4) + 0.00054988671875000002826211487061414*sin(4.0*t2 + 2.0*t3 + 2.0*t4) - 0.00036659114583333335217474324707609*sin(4.0*t2 - 1.0*t1 + 2.0*t3 + 2.0*t4) - 0.00028832486979166668263595274535049*sin(2.0*t2 - 2.0*t1 + 2.0*t3 + 2.0*t4) - 0.00028832486979166668263595274535049*sin(2.0*t1 + 2.0*t2 + 2.0*t3 + 2.0*t4) + 0.00036659114583333335217474324707609*sin(2.0*t2 - 2.0*t1 + 4.0*t3 + 2.0*t4) + 0.000091647786458333338043685811769024*sin(4.0*t2 - 2.0*t1 + 2.0*t3 + 2.0*t4) + 0.000091647786458333338043685811769024*sin(2.0*t1 + 4.0*t2 + 2.0*t3 + 2.0*t4) + 0.00036659114583333335217474324707609*sin(t1 + 2.0*t3 + 2.0*t4) - 0.00036659114583333335217474324707609*sin(t1 + 4.0*t2 + 2.0*t3 + 2.0*t4) + 0.00054988671875000002826211487061414*sin(2.0*t3 + 2.0*t4)) - 1.0*td1*(0.00036659114583333335217474324707609*sin(3.0*t2 - 1.0*t1 + t3 + t4) - 0.00073318229166666670434948649415219*sin(t2 - 2.0*t1 + 3.0*t3 + t4) - 0.00018329557291666667608737162353805*sin(3.0*t2 - 2.0*t1 + t3 + t4) - 0.00018329557291666667608737162353805*sin(2.0*t1 + 3.0*t2 + t3 + t4) + 0.00073318229166666670434948649415219*sin(t2 + t3 + t4) - 0.00036659114583333335217474324707609*sin(t1 - 1.0*t2 + t3 + t4) + 0.00057664973958333336527190549070099*sin(t2 - 2.0*t1 + t3 + t4) + 0.00057664973958333336527190549070099*sin(2.0*t1 + t2 + t3 + t4) + 0.00036659114583333335217474324707609*sin(t1 + 3.0*t2 + t3 + t4) + 0.00018329557291666667608737162353805*sin(2.0*t1 + t2 - 1.0*t3 - 1.0*t4) - 0.00036659114583333335217474324707609*sin(t3 - 1.0*t2 + t4) + 0.00036659114583333335217474324707609*sin(t1 + t2 - 1.0*t3 - 1.0*t4) - 0.00073318229166666670434948649415219*sin(2.0*t1 + t2 - 1.0*t3 + t4) - 0.00018329557291666667608737162353805*sin(2.0*t1 - 1.0*t2 + t3 + t4) - 0.00036659114583333335217474324707609*sin(3.0*t2 + t3 + t4) + 0.29875*L3^2*sin(t2 + t3 + t4) + 0.149375*L3^2*sin(t2 + t3 + t4 - 2.0*t5) + 0.149375*L3^2*sin(t2 + t3 + t4 + 2.0*t5) + 83.94875*L3*sin(t2 + t3 + t4 + t5) + 83.94875*L3*sin(t2 + t3 + t4 - 1.0*t5)) + td3*(112.33*L3*sin(t4 - 1.0*t5) - 0.00073318229166666670434948649415219*sin(2.0*t1 + t2 - 1.0*t3 + t4) - 0.00073318229166666670434948649415219*sin(t2 - 2.0*t1 + 3.0*t3 + t4) + 112.33*L3*sin(t4 + t5) + 224.66*L3*cos(t5)*sin(t4) + 0.5975*L3^2*cos(t5)*sin(t5)) - 1.0*td6*(0.00042011718750000002619432448724979*sin(t5) + 0.00042011718750000002619432448724979*cos(t1)^2*sin(t5) + 0.00063017578125000003929148673087468*cos(2.0*t2)*cos(2.0*t3)*cos(2.0*t4)*sin(t5) - 0.00063017578125000003929148673087468*cos(2.0*t2)*sin(2.0*t3)*sin(2.0*t4)*sin(t5) - 0.00063017578125000003929148673087468*cos(2.0*t3)*sin(2.0*t2)*sin(2.0*t4)*sin(t5) - 0.00063017578125000003929148673087468*cos(2.0*t4)*sin(2.0*t2)*sin(2.0*t3)*sin(t5) - 0.00021005859375000001309716224362489*cos(2.0*t1)*cos(2.0*t2)*cos(2.0*t3)*cos(2.0*t4)*sin(t5) + 0.00021005859375000001309716224362489*cos(2.0*t1)*cos(2.0*t2)*sin(2.0*t3)*sin(2.0*t4)*sin(t5) + 0.00021005859375000001309716224362489*cos(2.0*t1)*cos(2.0*t3)*sin(2.0*t2)*sin(2.0*t4)*sin(t5) + 0.00021005859375000001309716224362489*cos(2.0*t1)*cos(2.0*t4)*sin(2.0*t2)*sin(2.0*t3)*sin(t5) - 0.00021005859375000001309716224362489*sin(2.0*t1)*cos(t2)*cos(t3)*cos(t4)*cos(t5) + 0.00021005859375000001309716224362489*sin(2.0*t1)*cos(t2)*cos(t5)*sin(t3)*sin(t4) + 0.00021005859375000001309716224362489*sin(2.0*t1)*cos(t3)*cos(t5)*sin(t2)*sin(t4) + 0.00021005859375000001309716224362489*sin(2.0*t1)*cos(t4)*cos(t5)*sin(t2)*sin(t3) + 0.00042011718750000002619432448724979*cos(t1)*cos(t2)*cos(t3)*cos(t4)*cos(t5)*sin(t1) - 0.00042011718750000002619432448724979*cos(t1)*cos(t2)*cos(t5)*sin(t1)*sin(t3)*sin(t4) - 0.00042011718750000002619432448724979*cos(t1)*cos(t3)*cos(t5)*sin(t1)*sin(t2)*sin(t4) - 0.00042011718750000002619432448724979*cos(t1)*cos(t4)*cos(t5)*sin(t1)*sin(t2)*sin(t3)) + 0.29875*L3^2*td4*sin(2.0*t5)) + td2*(td4*(0.00018329557291666667608737162353805*sin(3.0*t2 - 2.0*t1 + t3 + t4) - 0.00036659114583333335217474324707609*sin(3.0*t2 - 1.0*t1 + t3 + t4) - 0.00018329557291666667608737162353805*sin(2.0*t1 + 3.0*t2 + t3 + t4) + 0.00036659114583333335217474324707609*sin(t1 - 1.0*t2 + t3 + t4) + 0.00036659114583333335217474324707609*sin(t1 + 3.0*t2 + t3 + t4) + 0.00018329557291666667608737162353805*sin(2.0*t1 + t2 - 1.0*t3 - 1.0*t4) + 0.00036659114583333335217474324707609*sin(t1 + t2 - 1.0*t3 - 1.0*t4) + 0.00018329557291666667608737162353805*sin(2.0*t1 - 1.0*t2 + t3 + t4) - 112.33*L3*sin(t4 - 1.0*t5) - 112.33*L3*sin(t4 + t5) - 121.89*L3*sin(t3 + t4 - 1.0*t5) - 121.89*L3*sin(t3 + t4 + t5) + 224.66*L3*cos(t5)*sin(t4) + 0.5975*L3^2*cos(t5)*sin(t5) + 243.78*L3*cos(t3)*cos(t5)*sin(t4) + 243.78*L3*cos(t4)*cos(t5)*sin(t3)) + td3*(0.00018329557291666667608737162353805*sin(3.0*t2 - 2.0*t1 + t3 + t4) - 0.00073318229166666670434948649415219*sin(t2 - 2.0*t1 + 3.0*t3 + t4) - 0.00036659114583333335217474324707609*sin(3.0*t2 - 1.0*t1 + t3 + t4) - 0.00018329557291666667608737162353805*sin(2.0*t1 + 3.0*t2 + t3 + t4) + 0.00036659114583333335217474324707609*sin(t1 - 1.0*t2 + t3 + t4) + 0.00036659114583333335217474324707609*sin(t1 + 3.0*t2 + t3 + t4) + 0.00018329557291666667608737162353805*sin(2.0*t1 + t2 - 1.0*t3 - 1.0*t4) + 0.00036659114583333335217474324707609*sin(t1 + t2 - 1.0*t3 - 1.0*t4) - 0.00073318229166666670434948649415219*sin(2.0*t1 + t2 - 1.0*t3 + t4) + 0.00018329557291666667608737162353805*sin(2.0*t1 - 1.0*t2 + t3 + t4) - 121.89*L3*sin(t3 + t4 - 1.0*t5) - 121.89*L3*sin(t3 + t4 + t5) + 449.32*L3*cos(t5)*sin(t4) + 0.5975*L3^2*cos(t5)*sin(t5) + 243.78*L3*cos(t3)*cos(t5)*sin(t4) + 243.78*L3*cos(t4)*cos(t5)*sin(t3)) - 1.0*td1*(0.00073318229166666670434948649415219*sin(3.0*t2 - 1.0*t1 + t3 + t4) - 0.00073318229166666670434948649415219*sin(t2 - 2.0*t1 + 3.0*t3 + t4) - 0.00018329557291666667608737162353805*sin(3.0*t2 - 2.0*t1 + t3 + t4) - 0.00018329557291666667608737162353805*sin(2.0*t1 + 3.0*t2 + t3 + t4) + 0.00073318229166666670434948649415219*sin(t2 + t3 + t4) + 0.00057664973958333336527190549070099*sin(t2 - 2.0*t1 + t3 + t4) + 0.00057664973958333336527190549070099*sin(2.0*t1 + t2 + t3 + t4) + 0.00073318229166666670434948649415219*sin(t1 + 3.0*t2 + t3 + t4) + 0.00018329557291666667608737162353805*sin(2.0*t1 + t2 - 1.0*t3 - 1.0*t4) + 0.00036659114583333335217474324707609*sin(t3 - 1.0*t2 + t4) - 0.00073318229166666670434948649415219*sin(2.0*t1 + t2 - 1.0*t3 + t4) - 0.00018329557291666667608737162353805*sin(2.0*t1 - 1.0*t2 + t3 + t4) - 0.0010997734375000000565242297412283*sin(3.0*t2 + t3 + t4) + 0.29875*L3^2*sin(t2 + t3 + t4) + 0.149375*L3^2*sin(t2 + t3 + t4 - 2.0*t5) + 0.149375*L3^2*sin(t2 + t3 + t4 + 2.0*t5) + 83.94875*L3*sin(t2 + t3 + t4 + t5) + 83.94875*L3*sin(t2 + t3 + t4 - 1.0*t5)) + td2*(449.32*L3*cos(t5)*sin(t4) + 0.5975*L3^2*cos(t5)*sin(t5) + 487.56*L3*cos(t3)*cos(t5)*sin(t4) + 487.56*L3*cos(t4)*cos(t5)*sin(t3)) + td5*(0.00036659114583333335217474324707609*sin(2.0*t1 + 2.0*t2 + 2.0*t4) + 0.001729949218750000095815716472103*sin(2.0*t2 + 2.0*t3 + 2.0*t4) + 0.0010997734375000000565242297412283*sin(4.0*t2 + 2.0*t3 + 2.0*t4) - 0.00073318229166666670434948649415219*sin(4.0*t2 - 1.0*t1 + 2.0*t3 + 2.0*t4) - 0.00028832486979166668263595274535049*sin(2.0*t2 - 2.0*t1 + 2.0*t3 + 2.0*t4) - 0.00028832486979166668263595274535049*sin(2.0*t1 + 2.0*t2 + 2.0*t3 + 2.0*t4) + 0.00036659114583333335217474324707609*sin(2.0*t2 - 2.0*t1 + 4.0*t3 + 2.0*t4) + 0.00018329557291666667608737162353805*sin(4.0*t2 - 2.0*t1 + 2.0*t3 + 2.0*t4) + 0.00018329557291666667608737162353805*sin(2.0*t1 + 4.0*t2 + 2.0*t3 + 2.0*t4) - 0.00073318229166666670434948649415219*sin(t1 + 4.0*t2 + 2.0*t3 + 2.0*t4) + 0.00036659114583333335217474324707609*sin(2.0*t2) + 0.00018329557291666667608737162353805*sin(2.0*t1 - 2.0*t2) - 0.00018329557291666667608737162353805*sin(2.0*t1 + 2.0*t2)) - 1.0*td6*(0.00042011718750000002619432448724979*sin(t5) + 0.00042011718750000002619432448724979*cos(t1)^2*sin(t5) + 0.00063017578125000003929148673087468*cos(2.0*t2)*cos(2.0*t3)*cos(2.0*t4)*sin(t5) - 0.00063017578125000003929148673087468*cos(2.0*t2)*sin(2.0*t3)*sin(2.0*t4)*sin(t5) - 0.00063017578125000003929148673087468*cos(2.0*t3)*sin(2.0*t2)*sin(2.0*t4)*sin(t5) - 0.00063017578125000003929148673087468*cos(2.0*t4)*sin(2.0*t2)*sin(2.0*t3)*sin(t5) - 0.00021005859375000001309716224362489*cos(2.0*t1)*cos(2.0*t2)*cos(2.0*t3)*cos(2.0*t4)*sin(t5) + 0.00021005859375000001309716224362489*cos(2.0*t1)*cos(2.0*t2)*sin(2.0*t3)*sin(2.0*t4)*sin(t5) + 0.00021005859375000001309716224362489*cos(2.0*t1)*cos(2.0*t3)*sin(2.0*t2)*sin(2.0*t4)*sin(t5) + 0.00021005859375000001309716224362489*cos(2.0*t1)*cos(2.0*t4)*sin(2.0*t2)*sin(2.0*t3)*sin(t5) - 0.00021005859375000001309716224362489*sin(2.0*t1)*cos(t2)*cos(t3)*cos(t4)*cos(t5) + 0.00021005859375000001309716224362489*sin(2.0*t1)*cos(t2)*cos(t5)*sin(t3)*sin(t4) + 0.00021005859375000001309716224362489*sin(2.0*t1)*cos(t3)*cos(t5)*sin(t2)*sin(t4) + 0.00021005859375000001309716224362489*sin(2.0*t1)*cos(t4)*cos(t5)*sin(t2)*sin(t3) + 0.00042011718750000002619432448724979*cos(t1)*cos(t2)*cos(t3)*cos(t4)*cos(t5)*sin(t1) - 0.00042011718750000002619432448724979*cos(t1)*cos(t2)*cos(t5)*sin(t1)*sin(t3)*sin(t4) - 0.00042011718750000002619432448724979*cos(t1)*cos(t3)*cos(t5)*sin(t1)*sin(t2)*sin(t4) - 0.00042011718750000002619432448724979*cos(t1)*cos(t4)*cos(t5)*sin(t1)*sin(t2)*sin(t3))) + td6*(td6*(0.5*(0.0016804687500000001047772979489991*cos(t1)*cos(t5) - 0.0016804687500000001047772979489991*cos(t2)*cos(t3)*cos(t4)*sin(t1)*sin(t5) + 0.0016804687500000001047772979489991*cos(t2)*sin(t1)*sin(t3)*sin(t4)*sin(t5) + 0.0016804687500000001047772979489991*cos(t3)*sin(t1)*sin(t2)*sin(t4)*sin(t5) + 0.0016804687500000001047772979489991*cos(t4)*sin(t1)*sin(t2)*sin(t3)*sin(t5))*(cos(t2)*cos(t5)*sin(t1)*sin(t3)*sin(t4) - 1.0*cos(t2)*cos(t3)*cos(t4)*cos(t5)*sin(t1) - 1.0*cos(t1)*sin(t5) + cos(t3)*cos(t5)*sin(t1)*sin(t2)*sin(t4) + cos(t4)*cos(t5)*sin(t1)*sin(t2)*sin(t3)) + 0.5*(sin(t1)*sin(t5) - 1.0*cos(t1)*cos(t2)*cos(t3)*cos(t4)*cos(t5) + cos(t1)*cos(t2)*cos(t5)*sin(t3)*sin(t4) + cos(t1)*cos(t3)*cos(t5)*sin(t2)*sin(t4) + cos(t1)*cos(t4)*cos(t5)*sin(t2)*sin(t3))*(0.00084023437500000005238864897449957*cos(t1)*cos(t2)*sin(t3)*sin(t4)*sin(t5) - 0.00084023437500000005238864897449957*cos(t1)*cos(t2)*cos(t3)*cos(t4)*sin(t5) - 0.00084023437500000005238864897449957*cos(t5)*sin(t1) + 0.00084023437500000005238864897449957*cos(t1)*cos(t3)*sin(t2)*sin(t4)*sin(t5) + 0.00084023437500000005238864897449957*cos(t1)*cos(t4)*sin(t2)*sin(t3)*sin(t5)) + 0.5*(0.00084023437500000005238864897449957*sin(t1)*sin(t5) - 0.00084023437500000005238864897449957*cos(t1)*cos(t2)*cos(t3)*cos(t4)*cos(t5) + 0.00084023437500000005238864897449957*cos(t1)*cos(t2)*cos(t5)*sin(t3)*sin(t4) + 0.00084023437500000005238864897449957*cos(t1)*cos(t3)*cos(t5)*sin(t2)*sin(t4) + 0.00084023437500000005238864897449957*cos(t1)*cos(t4)*cos(t5)*sin(t2)*sin(t3))*(cos(t1)*cos(t2)*sin(t3)*sin(t4)*sin(t5) - 1.0*cos(t1)*cos(t2)*cos(t3)*cos(t4)*sin(t5) - 1.0*cos(t5)*sin(t1) + cos(t1)*cos(t3)*sin(t2)*sin(t4)*sin(t5) + cos(t1)*cos(t4)*sin(t2)*sin(t3)*sin(t5)) + 0.5*(0.0016804687500000001047772979489991*cos(t2)*cos(t5)*sin(t1)*sin(t3)*sin(t4) - 0.0016804687500000001047772979489991*cos(t2)*cos(t3)*cos(t4)*cos(t5)*sin(t1) - 0.0016804687500000001047772979489991*cos(t1)*sin(t5) + 0.0016804687500000001047772979489991*cos(t3)*cos(t5)*sin(t1)*sin(t2)*sin(t4) + 0.0016804687500000001047772979489991*cos(t4)*cos(t5)*sin(t1)*sin(t2)*sin(t3))*(cos(t1)*cos(t5) - 1.0*cos(t2)*cos(t3)*cos(t4)*sin(t1)*sin(t5) + cos(t2)*sin(t1)*sin(t3)*sin(t4)*sin(t5) + cos(t3)*sin(t1)*sin(t2)*sin(t4)*sin(t5) + cos(t4)*sin(t1)*sin(t2)*sin(t3)*sin(t5))) + 1.0*td1*(0.00021005859375000001309716224362489*cos(2.0*t2)*cos(2.0*t3)*sin(2.0*t1)*sin(2.0*t4)*sin(t5) + 0.00021005859375000001309716224362489*cos(2.0*t2)*cos(2.0*t4)*sin(2.0*t1)*sin(2.0*t3)*sin(t5) + 0.00021005859375000001309716224362489*cos(2.0*t3)*cos(2.0*t4)*sin(2.0*t1)*sin(2.0*t2)*sin(t5) - 0.00042011718750000002619432448724979*cos(2.0*t1)*cos(t2)*cos(t3)*cos(t5)*sin(t4) - 0.00042011718750000002619432448724979*cos(2.0*t1)*cos(t2)*cos(t4)*cos(t5)*sin(t3) - 0.00042011718750000002619432448724979*cos(2.0*t1)*cos(t3)*cos(t4)*cos(t5)*sin(t2) - 0.00021005859375000001309716224362489*sin(2.0*t1)*sin(2.0*t2)*sin(2.0*t3)*sin(2.0*t4)*sin(t5) + 0.00042011718750000002619432448724979*cos(2.0*t1)*cos(t5)*sin(t2)*sin(t3)*sin(t4)) + td2*(0.00063017578125000003929148673087468*cos(2.0*t2)*cos(2.0*t3)*cos(2.0*t4)*sin(t5) - 0.00042011718750000002619432448724979*cos(t1)^2*sin(t5) - 0.00042011718750000002619432448724979*sin(t5) - 0.00063017578125000003929148673087468*cos(2.0*t2)*sin(2.0*t3)*sin(2.0*t4)*sin(t5) - 0.00063017578125000003929148673087468*cos(2.0*t3)*sin(2.0*t2)*sin(2.0*t4)*sin(t5) - 0.00063017578125000003929148673087468*cos(2.0*t4)*sin(2.0*t2)*sin(2.0*t3)*sin(t5) - 0.00021005859375000001309716224362489*cos(2.0*t1)*cos(2.0*t2)*cos(2.0*t3)*cos(2.0*t4)*sin(t5) + 0.00021005859375000001309716224362489*cos(2.0*t1)*cos(2.0*t2)*sin(2.0*t3)*sin(2.0*t4)*sin(t5) + 0.00021005859375000001309716224362489*cos(2.0*t1)*cos(2.0*t3)*sin(2.0*t2)*sin(2.0*t4)*sin(t5) + 0.00021005859375000001309716224362489*cos(2.0*t1)*cos(2.0*t4)*sin(2.0*t2)*sin(2.0*t3)*sin(t5) - 0.00021005859375000001309716224362489*sin(2.0*t1)*cos(t2)*cos(t3)*cos(t4)*cos(t5) + 0.00021005859375000001309716224362489*sin(2.0*t1)*cos(t2)*cos(t5)*sin(t3)*sin(t4) + 0.00021005859375000001309716224362489*sin(2.0*t1)*cos(t3)*cos(t5)*sin(t2)*sin(t4) + 0.00021005859375000001309716224362489*sin(2.0*t1)*cos(t4)*cos(t5)*sin(t2)*sin(t3) - 0.00042011718750000002619432448724979*cos(t1)*cos(t2)*cos(t3)*cos(t4)*cos(t5)*sin(t1) + 0.00042011718750000002619432448724979*cos(t1)*cos(t2)*cos(t5)*sin(t1)*sin(t3)*sin(t4) + 0.00042011718750000002619432448724979*cos(t1)*cos(t3)*cos(t5)*sin(t1)*sin(t2)*sin(t4) + 0.00042011718750000002619432448724979*cos(t1)*cos(t4)*cos(t5)*sin(t1)*sin(t2)*sin(t3)) + td3*(0.00063017578125000003929148673087468*cos(2.0*t2)*cos(2.0*t3)*cos(2.0*t4)*sin(t5) - 0.00042011718750000002619432448724979*cos(t1)^2*sin(t5) - 0.00042011718750000002619432448724979*sin(t5) - 0.00063017578125000003929148673087468*cos(2.0*t2)*sin(2.0*t3)*sin(2.0*t4)*sin(t5) - 0.00063017578125000003929148673087468*cos(2.0*t3)*sin(2.0*t2)*sin(2.0*t4)*sin(t5) - 0.00063017578125000003929148673087468*cos(2.0*t4)*sin(2.0*t2)*sin(2.0*t3)*sin(t5) - 0.00021005859375000001309716224362489*cos(2.0*t1)*cos(2.0*t2)*cos(2.0*t3)*cos(2.0*t4)*sin(t5) + 0.00021005859375000001309716224362489*cos(2.0*t1)*cos(2.0*t2)*sin(2.0*t3)*sin(2.0*t4)*sin(t5) + 0.00021005859375000001309716224362489*cos(2.0*t1)*cos(2.0*t3)*sin(2.0*t2)*sin(2.0*t4)*sin(t5) + 0.00021005859375000001309716224362489*cos(2.0*t1)*cos(2.0*t4)*sin(2.0*t2)*sin(2.0*t3)*sin(t5) - 0.00021005859375000001309716224362489*sin(2.0*t1)*cos(t2)*cos(t3)*cos(t4)*cos(t5) + 0.00021005859375000001309716224362489*sin(2.0*t1)*cos(t2)*cos(t5)*sin(t3)*sin(t4) + 0.00021005859375000001309716224362489*sin(2.0*t1)*cos(t3)*cos(t5)*sin(t2)*sin(t4) + 0.00021005859375000001309716224362489*sin(2.0*t1)*cos(t4)*cos(t5)*sin(t2)*sin(t3) - 0.00042011718750000002619432448724979*cos(t1)*cos(t2)*cos(t3)*cos(t4)*cos(t5)*sin(t1) + 0.00042011718750000002619432448724979*cos(t1)*cos(t2)*cos(t5)*sin(t1)*sin(t3)*sin(t4) + 0.00042011718750000002619432448724979*cos(t1)*cos(t3)*cos(t5)*sin(t1)*sin(t2)*sin(t4) + 0.00042011718750000002619432448724979*cos(t1)*cos(t4)*cos(t5)*sin(t1)*sin(t2)*sin(t3)) + td4*(0.00063017578125000003929148673087468*cos(2.0*t2)*cos(2.0*t3)*cos(2.0*t4)*sin(t5) - 0.00042011718750000002619432448724979*cos(t1)^2*sin(t5) - 0.00042011718750000002619432448724979*sin(t5) - 0.00063017578125000003929148673087468*cos(2.0*t2)*sin(2.0*t3)*sin(2.0*t4)*sin(t5) - 0.00063017578125000003929148673087468*cos(2.0*t3)*sin(2.0*t2)*sin(2.0*t4)*sin(t5) - 0.00063017578125000003929148673087468*cos(2.0*t4)*sin(2.0*t2)*sin(2.0*t3)*sin(t5) - 0.00021005859375000001309716224362489*cos(2.0*t1)*cos(2.0*t2)*cos(2.0*t3)*cos(2.0*t4)*sin(t5) + 0.00021005859375000001309716224362489*cos(2.0*t1)*cos(2.0*t2)*sin(2.0*t3)*sin(2.0*t4)*sin(t5) + 0.00021005859375000001309716224362489*cos(2.0*t1)*cos(2.0*t3)*sin(2.0*t2)*sin(2.0*t4)*sin(t5) + 0.00021005859375000001309716224362489*cos(2.0*t1)*cos(2.0*t4)*sin(2.0*t2)*sin(2.0*t3)*sin(t5) - 0.00021005859375000001309716224362489*sin(2.0*t1)*cos(t2)*cos(t3)*cos(t4)*cos(t5) + 0.00021005859375000001309716224362489*sin(2.0*t1)*cos(t2)*cos(t5)*sin(t3)*sin(t4) + 0.00021005859375000001309716224362489*sin(2.0*t1)*cos(t3)*cos(t5)*sin(t2)*sin(t4) + 0.00021005859375000001309716224362489*sin(2.0*t1)*cos(t4)*cos(t5)*sin(t2)*sin(t3) - 0.00042011718750000002619432448724979*cos(t1)*cos(t2)*cos(t3)*cos(t4)*cos(t5)*sin(t1) + 0.00042011718750000002619432448724979*cos(t1)*cos(t2)*cos(t5)*sin(t1)*sin(t3)*sin(t4) + 0.00042011718750000002619432448724979*cos(t1)*cos(t3)*cos(t5)*sin(t1)*sin(t2)*sin(t4) + 0.00042011718750000002619432448724979*cos(t1)*cos(t4)*cos(t5)*sin(t1)*sin(t2)*sin(t3))) - td1*(1.0*td3*(0.00073318229166666670434948649415219*sin(t2 - 2.0*t1 + 3.0*t3 + t4) - 0.00036659114583333335217474324707609*sin(3.0*t2 - 1.0*t1 + t3 + t4) + 0.00018329557291666667608737162353805*sin(3.0*t2 - 2.0*t1 + t3 + t4) + 0.00018329557291666667608737162353805*sin(2.0*t1 + 3.0*t2 + t3 + t4) - 0.00073318229166666670434948649415219*sin(t2 + t3 + t4) + 0.00036659114583333335217474324707609*sin(t1 - 1.0*t2 + t3 + t4) - 0.00057664973958333336527190549070099*sin(t2 - 2.0*t1 + t3 + t4) - 0.00057664973958333336527190549070099*sin(2.0*t1 + t2 + t3 + t4) - 0.00036659114583333335217474324707609*sin(t1 + 3.0*t2 + t3 + t4) - 0.00018329557291666667608737162353805*sin(2.0*t1 + t2 - 1.0*t3 - 1.0*t4) + 0.00036659114583333335217474324707609*sin(t3 - 1.0*t2 + t4) - 0.00036659114583333335217474324707609*sin(t1 + t2 - 1.0*t3 - 1.0*t4) + 0.00073318229166666670434948649415219*sin(2.0*t1 + t2 - 1.0*t3 + t4) + 0.00018329557291666667608737162353805*sin(2.0*t1 - 1.0*t2 + t3 + t4) + 0.00036659114583333335217474324707609*sin(3.0*t2 + t3 + t4) - 0.29875*L3^2*sin(t2 + t3 + t4) + 0.149375*L3^2*sin(t2 + t3 + t4 - 2.0*t5) + 0.149375*L3^2*sin(t2 + t3 + t4 + 2.0*t5) - 61.24375*L3*sin(t2 + t3 + t4 + t5) + 224.66*L3*sin(t2 + t3 - 1.0*t5) - 224.66*L3*sin(t2 + t3 + t5) + 61.24375*L3*sin(t2 + t3 + t4 - 1.0*t5) - 0.5975*L3*L4*sin(t2 + t3 + t4 - 1.0*t5) + 0.5975*L3*L4*sin(t2 + t3 + t4 + t5)) + 1.0*td5*(0.00018329557291666667608737162353805*sin(2.0*t3 - 1.0*t1 + 2.0*t4) - 0.00036659114583333335217474324707609*sin(2.0*t1 + 2.0*t2 + 2.0*t4) + 0.000091647786458333338043685811769024*sin(2.0*t3 - 2.0*t1 + 2.0*t4) - 0.000091647786458333338043685811769024*sin(2.0*t1 + 2.0*t3 + 2.0*t4) - 0.00018329557291666667608737162353805*sin(4.0*t2 - 1.0*t1 + 2.0*t3 + 2.0*t4) - 0.00028832486979166668263595274535049*sin(2.0*t2 - 2.0*t1 + 2.0*t3 + 2.0*t4) + 0.00028832486979166668263595274535049*sin(2.0*t1 + 2.0*t2 + 2.0*t3 + 2.0*t4) + 0.00036659114583333335217474324707609*sin(2.0*t2 - 2.0*t1 + 4.0*t3 + 2.0*t4) + 0.000091647786458333338043685811769024*sin(4.0*t2 - 2.0*t1 + 2.0*t3 + 2.0*t4) - 0.000091647786458333338043685811769024*sin(2.0*t1 + 4.0*t2 + 2.0*t3 + 2.0*t4) - 0.00018329557291666667608737162353805*sin(t1 + 2.0*t3 + 2.0*t4) + 0.00018329557291666667608737162353805*sin(t1 + 4.0*t2 + 2.0*t3 + 2.0*t4) - 0.00057664973958333336527190549070099*sin(2.0*t1) + 0.00018329557291666667608737162353805*sin(2.0*t1 - 2.0*t2) + 0.00018329557291666667608737162353805*sin(2.0*t1 + 2.0*t2) + 0.00073318229166666670434948649415219*sin(2.0*t1 - 2.0*t3)) + 1.0*td1*(0.0746875*L3^2*sin(2.0*t2 + 2.0*t3 + 2.0*t4 - 2.0*t5) - 112.33*L3*sin(t4 - 1.0*t5) - 0.0746875*L3^2*sin(2.0*t2 + 2.0*t3 + 2.0*t4 + 2.0*t5) + 112.33*L3*sin(2.0*t2 + 2.0*t3 + t4 - 1.0*t5) + 30.621875*L3*sin(2.0*t2 + 2.0*t3 + 2.0*t4 + t5) - 112.33*L3*sin(t4 + t5) - 121.89*L3*sin(t3 + t4 - 1.0*t5) + 121.89*L3*sin(2.0*t2 + t3 + t4 - 1.0*t5) + 112.33*L3*sin(2.0*t2 + 2.0*t3 + t4 + t5) + 0.149375*L3^2*sin(2.0*t5) + 167.8975*L3*sin(t5) + 30.621875*L3*sin(2.0*t2 + 2.0*t3 + 2.0*t4 - 1.0*t5) - 121.89*L3*sin(t3 + t4 + t5) + 121.89*L3*sin(2.0*t2 + t3 + t4 + t5) - 0.29875*L3*L4*sin(2.0*t2 + 2.0*t3 + 2.0*t4 - 1.0*t5) - 0.29875*L3*L4*sin(2.0*t2 + 2.0*t3 + 2.0*t4 + t5)) - td2*(0.00073318229166666670434948649415219*sin(3.0*t2 - 1.0*t1 + t3 + t4) - 0.00073318229166666670434948649415219*sin(t2 - 2.0*t1 + 3.0*t3 + t4) - 0.00018329557291666667608737162353805*sin(3.0*t2 - 2.0*t1 + t3 + t4) - 0.00018329557291666667608737162353805*sin(2.0*t1 + 3.0*t2 + t3 + t4) + 0.00073318229166666670434948649415219*sin(t2 + t3 + t4) + 0.00057664973958333336527190549070099*sin(t2 - 2.0*t1 + t3 + t4) + 0.00057664973958333336527190549070099*sin(2.0*t1 + t2 + t3 + t4) + 0.00073318229166666670434948649415219*sin(t1 + 3.0*t2 + t3 + t4) + 0.00018329557291666667608737162353805*sin(2.0*t1 + t2 - 1.0*t3 - 1.0*t4) + 0.00036659114583333335217474324707609*sin(t3 - 1.0*t2 + t4) - 0.00073318229166666670434948649415219*sin(2.0*t1 + t2 - 1.0*t3 + t4) - 0.00018329557291666667608737162353805*sin(2.0*t1 - 1.0*t2 + t3 + t4) - 0.0010997734375000000565242297412283*sin(3.0*t2 + t3 + t4) - 243.78*L3*sin(t2 - 1.0*t5) + 0.29875*L3^2*sin(t2 + t3 + t4) - 0.149375*L3^2*sin(t2 + t3 + t4 - 2.0*t5) - 0.149375*L3^2*sin(t2 + t3 + t4 + 2.0*t5) + 61.24375*L3*sin(t2 + t3 + t4 + t5) + 243.78*L3*sin(t2 + t5) - 224.66*L3*sin(t2 + t3 - 1.0*t5) + 224.66*L3*sin(t2 + t3 + t5) - 61.24375*L3*sin(t2 + t3 + t4 - 1.0*t5) + 0.5975*L3*L4*sin(t2 + t3 + t4 - 1.0*t5) - 0.5975*L3*L4*sin(t2 + t3 + t4 + t5)) + 1.0*td4*(0.00073318229166666670434948649415219*sin(t2 - 2.0*t1 + 3.0*t3 + t4) - 0.00036659114583333335217474324707609*sin(3.0*t2 - 1.0*t1 + t3 + t4) + 0.00018329557291666667608737162353805*sin(3.0*t2 - 2.0*t1 + t3 + t4) + 0.00018329557291666667608737162353805*sin(2.0*t1 + 3.0*t2 + t3 + t4) - 0.00073318229166666670434948649415219*sin(t2 + t3 + t4) + 0.00036659114583333335217474324707609*sin(t1 - 1.0*t2 + t3 + t4) - 0.00057664973958333336527190549070099*sin(t2 - 2.0*t1 + t3 + t4) - 0.00057664973958333336527190549070099*sin(2.0*t1 + t2 + t3 + t4) - 0.00036659114583333335217474324707609*sin(t1 + 3.0*t2 + t3 + t4) - 0.00018329557291666667608737162353805*sin(2.0*t1 + t2 - 1.0*t3 - 1.0*t4) + 0.00036659114583333335217474324707609*sin(t3 - 1.0*t2 + t4) - 0.00036659114583333335217474324707609*sin(t1 + t2 - 1.0*t3 - 1.0*t4) + 0.00073318229166666670434948649415219*sin(2.0*t1 + t2 - 1.0*t3 + t4) + 0.00018329557291666667608737162353805*sin(2.0*t1 - 1.0*t2 + t3 + t4) + 0.00036659114583333335217474324707609*sin(3.0*t2 + t3 + t4) - 0.29875*L3^2*sin(t2 + t3 + t4) + 0.149375*L3^2*sin(t2 + t3 + t4 - 2.0*t5) + 0.149375*L3^2*sin(t2 + t3 + t4 + 2.0*t5) - 61.24375*L3*sin(t2 + t3 + t4 + t5) + 61.24375*L3*sin(t2 + t3 + t4 - 1.0*t5) - 0.5975*L3*L4*sin(t2 + t3 + t4 - 1.0*t5) + 0.5975*L3*L4*sin(t2 + t3 + t4 + t5)) + td6*(0.00021005859375000001309716224362489*cos(2.0*t2)*cos(2.0*t3)*sin(2.0*t1)*sin(2.0*t4)*sin(t5) + 0.00021005859375000001309716224362489*cos(2.0*t2)*cos(2.0*t4)*sin(2.0*t1)*sin(2.0*t3)*sin(t5) + 0.00021005859375000001309716224362489*cos(2.0*t3)*cos(2.0*t4)*sin(2.0*t1)*sin(2.0*t2)*sin(t5) - 0.00042011718750000002619432448724979*cos(2.0*t1)*cos(t2)*cos(t3)*cos(t5)*sin(t4) - 0.00042011718750000002619432448724979*cos(2.0*t1)*cos(t2)*cos(t4)*cos(t5)*sin(t3) - 0.00042011718750000002619432448724979*cos(2.0*t1)*cos(t3)*cos(t4)*cos(t5)*sin(t2) - 0.00021005859375000001309716224362489*sin(2.0*t1)*sin(2.0*t2)*sin(2.0*t3)*sin(2.0*t4)*sin(t5) + 0.00042011718750000002619432448724979*cos(2.0*t1)*cos(t5)*sin(t2)*sin(t3)*sin(t4)))
